simulink model "DYN_02x"  (R2021a)
(part 22 of 53)

(sin(e5)*(cos(e1)*cos(e2)*cos(e3) - cos(e1)*sin(e2)*sin(e3)) + cos(e5)*(sin(e1)*sin(e4) + cos(e4)*(cos(e1)*cos(e2)*sin(e3) + cos(e1)*cos(e3)*sin(e2))))*(z5*(cos(e2 + e3)*cos(e5) - sin(e2 + e3)*cos(e4)*sin(e5)) - y5*sin(e2 + e3)*sin(e4) + cos(e5)*sin(e4)*(a3*cos(e2 + e3) - d4*sin(e2 + e3) + a2*cos(e2))) - (cos(e5)*(cos(e1)*cos(e2)*cos(e3) - cos(e1)*sin(e2)*sin(e3)) - sin(e5)*(sin(e1)*sin(e4) + cos(e4)*(cos(e1)*cos(e2)*sin(e3) + cos(e1)*cos(e3)*sin(e2))))*(z5*(cos(e2 + e3)*sin(e5) + sin(e2 + e3)*cos(e4)*cos(e5)) - x5*sin(e2 + e3)*sin(e4) + sin(e4)*sin(e5)*(a3*cos(e2 + e3) - d4*sin(e2 + e3) + a2*cos(e2))) - (sin(e5)*(cos(e1)*cos(e2)*sin(e3) + cos(e1)*cos(e3)*sin(e2)) - cos(e4)*cos(e5)*(cos(e1)*cos(e2)*cos(e3) - cos(e1)*sin(e2)*sin(e3)))*(z5*(sin(e2 + e3)*cos(e5) + cos(e2 + e3)*cos(e4)*sin(e5)) + cos(e5)*sin(e4)*(a1 + d4*cos(e2 + e3) + a3*sin(e2 + e3) + a2*sin(e2)) + y5*cos(e2 + e3)*sin(e4)) - sin(e4)*(cos(e1)*cos(e2)*cos(e3) - cos(e1)*sin(e2)*sin(e3))*(cos(e4)*(a1 + d4*cos(e2 + e3) + a3*sin(e2 + e3) + a2*sin(e2)) + x5*(sin(e2 + e3)*cos(e5) + cos(e2 + e3)*cos(e4)*sin(e5)) - y5*(sin(e2 + e3)*sin(e5) - cos(e2 + e3)*cos(e4)*cos(e5)))) - m5*((cos(e5)*(sin(e2)*sin(e3) - cos(e2)*cos(e3)) + cos(e4)*sin(e5)*(cos(e2)*sin(e3) + cos(e3)*sin(e2)))*(a3*cos(e5) + x5*cos(e4) + d4*cos(e4)*sin(e5) + z5*cos(e5)*sin(e4)) + (sin(e5)*(sin(e2)*sin(e3) - cos(e2)*cos(e3)) - cos(e4)*cos(e5)*(cos(e2)*sin(e3) + cos(e3)*sin(e2)))*(a3*sin(e5) - y5*cos(e4) - d4*cos(e4)*cos(e5) + z5*sin(e4)*sin(e5)) + sin(e4)*(cos(e2)*sin(e3) + cos(e3)*sin(e2))*(d4*sin(e4) + y5*cos(e5)*sin(e4) + x5*sin(e4)*sin(e5)))*((cos(e5)*(cos(e2)*sin(e3) + cos(e3)*sin(e2)) - cos(e4)*sin(e5)*(sin(e2)*sin(e3) - cos(e2)*cos(e3)))*(z5*(sin(e2 + e3)*sin(e5) - cos(e2 + e3)*cos(e4)*cos(e5)) + sin(e4)*sin(e5)*(a1 + d4*cos(e2 + e3) + a3*sin(e2 + e3) + a2*sin(e2)) + x5*cos(e2 + e3)*sin(e4)) - (sin(e5)*(cos(e2)*sin(e3) + cos(e3)*sin(e2)) + cos(e4)*cos(e5)*(sin(e2)*sin(e3) - cos(e2)*cos(e3)))*(z5*(sin(e2 + e3)*cos(e5) + cos(e2 + e3)*cos(e4)*sin(e5)) + cos(e5)*sin(e4)*(a1 + d4*cos(e2 + e3) + a3*sin(e2 + e3) + a2*sin(e2)) + y5*cos(e2 + e3)*sin(e4)) + sin(e4)*(sin(e2)*sin(e3) - cos(e2)*cos(e3))*(cos(e4)*(a1 + d4*cos(e2 + e3) + a3*sin(e2 + e3) + a2*sin(e2)) + x5*(sin(e2 + e3)*cos(e5) + cos(e2 + e3)*cos(e4)*sin(e5)) - y5*(sin(e2 + e3)*sin(e5) - cos(e2 + e3)*cos(e4)*cos(e5)))) - (sin(e4)*sin(e5)*(I5xy*(cos(e2 + e3)*sin(e5) + sin(e2 + e3)*cos(e4)*cos(e5)) + I5yy*(cos(e2 + e3)*cos(e5) - sin(e2 + e3)*cos(e4)*sin(e5)) + I5zy*sin(e2 + e3)*sin(e4)))/2 + m5*((cos(e4)*sin(e1) - sin(e4)*(cos(e1)*cos(e2)*sin(e3) + cos(e1)*cos(e3)*sin(e2)))*(cos(e4)*(a1 + d4*cos(e2 + e3) + a3*sin(e2 + e3) + a2*sin(e2)) + x5*(sin(e2 + e3)*cos(e5) + cos(e2 + e3)*cos(e4)*sin(e5)) - y5*(sin(e2 + e3)*sin(e5) - cos(e2 + e3)*cos(e4)*cos(e5))) + (sin(e5)*(cos(e1)*cos(e2)*cos(e3) - cos(e1)*sin(e2)*sin(e3)) + cos(e5)*(sin(e1)*sin(e4) + cos(e4)*(cos(e1)*cos(e2)*sin(e3) + cos(e1)*cos(e3)*sin(e2))))*(z5*(sin(e2 + e3)*cos(e5) + cos(e2 + e3)*cos(e4)*sin(e5)) + cos(e5)*sin(e4)*(a1 + d4*cos(e2 + e3) + a3*sin(e2 + e3) + a2*sin(e2)) + y5*cos(e2 + e3)*sin(e4)) - (cos(e5)*(cos(e1)*cos(e2)*cos(e3) - cos(e1)*sin(e2)*sin(e3)) - sin(e5)*(sin(e1)*sin(e4) + cos(e4)*(cos(e1)*cos(e2)*sin(e3) + cos(e1)*cos(e3)*sin(e2))))*(z5*(sin(e2 + e3)*sin(e5) - cos(e2 + e3)*cos(e4)*cos(e5)) + sin(e4)*sin(e5)*(a1 + d4*cos(e2 + e3) + a3*sin(e2 + e3) + a2*sin(e2)) + x5*cos(e2 + e3)*sin(e4)))*((cos(e5)*(cos(e1)*cos(e2)*sin(e3) + cos(e1)*cos(e3)*sin(e2)) + cos(e4)*sin(e5)*(cos(e1)*cos(e2)*cos(e3) - cos(e1)*sin(e2)*sin(e3)))*(a3*cos(e5) + x5*cos(e4) + d4*cos(e4)*sin(e5) + z5*cos(e5)*sin(e4)) + (sin(e5)*(cos(e1)*cos(e2)*sin(e3) + cos(e1)*cos(e3)*sin(e2)) - cos(e4)*cos(e5)*(cos(e1)*cos(e2)*cos(e3) - cos(e1)*sin(e2)*sin(e3)))*(a3*sin(e5) - y5*cos(e4) - d4*cos(e4)*cos(e5) + z5*sin(e4)*sin(e5)) + sin(e4)*(cos(e1)*cos(e2)*cos(e3) - cos(e1)*sin(e2)*sin(e3))*(d4*sin(e4) + y5*cos(e5)*sin(e4) + x5*sin(e4)*sin(e5))) - (sin(e2 + e3)*sin(e4)*(I5zz*cos(e4) - I5xz*cos(e5)*sin(e4) + I5yz*sin(e4)*sin(e5)))/2 + m4*(cos(e4)*(sin(e2)*sin(e3) - cos(e2)*cos(e3))*(d4*cos(e4) + z4*cos(e4)) - (cos(e2)*sin(e3) + cos(e3)*sin(e2))*(a3 + x4*cos(e4) - y4*sin(e4)) + sin(e4)*(sin(e2)*sin(e3) - cos(e2)*cos(e3))*(d4*sin(e4) + z4*sin(e4)))*((sin(e2)*sin(e3) - cos(e2)*cos(e3))*(y4*cos(e2 + e3)*cos(e4) + x4*cos(e2 + e3)*sin(e4)) + (cos(e2)*sin(e3) + cos(e3)*sin(e2))*(y4*sin(e2 + e3)*cos(e4) + x4*sin(e2 + e3)*sin(e4)) - sin(e4)*(sin(e2)*sin(e3) - cos(e2)*cos(e3))*(x4*cos(e2 + e3) + cos(e4)*(a3*cos(e2 + e3) - d4*sin(e2 + e3) + a2*cos(e2)) - z4*sin(e2 + e3)*cos(e4)) - cos(e4)*(sin(e2)*sin(e3) - cos(e2)*cos(e3))*(y4*cos(e2 + e3) - sin(e4)*(a3*cos(e2 + e3) - d4*sin(e2 + e3) + a2*cos(e2)) + z4*sin(e2 + e3)*sin(e4)) - sin(e4)*(cos(e2)*sin(e3) + cos(e3)*sin(e2))*(cos(e4)*(a1 + d4*cos(e2 + e3) + a3*sin(e2 + e3) + a2*sin(e2)) + x4*sin(e2 + e3) + z4*cos(e2 + e3)*cos(e4)) + cos(e4)*(cos(e2)*sin(e3) + cos(e3)*sin(e2))*(sin(e4)*(a1 + d4*cos(e2 + e3) + a3*sin(e2 + e3) + a2*sin(e2)) - y4*sin(e2 + e3) + z4*cos(e2 + e3)*sin(e4))) - m5*((cos(e5)*(cos(e2)*sin(e1)*sin(e3) + cos(e3)*sin(e1)*sin(e2)) + cos(e4)*sin(e5)*(cos(e2)*cos(e3)*sin(e1) - sin(e1)*sin(e2)*sin(e3)))*(a3*cos(e5) + x5*cos(e4) + d4*cos(e4)*sin(e5) + z5*cos(e5)*sin(e4)) + (sin(e5)*(cos(e2)*sin(e1)*sin(e3) + cos(e3)*sin(e1)*sin(e2)) - cos(e4)*cos(e5)*(cos(e2)*cos(e3)*sin(e1) - sin(e1)*sin(e2)*sin(e3)))*(a3*sin(e5) - y5*cos(e4) - d4*cos(e4)*cos(e5) + z5*sin(e4)*sin(e5)) + sin(e4)*(cos(e2)*cos(e3)*sin(e1) - sin(e1)*sin(e2)*sin(e3))*(d4*sin(e4) + y5*cos(e5)*sin(e4) + x5*sin(e4)*sin(e5)))*((cos(e5)*(cos(e2)*cos(e3)*sin(e1) - sin(e1)*sin(e2)*sin(e3)) + sin(e5)*(cos(e1)*sin(e4) - cos(e4)*(cos(e2)*sin(e1)*sin(e3) + cos(e3)*sin(e1)*sin(e2))))*(z5*(sin(e2 + e3)*sin(e5) - cos(e2 + e3)*cos(e4)*cos(e5)) + sin(e4)*sin(e5)*(a1 + d4*cos(e2 + e3) + a3*sin(e2 + e3) + a2*sin(e2)) + x5*cos(e2 + e3)*sin(e4)) + (sin(e4)*(cos(e2)*sin(e1)*sin(e3) + cos(e3)*sin(e1)*sin(e2)) + cos(e1)*cos(e4))*(cos(e4)*(a1 + d4*cos(e2 + e3) + a3*sin(e2 + e3) + a2*sin(e2)) + x5*(sin(e2 + e3)*cos(e5) + cos(e2 + e3)*cos(e4)*sin(e5)) - y5*(sin(e2 + e3)*sin(e5) - cos(e2 + e3)*cos(e4)*cos(e5))) - (sin(e5)*(cos(e2)*cos(e3)*sin(e1) - sin(e1)*sin(e2)*sin(e3)) - cos(e5)*(cos(e1)*sin(e4) - cos(e4)*(cos(e2)*sin(e1)*sin(e3) + cos(e3)*sin(e1)*sin(e2))))*(z5*(sin(e2 + e3)*cos(e5) + cos(e2 + e3)*cos(e4)*sin(e5)) + cos(e5)*sin(e4)*(a1 + d4*cos(e2 + e3) + a3*sin(e2 + e3) + a2*sin(e2)) + y5*cos(e2 + e3)*sin(e4))) + m6*((sin(e6)*(sin(e5)*(cos(e2)*cos(e3)*sin(e1) - sin(e1)*sin(e2)*sin(e3)) - cos(e5)*(cos(e1)*sin(e4) - cos(e4)*(cos(e2)*sin(e1)*sin(e3) + cos(e3)*sin(e1)*sin(e2)))) + cos(e6)*(sin(e4)*(cos(e2)*sin(e1)*sin(e3) + cos(e3)*sin(e1)*sin(e2)) + cos(e1)*cos(e4)))*(z6*(cos(e4)*sin(e6) + cos(e5)*cos(e6)*sin(e4)) - sin(e6)*(a3*sin(e5) - d4*cos(e4)*cos(e5)) + d4*cos(e6)*sin(e4) + x6*sin(e4)*sin(e5)) - (cos(e5)*(cos(e2)*cos(e3)*sin(e1) - sin(e1)*sin(e2)*sin(e3)) + sin(e5)*(cos(e1)*sin(e4) - cos(e4)*(cos(e2)*sin(e1)*sin(e3) + cos(e3)*sin(e1)*sin(e2))))*(a3*cos(e5) - y6*(cos(e4)*sin(e6) + cos(e5)*cos(e6)*sin(e4)) + x6*(cos(e4)*cos(e6) - cos(e5)*sin(e4)*sin(e6)) + d4*cos(e4)*sin(e5)) + (cos(e6)*(sin(e5)*(cos(e2)*cos(e3)*sin(e1) - sin(e1)*sin(e2)*sin(e3)) - cos(e5)*(cos(e1)*sin(e4) - cos(e4)*(cos(e2)*sin(e1)*sin(e3) + cos(e3)*sin(e1)*sin(e2)))) - sin(e6)*(sin(e4)*(cos(e2)*sin(e1)*sin(e3) + cos(e3)*sin(e1)*sin(e2)) + cos(e1)*cos(e4)))*(z6*(cos(e4)*cos(e6) - cos(e5)*sin(e4)*sin(e6)) - cos(e6)*(a3*sin(e5) - d4*cos(e4)*cos(e5)) - d4*sin(e4)*sin(e6) + y6*sin(e4)*sin(e5)))*((sin(e6)*(sin(e5)*(cos(e2)*sin(e1)*sin(e3) + cos(e3)*sin(e1)*sin(e2)) - cos(e4)*cos(e5)*(cos(e2)*cos(e3)*sin(e1) - sin(e1)*sin(e2)*sin(e3))) - cos(e6)*sin(e4)*(cos(e2)*cos(e3)*sin(e1) - sin(e1)*sin(e2)*sin(e3)))*(x6*(sin(e2 + e3)*cos(e5) + cos(e2 + e3)*cos(e4)*sin(e5)) - z6*(cos(e6)*(sin(e2 + e3)*sin(e5) - cos(e2 + e3)*cos(e4)*cos(e5)) + cos(e2 + e3)*sin(e4)*sin(e6)) + cos(e4)*cos(e6)*(a1 + d4*cos(e2 + e3) + a3*sin(e2 + e3) + a2*sin(e2)) - cos(e5)*sin(e4)*sin(e6)*(a1 + d4*cos(e2 + e3) + a3*sin(e2 + e3) + a2*sin(e2))) + (cos(e6)*(sin(e5)*(cos(e2)*sin(e1)*sin(e3) + cos(e3)*sin(e1)*sin(e2)) - cos(e4)*cos(e5)*(cos(e2)*cos(e3)*sin(e1) - sin(e1)*sin(e2)*sin(e3))) + sin(e4)*sin(e6)*(cos(e2)*cos(e3)*sin(e1) - sin(e1)*sin(e2)*sin(e3)))*(y6*(sin(e2 + e3)*cos(e5) + cos(e2 + e3)*cos(e4)*sin(e5)) + z6*(sin(e6)*(sin(e2 + e3)*sin(e5) - cos(e2 + e3)*cos(e4)*cos(e5)) - cos(e2 + e3)*cos(e6)*sin(e4)) - cos(e4)*sin(e6)*(a1 + d4*cos(e2 + e3) + a3*sin(e2 + e3) + a2*sin(e2)) - cos(e5)*cos(e6)*sin(e4)*(a1 + d4*cos(e2 + e3) + a3*sin(e2 + e3) + a2*sin(e2))) + (cos(e5)*(cos(e2)*cos(e3)*sin(e1) - sin(e1)*sin(e2)*sin(e3)) + sin(e5)*(cos(e1)*sin(e4) - cos(e4)*(cos(e2)*sin(e1)*sin(e3) + cos(e3)*sin(e1)*sin(e2))))*(x6*(sin(e6)*(cos(e2 + e3)*sin(e5) + sin(e2 + e3)*cos(e4)*cos(e5)) + sin(e2 + e3)*cos(e6)*sin(e4)) + y6*(cos(e6)*(cos(e2 + e3)*sin(e5) + sin(e2 + e3)*cos(e4)*cos(e5)) - sin(e2 + e3)*sin(e4)*sin(e6)) - sin(e4)*sin(e5)*(a3*cos(e2 + e3) - d4*sin(e2 + e3) + a2*cos(e2))) - (sin(e6)*(sin(e5)*(cos(e2)*cos(e3)*sin(e1) - sin(e1)*sin(e2)*sin(e3)) - cos(e5)*(cos(e1)*sin(e4) - cos(e4)*(cos(e2)*sin(e1)*sin(e3) + cos(e3)*sin(e1)*sin(e2)))) + cos(e6)*(sin(e4)*(cos(e2)*sin(e1)*sin(e3) + cos(e3)*sin(e1)*sin(e2)) + cos(e1)*cos(e4)))*(x6*(cos(e2 + e3)*cos(e5) - sin(e2 + e3)*cos(e4)*sin(e5)) - z6*(cos(e6)*(cos(e2 + e3)*sin(e5) + sin(e2 + e3)*cos(e4)*cos(e5)) - sin(e2 + e3)*sin(e4)*sin(e6)) + cos(e4)*cos(e6)*(a3*cos(e2 + e3) - d4*sin(e2 + e3) + a2*cos(e2)) - cos(e5)*sin(e4)*sin(e6)*(a3*cos(e2 + e3) - d4*sin(e2 + e3) + a2*cos(e2))) - (cos(e6)*(sin(e5)*(cos(e2)*cos(e3)*sin(e1) - sin(e1)*sin(e2)*sin(e3)) - cos(e5)*(cos(e1)*sin(e4) - cos(e4)*(cos(e2)*sin(e1)*sin(e3) + cos(e3)*sin(e1)*sin(e2)))) - sin(e6)*(sin(e4)*(cos(e2)*sin(e1)*sin(e3) + cos(e3)*sin(e1)*sin(e2)) + cos(e1)*cos(e4)))*(y6*(cos(e2 + e3)*cos(e5) - sin(e2 + e3)*cos(e4)*sin(e5)) + z6*(sin(e6)*(cos(e2 + e3)*sin(e5) + sin(e2 + e3)*cos(e4)*cos(e5)) + sin(e2 + e3)*cos(e6)*sin(e4)) - cos(e4)*sin(e6)*(a3*cos(e2 + e3) - d4*sin(e2 + e3) + a2*cos(e2)) - cos(e5)*cos(e6)*sin(e4)*(a3*cos(e2 + e3) - d4*sin(e2 + e3) + a2*cos(e2))) - (cos(e5)*(cos(e2)*sin(e1)*sin(e3) + cos(e3)*sin(e1)*sin(e2)) + cos(e4)*sin(e5)*(cos(e2)*cos(e3)*sin(e1) - sin(e1)*sin(e2)*sin(e3)))*(x6*(sin(e6)*(sin(e2 + e3)*sin(e5) - cos(e2 + e3)*cos(e4)*cos(e5)) - cos(e2 + e3)*cos(e6)*sin(e4)) + y6*(cos(e6)*(sin(e2 + e3)*sin(e5) - cos(e2 + e3)*cos(e4)*cos(e5)) + cos(e2 + e3)*sin(e4)*sin(e6)) - sin(e4)*sin(e5)*(a1 + d4*cos(e2 + e3) + a3*sin(e2 + e3) + a2*sin(e2)))) - m4*((cos(e2)*cos(e3)*sin(e1) - sin(e1)*sin(e2)*sin(e3))*(a3 + x4*cos(e4) - y4*sin(e4)) + (d4*cos(e4) + z4*cos(e4))*(cos(e1)*sin(e4) - cos(e4)*(cos(e2)*sin(e1)*sin(e3) + cos(e3)*sin(e1)*sin(e2))) - (sin(e4)*(cos(e2)*sin(e1)*sin(e3) + cos(e3)*sin(e1)*sin(e2)) + cos(e1)*cos(e4))*(d4*sin(e4) + z4*sin(e4)))*((cos(e2)*sin(e1)*sin(e3) + cos(e3)*sin(e1)*sin(e2))*(y4*cos(e2 + e3)*cos(e4) + x4*cos(e2 + e3)*sin(e4)) + (cos(e2)*cos(e3)*sin(e1) - sin(e1)*sin(e2)*sin(e3))*(y4*sin(e2 + e3)*cos(e4) + x4*sin(e2 + e3)*sin(e4)) - (sin(e4)*(cos(e2)*sin(e1)*sin(e3) + cos(e3)*sin(e1)*sin(e2)) + cos(e1)*cos(e4))*(x4*cos(e2 + e3) + cos(e4)*(a3*cos(e2 + e3) - d4*sin(e2 + e3) + a2*cos(e2)) - z4*sin(e2 + e3)*cos(e4)) + (cos(e1)*sin(e4) - cos(e4)*(cos(e2)*sin(e1)*sin(e3) + cos(e3)*sin(e1)*sin(e2)))*(y4*cos(e2 + e3) - sin(e4)*(a3*cos(e2 + e3) - d4*sin(e2 + e3) + a2*cos(e2)) + z4*sin(e2 + e3)*sin(e4)) - sin(e4)*(cos(e2)*cos(e3)*sin(e1) - sin(e1)*sin(e2)*sin(e3))*(cos(e4)*(a1 + d4*cos(e2 + e3) + a3*sin(e2 + e3) + a2*sin(e2)) + x4*sin(e2 + e3) + z4*cos(e2 + e3)*cos(e4)) + cos(e4)*(cos(e2)*cos(e3)*sin(e1) - sin(e1)*sin(e2)*sin(e3))*(sin(e4)*(a1 + d4*cos(e2 + e3) + a3*sin(e2 + e3) + a2*sin(e2)) - y4*sin(e2 + e3) + z4*cos(e2 + e3)*sin(e4))) - m4*((sin(e4)*(cos(e2)*sin(e1)*sin(e3) + cos(e3)*sin(e1)*sin(e2)) + cos(e1)*cos(e4))*(cos(e4)*(a1 + d4*cos(e2 + e3) + a3*sin(e2 + e3) + a2*sin(e2)) + x4*sin(e2 + e3) + z4*cos(e2 + e3)*cos(e4)) + (cos(e2)*cos(e3)*sin(e1) - sin(e1)*sin(e2)*sin(e3))*(y4*cos(e2 + e3)*cos(e4) + x4*cos(e2 + e3)*sin(e4)) + (cos(e1)*sin(e4) - cos(e4)*(cos(e2)*sin(e1)*sin(e3) + cos(e3)*sin(e1)*sin(e2)))*(sin(e4)*(a1 + d4*cos(e2 + e3) + a3*sin(e2 + e3) + a2*sin(e2)) - y4*sin(e2 + e3) + z4*cos(e2 + e3)*sin(e4)))*((cos(e2)*sin(e1)*sin(e3) + cos(e3)*sin(e1)*sin(e2))*(a3 + x4*cos(e4) - y4*sin(e4)) + cos(e4)*(cos(e2)*cos(e3)*sin(e1) - sin(e1)*sin(e2)*sin(e3))*(d4*cos(e4) + z4*cos(e4)) + sin(e4)*(cos(e2)*cos(e3)*sin(e1) - sin(e1)*sin(e2)*sin(e3))*(d4*sin(e4) + z4*sin(e4))) - m4*((cos(e1)*cos(e2)*cos(e3) - cos(e1)*sin(e2)*sin(e3))*(a3 + x4*cos(e4) - y4*sin(e4)) - (sin(e1)*sin(e4) + cos(e4)*(cos(e1)*cos(e2)*sin(e3) + cos(e1)*cos(e3)*sin(e2)))*(d4*cos(e4) + z4*cos(e4)) + (cos(e4)*sin(e1) - sin(e4)*(cos(e1)*cos(e2)*sin(e3) + cos(e1)*cos(e3)*sin(e2)))*(d4*sin(e4) + z4*sin(e4)))*((y4*cos(e2 + e3)*cos(e4) + x4*cos(e2 + e3)*sin(e4))*(cos(e1)*cos(e2)*sin(e3) + cos(e1)*cos(e3)*sin(e2)) + (y4*sin(e2 + e3)*cos(e4) + x4*sin(e2 + e3)*sin(e4))*(cos(e1)*cos(e2)*cos(e3) - cos(e1)*sin(e2)*sin(e3)) + (cos(e4)*sin(e1) - sin(e4)*(cos(e1)*cos(e2)*sin(e3) + cos(e1)*cos(e3)*sin(e2)))*(x4*cos(e2 + e3) + cos(e4)*(a3*cos(e2 + e3) - d4*sin(e2 + e3) + a2*cos(e2)) - z4*sin(e2 + e3)*cos(e4)) - (sin(e1)*sin(e4) + cos(e4)*(cos(e1)*cos(e2)*sin(e3) + cos(e1)*cos(e3)*sin(e2)))*(y4*cos(e2 + e3) - sin(e4)*(a3*cos(e2 + e3) - d4*sin(e2 + e3) + a2*cos(e2)) + z4*sin(e2 + e3)*sin(e4)) - sin(e4)*(cos(e1)*cos(e2)*cos(e3) - cos(e1)*sin(e2)*sin(e3))*(cos(e4)*(a1 + d4*cos(e2 + e3) + a3*sin(e2 + e3) + a2*sin(e2)) + x4*sin(e2 + e3) + z4*cos(e2 + e3)*cos(e4)) + cos(e4)*(cos(e1)*cos(e2)*cos(e3) - cos(e1)*sin(e2)*sin(e3))*(sin(e4)*(a1 + d4*cos(e2 + e3) + a3*sin(e2 + e3) + a2*sin(e2)) - y4*sin(e2 + e3) + z4*cos(e2 + e3)*sin(e4))) + m3*(y3*cos(e2 + e3)*cos(e1) + x3*sin(e2 + e3)*cos(e1))*(sin(e1)*(a1 + y3*cos(e2 + e3) + x3*sin(e2 + e3) + a2*sin(e2)) + z3*cos(e2 + e3)^2*cos(e1) + z3*sin(e2 + e3)^2*cos(e1)) + m6*((sin(e6)*(sin(e5)*(cos(e2)*sin(e3) + cos(e3)*sin(e2)) + cos(e4)*cos(e5)*(sin(e2)*sin(e3) - cos(e2)*cos(e3))) + cos(e6)*sin(e4)*(sin(e2)*sin(e3) - cos(e2)*cos(e3)))*(z6*(cos(e4)*sin(e6) + cos(e5)*cos(e6)*sin(e4)) - sin(e6)*(a3*sin(e5) - d4*cos(e4)*cos(e5)) + d4*cos(e6)*sin(e4) + x6*sin(e4)*sin(e5)) + (cos(e6)*(sin(e5)*(cos(e2)*sin(e3) + cos(e3)*sin(e2)) + cos(e4)*cos(e5)*(sin(e2)*sin(e3) - cos(e2)*cos(e3))) - sin(e4)*sin(e6)*(sin(e2)*sin(e3) - cos(e2)*cos(e3)))*(z6*(cos(e4)*cos(e6) - cos(e5)*sin(e4)*sin(e6)) - cos(e6)*(a3*sin(e5) - d4*cos(e4)*cos(e5)) - d4*sin(e4)*sin(e6) + y6*sin(e4)*sin(e5)) - (cos(e5)*(cos(e2)*sin(e3) + cos(e3)*sin(e2)) - cos(e4)*sin(e5)*(sin(e2)*sin(e3) - cos(e2)*cos(e3)))*(a3*cos(e5) - y6*(cos(e4)*sin(e6) + cos(e5)*cos(e6)*sin(e4)) + x6*(cos(e4)*cos(e6) - cos(e5)*sin(e4)*sin(e6)) + d4*cos(e4)*sin(e5)))*((sin(e6)*(sin(e5)*(sin(e2)*sin(e3) - cos(e2)*cos(e3)) - cos(e4)*cos(e5)*(cos(e2)*sin(e3) + cos(e3)*sin(e2))) - cos(e6)*sin(e4)*(cos(e2)*sin(e3) + cos(e3)*sin(e2)))*(x6*(sin(e2 + e3)*cos(e5) + cos(e2 + e3)*cos(e4)*sin(e5)) - z6*(cos(e6)*(sin(e2 + e3)*sin(e5) - cos(e2 + e3)*cos(e4)*cos(e5)) + cos(e2 + e3)*sin(e4)*sin(e6)) + cos(e4)*cos(e6)*(a1 + d4*cos(e2 + e3) + a3*sin(e2 + e3) + a2*sin(e2)) - cos(e5)*sin(e4)*sin(e6)*(a1 + d4*cos(e2 + e3) + a3*sin(e2 + e3) + a2*sin(e2))) + (cos(e6)*(sin(e5)*(sin(e2)*sin(e3) - cos(e2)*cos(e3)) - cos(e4)*cos(e5)*(cos(e2)*sin(e3) + cos(e3)*sin(e2))) + sin(e4)*sin(e6)*(cos(e2)*sin(e3) + cos(e3)*sin(e2)))*(y6*(sin(e2 + e3)*cos(e5) + cos(e2 + e3)*cos(e4)*sin(e5)) + z6*(sin(e6)*(sin(e2 + e3)*sin(e5) - cos(e2 + e3)*cos(e4)*cos(e5)) - cos(e2 + e3)*cos(e6)*sin(e4)) - cos(e4)*sin(e6)*(a1 + d4*cos(e2 + e3) + a3*sin(e2 + e3) + a2*sin(e2)) - cos(e5)*cos(e6)*sin(e4)*(a1 + d4*cos(e2 + e3) + a3*sin(e2 + e3) + a2*sin(e2))) + (cos(e5)*(cos(e2)*sin(e3) + cos(e3)*sin(e2)) - cos(e4)*sin(e5)*(sin(e2)*sin(e3) - cos(e2)*cos(e3)))*(x6*(sin(e6)*(cos(e2 + e3)*sin(e5) + sin(e2 + e3)*cos(e4)*cos(e5)) + sin(e2 + e3)*cos(e6)*sin(e4)) + y6*(cos(e6)*(cos(e2 + e3)*sin(e5) + sin(e2 + e3)*cos(e4)*cos(e5)) - sin(e2 + e3)*sin(e4)*sin(e6)) - sin(e4)*sin(e5)*(a3*cos(e2 + e3) - d4*sin(e2 + e3) + a2*cos(e2))) - (sin(e6)*(sin(e5)*(cos(e2)*sin(e3) + cos(e3)*sin(e2)) + cos(e4)*cos(e5)*(sin(e2)*sin(e3) - cos(e2)*cos(e3))) + cos(e6)*sin(e4)*(sin(e2)*sin(e3) - cos(e2)*cos(e3)))*(x6*(cos(e2 + e3)*cos(e5) - sin(e2 + e3)*cos(e4)*sin(e5)) - z6*(cos(e6)*(cos(e2 + e3)*sin(e5) + sin(e2 + e3)*cos(e4)*cos(e5)) - sin(e2 + e3)*sin(e4)*sin(e6)) + cos(e4)*cos(e6)*(a3*cos(e2 + e3) - d4*sin(e2 + e3) + a2*cos(e2)) - cos(e5)*sin(e4)*sin(e6)*(a3*cos(e2 + e3) - d4*sin(e2 + e3) + a2*cos(e2))) - (cos(e6)*(sin(e5)*(cos(e2)*sin(e3) + cos(e3)*sin(e2)) + cos(e4)*cos(e5)*(sin(e2)*sin(e3) - cos(e2)*cos(e3))) - sin(e4)*sin(e6)*(sin(e2)*sin(e3) - cos(e2)*cos(e3)))*(y6*(cos(e2 + e3)*cos(e5) - sin(e2 + e3)*cos(e4)*sin(e5)) + z6*(sin(e6)*(cos(e2 + e3)*sin(e5) + sin(e2 + e3)*cos(e4)*cos(e5)) + sin(e2 + e3)*cos(e6)*sin(e4)) - cos(e4)*sin(e6)*(a3*cos(e2 + e3) - d4*sin(e2 + e3) + a2*cos(e2)) - cos(e5)*cos(e6)*sin(e4)*(a3*cos(e2 + e3) - d4*sin(e2 + e3) + a2*cos(e2))) - (cos(e5)*(sin(e2)*sin(e3) - cos(e2)*cos(e3)) + cos(e4)*sin(e5)*(cos(e2)*sin(e3) + cos(e3)*sin(e2)))*(x6*(sin(e6)*(sin(e2 + e3)*sin(e5) - cos(e2 + e3)*cos(e4)*cos(e5)) - cos(e2 + e3)*cos(e6)*sin(e4)) + y6*(cos(e6)*(sin(e2 + e3)*sin(e5) - cos(e2 + e3)*cos(e4)*cos(e5)) + cos(e2 + e3)*sin(e4)*sin(e6)) - sin(e4)*sin(e5)*(a1 + d4*cos(e2 + e3) + a3*sin(e2 + e3) + a2*sin(e2)))) + m6*((sin(e6)*(sin(e5)*(cos(e2)*cos(e3)*sin(e1) - sin(e1)*sin(e2)*sin(e3)) - cos(e5)*(cos(e1)*sin(e4) - cos(e4)*(cos(e2)*sin(e1)*sin(e3) + cos(e3)*sin(e1)*sin(e2)))) + cos(e6)*(sin(e4)*(cos(e2)*sin(e1)*sin(e3) + cos(e3)*sin(e1)*sin(e2)) + cos(e1)*cos(e4)))*(x6*(sin(e2 + e3)*cos(e5) + cos(e2 + e3)*cos(e4)*sin(e5)) - z6*(cos(e6)*(sin(e2 + e3)*sin(e5) - cos(e2 + e3)*cos(e4)*cos(e5)) + cos(e2 + e3)*sin(e4)*sin(e6)) + cos(e4)*cos(e6)*(a1 + d4*cos(e2 + e3) + a3*sin(e2 + e3) + a2*sin(e2)) - cos(e5)*sin(e4)*sin(e6)*(a1 + d4*cos(e2 + e3) + a3*sin(e2 + e3) + a2*sin(e2))) + (cos(e6)*(sin(e5)*(cos(e2)*cos(e3)*sin(e1) - sin(e1)*sin(e2)*sin(e3)) - cos(e5)*(cos(e1)*sin(e4) - cos(e4)*(cos(e2)*sin(e1)*sin(e3) + cos(e3)*sin(e1)*sin(e2)))) - sin(e6)*(sin(e4)*(cos(e2)*sin(e1)*sin(e3) + cos(e3)*sin(e1)*sin(e2)) + cos(e1)*cos(e4)))*(y6*(sin(e2 + e3)*cos(e5) + cos(e2 + e3)*cos(e4)*sin(e5)) + z6*(sin(e6)*(sin(e2 + e3)*sin(e5) - cos(e2 + e3)*cos(e4)*cos(e5)) - cos(e2 + e3)*cos(e6)*sin(e4)) - cos(e4)*sin(e6)*(a1 + d4*cos(e2 + e3) + a3*sin(e2 + e3) + a2*sin(e2)) - cos(e5)*cos(e6)*sin(e4)*(a1 + d4*cos(e2 + e3) + a3*sin(e2 + e3) + a2*sin(e2))) - (cos(e5)*(cos(e2)*cos(e3)*sin(e1) - sin(e1)*sin(e2)*sin(e3)) + sin(e5)*(cos(e1)*sin(e4) - cos(e4)*(cos(e2)*sin(e1)*sin(e3) + cos(e3)*sin(e1)*sin(e2))))*(x6*(sin(e6)*(sin(e2 + e3)*sin(e5) - cos(e2 + e3)*cos(e4)*cos(e5)) - cos(e2 + e3)*cos(e6)*sin(e4)) + y6*(cos(e6)*(sin(e2 + e3)*sin(e5) - cos(e2 + e3)*cos(e4)*cos(e5)) + cos(e2 + e3)*sin(e4)*sin(e6)) - sin(e4)*sin(e5)*(a1 + d4*cos(e2 + e3) + a3*sin(e2 + e3) + a2*sin(e2))))*((sin(e6)*(sin(e5)*(cos(e2)*sin(e1)*sin(e3) + cos(e3)*sin(e1)*sin(e2)) - cos(e4)*cos(e5)*(cos(e2)*cos(e3)*sin(e1) - sin(e1)*sin(e2)*sin(e3))) - cos(e6)*sin(e4)*(cos(e2)*cos(e3)*sin(e1) - sin(e1)*sin(e2)*sin(e3)))*(z6*(cos(e4)*sin(e6) + cos(e5)*cos(e6)*sin(e4)) - sin(e6)*(a3*sin(e5) - d4*cos(e4)*cos(e5)) + d4*cos(e6)*sin(e4) + x6*sin(e4)*sin(e5)) - (cos(e5)*(cos(e2)*sin(e1)*sin(e3) + cos(e3)*sin(e1)*sin(e2)) + cos(e4)*sin(e5)*(cos(e2)*cos(e3)*sin(e1) - sin(e1)*sin(e2)*sin(e3)))*(a3*cos(e5) - y6*(cos(e4)*sin(e6) + cos(e5)*cos(e6)*sin(e4)) + x6*(cos(e4)*cos(e6) - cos(e5)*sin(e4)*sin(e6)) + d4*cos(e4)*sin(e5)) + (cos(e6)*(sin(e5)*(cos(e2)*sin(e1)*sin(e3) + cos(e3)*sin(e1)*sin(e2)) - cos(e4)*cos(e5)*(cos(e2)*cos(e3)*sin(e1) - sin(e1)*sin(e2)*sin(e3))) + sin(e4)*sin(e6)*(cos(e2)*cos(e3)*sin(e1) - sin(e1)*sin(e2)*sin(e3)))*(z6*(cos(e4)*cos(e6) - cos(e5)*sin(e4)*sin(e6)) - cos(e6)*(a3*sin(e5) - d4*cos(e4)*cos(e5)) - d4*sin(e4)*sin(e6) + y6*sin(e4)*sin(e5))) + m5*((cos(e5)*(cos(e2)*cos(e3)*sin(e1) - sin(e1)*sin(e2)*sin(e3)) + sin(e5)*(cos(e1)*sin(e4) - cos(e4)*(cos(e2)*sin(e1)*sin(e3) + cos(e3)*sin(e1)*sin(e2))))*(a3*cos(e5) + x5*cos(e4) + d4*cos(e4)*sin(e5) + z5*cos(e5)*sin(e4)) + (sin(e5)*(cos(e2)*cos(e3)*sin(e1) - sin(e1)*sin(e2)*sin(e3)) - cos(e5)*(cos(e1)*sin(e4) - cos(e4)*(cos(e2)*sin(e1)*sin(e3) + cos(e3)*sin(e1)*sin(e2))))*(a3*sin(e5) - y5*cos(e4) - d4*cos(e4)*cos(e5) + z5*sin(e4)*sin(e5)) - (sin(e4)*(cos(e2)*sin(e1)*sin(e3) + cos(e3)*sin(e1)*sin(e2)) + cos(e1)*cos(e4))*(d4*sin(e4) + y5*cos(e5)*sin(e4) + x5*sin(e4)*sin(e5)))*((sin(e4)*(cos(e2)*sin(e1)*sin(e3) + cos(e3)*sin(e1)*sin(e2)) + cos(e1)*cos(e4))*(x5*(cos(e2 + e3)*cos(e5) - sin(e2 + e3)*cos(e4)*sin(e5)) - y5*(cos(e2 + e3)*sin(e5) + sin(e2 + e3)*cos(e4)*cos(e5)) + cos(e4)*(a3*cos(e2 + e3) - d4*sin(e2 + e3) + a2*cos(e2))) + (sin(e5)*(cos(e2)*sin(e1)*sin(e3) + cos(e3)*sin(e1)*sin(e2)) - cos(e4)*cos(e5)*(cos(e2)*cos(e3)*sin(e1) - sin(e1)*sin(e2)*sin(e3)))*(z5*(sin(e2 + e3)*cos(e5) + cos(e2 + e3)*cos(e4)*sin(e5)) + cos(e5)*sin(e4)*(a1 + d4*cos(e2 + e3) + a3*sin(e2 + e3) + a2*sin(e2)) + y5*cos(e2 + e3)*sin(e4)) - (cos(e5)*(cos(e2)*sin(e1)*sin(e3) + cos(e3)*sin(e1)*sin(e2)) + cos(e4)*sin(e5)*(cos(e2)*cos(e3)*sin(e1) - sin(e1)*sin(e2)*sin(e3)))*(z5*(sin(e2 + e3)*sin(e5) - cos(e2 + e3)*cos(e4)*cos(e5)) + sin(e4)*sin(e5)*(a1 + d4*cos(e2 + e3) + a3*sin(e2 + e3) + a2*sin(e2)) + x5*cos(e2 + e3)*sin(e4)) - (sin(e5)*(cos(e2)*cos(e3)*sin(e1) - sin(e1)*sin(e2)*sin(e3)) - cos(e5)*(cos(e1)*sin(e4) - cos(e4)*(cos(e2)*sin(e1)*sin(e3) + cos(e3)*sin(e1)*sin(e2))))*(z5*(cos(e2 + e3)*cos(e5) - sin(e2 + e3)*cos(e4)*sin(e5)) - y5*sin(e2 + e3)*sin(e4) + cos(e5)*sin(e4)*(a3*cos(e2 + e3) - d4*sin(e2 + e3) + a2*cos(e2))) + (cos(e5)*(cos(e2)*cos(e3)*sin(e1) - sin(e1)*sin(e2)*sin(e3)) + sin(e5)*(cos(e1)*sin(e4) - cos(e4)*(cos(e2)*sin(e1)*sin(e3) + cos(e3)*sin(e1)*sin(e2))))*(z5*(cos(e2 + e3)*sin(e5) + sin(e2 + e3)*cos(e4)*cos(e5)) - x5*sin(e2 + e3)*sin(e4) + sin(e4)*sin(e5)*(a3*cos(e2 + e3) - d4*sin(e2 + e3) + a2*cos(e2))) + sin(e4)*(cos(e2)*cos(e3)*sin(e1) - sin(e1)*sin(e2)*sin(e3))*(cos(e4)*(a1 + d4*cos(e2 + e3) + a3*sin(e2 + e3) + a2*sin(e2)) + x5*(sin(e2 + e3)*cos(e5) + cos(e2 + e3)*cos(e4)*sin(e5)) - y5*(sin(e2 + e3)*sin(e5) - cos(e2 + e3)*cos(e4)*cos(e5)))) + m3*(y3*cos(e2 + e3)*sin(e1) + x3*sin(e2 + e3)*sin(e1))*(z3*cos(e2 + e3)^2*sin(e1) - cos(e1)*(a1 + y3*cos(e2 + e3) + x3*sin(e2 + e3) + a2*sin(e2)) + z3*sin(e2 + e3)^2*sin(e1)) + m4*((cos(e1)*cos(e2)*sin(e3) + cos(e1)*cos(e3)*sin(e2))*(a3 + x4*cos(e4) - y4*sin(e4)) + cos(e4)*(d4*cos(e4) + z4*cos(e4))*(cos(e1)*cos(e2)*cos(e3) - cos(e1)*sin(e2)*sin(e3)) + sin(e4)*(d4*sin(e4) + z4*sin(e4))*(cos(e1)*cos(e2)*cos(e3) - cos(e1)*sin(e2)*sin(e3)))*((cos(e4)*sin(e1) - sin(e4)*(cos(e1)*cos(e2)*sin(e3) + cos(e1)*cos(e3)*sin(e2)))*(cos(e4)*(a1 + d4*cos(e2 + e3) + a3*sin(e2 + e3) + a2*sin(e2)) + x4*sin(e2 + e3) + z4*cos(e2 + e3)*cos(e4)) - (y4*cos(e2 + e3)*cos(e4) + x4*cos(e2 + e3)*sin(e4))*(cos(e1)*cos(e2)*cos(e3) - cos(e1)*sin(e2)*sin(e3)) + (sin(e1)*sin(e4) + cos(e4)*(cos(e1)*cos(e2)*sin(e3) + cos(e1)*cos(e3)*sin(e2)))*(sin(e4)*(a1 + d4*cos(e2 + e3) + a3*sin(e2 + e3) + a2*sin(e2)) - y4*sin(e2 + e3) + z4*cos(e2 + e3)*sin(e4))) - m4*((sin(e2)*sin(e3) - cos(e2)*cos(e3))*(a3 + x4*cos(e4) - y4*sin(e4)) + cos(e4)*(cos(e2)*sin(e3) + cos(e3)*sin(e2))*(d4*cos(e4) + z4*cos(e4)) + sin(e4)*(cos(e2)*sin(e3) + cos(e3)*sin(e2))*(d4*sin(e4) + z4*sin(e4)))*((cos(e2)*sin(e3) + cos(e3)*sin(e2))*(y4*cos(e2 + e3)*cos(e4) + x4*cos(e2 + e3)*sin(e4)) + sin(e4)*(sin(e2)*sin(e3) - cos(e2)*cos(e3))*(cos(e4)*(a1 + d4*cos(e2 + e3) + a3*sin(e2 + e3) + a2*sin(e2)) + x4*sin(e2 + e3) + z4*cos(e2 + e3)*cos(e4)) - cos(e4)*(sin(e2)*sin(e3) - cos(e2)*cos(e3))*(sin(e4)*(a1 + d4*cos(e2 + e3) + a3*sin(e2 + e3) + a2*sin(e2)) - y4*sin(e2 + e3) + z4*cos(e2 + e3)*sin(e4))) - (sin(e4)*sin(e5)*(I6zz*(cos(e2 + e3)*cos(e5) - sin(e2 + e3)*cos(e4)*sin(e5)) + I6xz*(cos(e6)*(cos(e2 + e3)*sin(e5) + sin(e2 + e3)*cos(e4)*cos(e5)) - sin(e2 + e3)*sin(e4)*sin(e6)) - I6yz*(sin(e6)*(cos(e2 + e3)*sin(e5) + sin(e2 + e3)*cos(e4)*cos(e5)) + sin(e2 + e3)*cos(e6)*sin(e4))))/2 + m6*((sin(e6)*(sin(e5)*(cos(e1)*cos(e2)*cos(e3) - cos(e1)*sin(e2)*sin(e3)) + cos(e5)*(sin(e1)*sin(e4) + cos(e4)*(cos(e1)*cos(e2)*sin(e3) + cos(e1)*cos(e3)*sin(e2)))) - cos(e6)*(cos(e4)*sin(e1) - sin(e4)*(cos(e1)*cos(e2)*sin(e3) + cos(e1)*cos(e3)*sin(e2))))*(x6*(sin(e2 + e3)*cos(e5) + cos(e2 + e3)*cos(e4)*sin(e5)) - z6*(cos(e6)*(sin(e2 + e3)*sin(e5) - cos(e2 + e3)*cos(e4)*cos(e5)) + cos(e2 + e3)*sin(e4)*sin(e6)) + cos(e4)*cos(e6)*(a1 + d4*cos(e2 + e3) + a3*sin(e2 + e3) + a2*sin(e2)) - cos(e5)*sin(e4)*sin(e6)*(a1 + d4*cos(e2 + e3) + a3*sin(e2 + e3) + a2*sin(e2))) + (cos(e6)*(sin(e5)*(cos(e1)*cos(e2)*cos(e3) - cos(e1)*sin(e2)*sin(e3)) + cos(e5)*(sin(e1)*sin(e4) + cos(e4)*(cos(e1)*cos(e2)*sin(e3) + cos(e1)*cos(e3)*sin(e2)))) + sin(e6)*(cos(e4)*sin(e1) - sin(e4)*(cos(e1)*cos(e2)*sin(e3) + cos(e1)*cos(e3)*sin(e2))))*(y6*(sin(e2 + e3)*cos(e5) + cos(e2 + e3)*cos(e4)*sin(e5)) + z6*(sin(e6)*(sin(e2 + e3)*sin(e5) - cos(e2 + e3)*cos(e4)*cos(e5)) - cos(e2 + e3)*cos(e6)*sin(e4)) - cos(e4)*sin(e6)*(a1 + d4*cos(e2 + e3) + a3*sin(e2 + e3) + a2*sin(e2)) - cos(e5)*cos(e6)*sin(e4)*(a1 + d4*cos(e2 + e3) + a3*sin(e2 + e3) + a2*sin(e2))) - (cos(e5)*(cos(e1)*cos(e2)*cos(e3) - cos(e1)*sin(e2)*sin(e3)) - sin(e5)*(sin(e1)*sin(e4) + cos(e4)*(cos(e1)*cos(e2)*sin(e3) + cos(e1)*cos(e3)*sin(e2))))*(x6*(sin(e6)*(sin(e2 + e3)*sin(e5) - cos(e2 + e3)*cos(e4)*cos(e5)) - cos(e2 + e3)*cos(e6)*sin(e4)) + y6*(cos(e6)*(sin(e2 + e3)*sin(e5) - cos(e2 + e3)*cos(e4)*cos(e5)) + cos(e2 + e3)*sin(e4)*sin(e6)) - sin(e4)*sin(e5)*(a1 + d4*cos(e2 + e3) + a3*sin(e2 + e3) + a2*sin(e2))))*((sin(e6)*(sin(e5)*(cos(e1)*cos(e2)*sin(e3) + cos(e1)*cos(e3)*sin(e2)) - cos(e4)*cos(e5)*(cos(e1)*cos(e2)*cos(e3) - cos(e1)*sin(e2)*sin(e3))) - cos(e6)*sin(e4)*(cos(e1)*cos(e2)*cos(e3) - cos(e1)*sin(e2)*sin(e3)))*(z6*(cos(e4)*sin(e6) + cos(e5)*cos(e6)*sin(e4)) - sin(e6)*(a3*sin(e5) - d4*cos(e4)*cos(e5)) + d4*cos(e6)*sin(e4) + x6*sin(e4)*sin(e5)) - (cos(e5)*(cos(e1)*cos(e2)*sin(e3) + cos(e1)*cos(e3)*sin(e2)) + cos(e4)*sin(e5)*(cos(e1)*cos(e2)*cos(e3) - cos(e1)*sin(e2)*sin(e3)))*(a3*cos(e5) - y6*(cos(e4)*sin(e6) + cos(e5)*cos(e6)*sin(e4)) + x6*(cos(e4)*cos(e6) - cos(e5)*sin(e4)*sin(e6)) + d4*cos(e4)*sin(e5)) + (cos(e6)*(sin(e5)*(cos(e1)*cos(e2)*sin(e3) + cos(e1)*cos(e3)*sin(e2)) - cos(e4)*cos(e5)*(cos(e1)*cos(e2)*cos(e3) - cos(e1)*sin(e2)*sin(e3))) + sin(e4)*sin(e6)*(cos(e1)*cos(e2)*cos(e3) - cos(e1)*sin(e2)*sin(e3)))*(z6*(cos(e4)*cos(e6) - cos(e5)*sin(e4)*sin(e6)) - cos(e6)*(a3*sin(e5) - d4*cos(e4)*cos(e5)) - d4*sin(e4)*sin(e6) + y6*sin(e4)*sin(e5))) + m6*((sin(e6)*(sin(e5)*(sin(e2)*sin(e3) - cos(e2)*cos(e3)) - cos(e4)*cos(e5)*(cos(e2)*sin(e3) + cos(e3)*sin(e2))) - cos(e6)*sin(e4)*(cos(e2)*sin(e3) + cos(e3)*sin(e2)))*(z6*(cos(e4)*sin(e6) + cos(e5)*cos(e6)*sin(e4)) - sin(e6)*(a3*sin(e5) - d4*cos(e4)*cos(e5)) + d4*cos(e6)*sin(e4) + x6*sin(e4)*sin(e5)) + (cos(e6)*(sin(e5)*(sin(e2)*sin(e3) - cos(e2)*cos(e3)) - cos(e4)*cos(e5)*(cos(e2)*sin(e3) + cos(e3)*sin(e2))) + sin(e4)*sin(e6)*(cos(e2)*sin(e3) + cos(e3)*sin(e2)))*(z6*(cos(e4)*cos(e6) - cos(e5)*sin(e4)*sin(e6)) - cos(e6)*(a3*sin(e5) - d4*cos(e4)*cos(e5)) - d4*sin(e4)*sin(e6) + y6*sin(e4)*sin(e5)) - (cos(e5)*(sin(e2)*sin(e3) - cos(e2)*cos(e3)) + cos(e4)*sin(e5)*(cos(e2)*sin(e3) + cos(e3)*sin(e2)))*(a3*cos(e5) - y6*(cos(e4)*sin(e6) + cos(e5)*cos(e6)*sin(e4)) + x6*(cos(e4)*cos(e6) - cos(e5)*sin(e4)*sin(e6)) + d4*cos(e4)*sin(e5)))*((sin(e6)*(sin(e5)*(cos(e2)*sin(e3) + cos(e3)*sin(e2)) + cos(e4)*cos(e5)*(sin(e2)*sin(e3) - cos(e2)*cos(e3))) + cos(e6)*sin(e4)*(sin(e2)*sin(e3) - cos(e2)*cos(e3)))*(x6*(sin(e2 + e3)*cos(e5) + cos(e2 + e3)*cos(e4)*sin(e5)) - z6*(cos(e6)*(sin(e2 + e3)*sin(e5) - cos(e2 + e3)*cos(e4)*cos(e5)) + cos(e2 + e3)*sin(e4)*sin(e6)) + cos(e4)*cos(e6)*(a1 + d4*cos(e2 + e3) + a3*sin(e2 + e3) + a2*sin(e2)) - cos(e5)*sin(e4)*sin(e6)*(a1 + d4*cos(e2 + e3) + a3*sin(e2 + e3) + a2*sin(e2))) + (cos(e6)*(sin(e5)*(cos(e2)*sin(e3) + cos(e3)*sin(e2)) + cos(e4)*cos(e5)*(sin(e2)*sin(e3) - cos(e2)*cos(e3))) - sin(e4)*sin(e6)*(sin(e2)*sin(e3) - cos(e2)*cos(e3)))*(y6*(sin(e2 + e3)*cos(e5) + cos(e2 + e3)*cos(e4)*sin(e5)) + z6*(sin(e6)*(sin(e2 + e3)*sin(e5) - cos(e2 + e3)*cos(e4)*cos(e5)) - cos(e2 + e3)*cos(e6)*sin(e4)) - cos(e4)*sin(e6)*(a1 + d4*cos(e2 + e3) + a3*sin(e2 + e3) + a2*sin(e2)) - cos(e5)*cos(e6)*sin(e4)*(a1 + d4*cos(e2 + e3) + a3*sin(e2 + e3) + a2*sin(e2))) - (cos(e5)*(cos(e2)*sin(e3) + cos(e3)*sin(e2)) - cos(e4)*sin(e5)*(sin(e2)*sin(e3) - cos(e2)*cos(e3)))*(x6*(sin(e6)*(sin(e2 + e3)*sin(e5) - cos(e2 + e3)*cos(e4)*cos(e5)) - cos(e2 + e3)*cos(e6)*sin(e4)) + y6*(cos(e6)*(sin(e2 + e3)*sin(e5) - cos(e2 + e3)*cos(e4)*cos(e5)) + cos(e2 + e3)*sin(e4)*sin(e6)) - sin(e4)*sin(e5)*(a1 + d4*cos(e2 + e3) + a3*sin(e2 + e3) + a2*sin(e2)))) + m6*((sin(e6)*(sin(e5)*(cos(e1)*cos(e2)*cos(e3) - cos(e1)*sin(e2)*sin(e3)) + cos(e5)*(sin(e1)*sin(e4) + cos(e4)*(cos(e1)*cos(e2)*sin(e3) + cos(e1)*cos(e3)*sin(e2)))) - cos(e6)*(cos(e4)*sin(e1) - sin(e4)*(cos(e1)*cos(e2)*sin(e3) + cos(e1)*cos(e3)*sin(e2))))*(z6*(cos(e4)*sin(e6) + cos(e5)*cos(e6)*sin(e4)) - sin(e6)*(a3*sin(e5) - d4*cos(e4)*cos(e5)) + d4*cos(e6)*sin(e4) + x6*sin(e4)*sin(e5)) + (cos(e6)*(sin(e5)*(cos(e1)*cos(e2)*cos(e3) - cos(e1)*sin(e2)*sin(e3)) + cos(e5)*(sin(e1)*sin(e4) + cos(e4)*(cos(e1)*cos(e2)*sin(e3) + cos(e1)*cos(e3)*sin(e2)))) + sin(e6)*(cos(e4)*sin(e1) - sin(e4)*(cos(e1)*cos(e2)*sin(e3) + cos(e1)*cos(e3)*sin(e2))))*(z6*(cos(e4)*cos(e6) - cos(e5)*sin(e4)*sin(e6)) - cos(e6)*(a3*sin(e5) - d4*cos(e4)*cos(e5)) - d4*sin(e4)*sin(e6) + y6*sin(e4)*sin(e5)) - (cos(e5)*(cos(e1)*cos(e2)*cos(e3) - cos(e1)*sin(e2)*sin(e3)) - sin(e5)*(sin(e1)*sin(e4) + cos(e4)*(cos(e1)*cos(e2)*sin(e3) + cos(e1)*cos(e3)*sin(e2))))*(a3*cos(e5) - y6*(cos(e4)*sin(e6) + cos(e5)*cos(e6)*sin(e4)) + x6*(cos(e4)*cos(e6) - cos(e5)*sin(e4)*sin(e6)) + d4*cos(e4)*sin(e5)))*((cos(e5)*(cos(e1)*cos(e2)*cos(e3) - cos(e1)*sin(e2)*sin(e3)) - sin(e5)*(sin(e1)*sin(e4) + cos(e4)*(cos(e1)*cos(e2)*sin(e3) + cos(e1)*cos(e3)*sin(e2))))*(x6*(sin(e6)*(cos(e2 + e3)*sin(e5) + sin(e2 + e3)*cos(e4)*cos(e5)) + sin(e2 + e3)*cos(e6)*sin(e4)) + y6*(cos(e6)*(cos(e2 + e3)*sin(e5) + sin(e2 + e3)*cos(e4)*cos(e5)) - sin(e2 + e3)*sin(e4)*sin(e6)) - sin(e4)*sin(e5)*(a3*cos(e2 + e3) - d4*sin(e2 + e3) + a2*cos(e2))) - (sin(e6)*(sin(e5)*(cos(e1)*cos(e2)*cos(e3) - cos(e1)*sin(e2)*sin(e3)) + cos(e5)*(sin(e1)*sin(e4) + cos(e4)*(cos(e1)*cos(e2)*sin(e3) + cos(e1)*cos(e3)*sin(e2)))) - cos(e6)*(cos(e4)*sin(e1) - sin(e4)*(cos(e1)*cos(e2)*sin(e3) + cos(e1)*cos(e3)*sin(e2))))*(x6*(cos(e2 + e3)*cos(e5) - sin(e2 + e3)*cos(e4)*sin(e5)) - z6*(cos(e6)*(cos(e2 + e3)*sin(e5) + sin(e2 + e3)*cos(e4)*cos(e5)) - sin(e2 + e3)*sin(e4)*sin(e6)) + cos(e4)*cos(e6)*(a3*cos(e2 + e3) - d4*sin(e2 + e3) + a2*cos(e2)) - cos(e5)*sin(e4)*sin(e6)*(a3*cos(e2 + e3) - d4*sin(e2 + e3) + a2*cos(e2))) - (cos(e6)*(sin(e5)*(cos(e1)*cos(e2)*cos(e3) - cos(e1)*sin(e2)*sin(e3)) + cos(e5)*(sin(e1)*sin(e4) + cos(e4)*(cos(e1)*cos(e2)*sin(e3) + cos(e1)*cos(e3)*sin(e2)))) + sin(e6)*(cos(e4)*sin(e1) - sin(e4)*(cos(e1)*cos(e2)*sin(e3) + cos(e1)*cos(e3)*sin(e2))))*(y6*(cos(e2 + e3)*cos(e5) - sin(e2 + e3)*cos(e4)*sin(e5)) + z6*(sin(e6)*(cos(e2 + e3)*sin(e5) + sin(e2 + e3)*cos(e4)*cos(e5)) + sin(e2 + e3)*cos(e6)*sin(e4)) - cos(e4)*sin(e6)*(a3*cos(e2 + e3) - d4*sin(e2 + e3) + a2*cos(e2)) - cos(e5)*cos(e6)*sin(e4)*(a3*cos(e2 + e3) - d4*sin(e2 + e3) + a2*cos(e2))) - (cos(e5)*(cos(e1)*cos(e2)*sin(e3) + cos(e1)*cos(e3)*sin(e2)) + cos(e4)*sin(e5)*(cos(e1)*cos(e2)*cos(e3) - cos(e1)*sin(e2)*sin(e3)))*(x6*(sin(e6)*(sin(e2 + e3)*sin(e5) - cos(e2 + e3)*cos(e4)*cos(e5)) - cos(e2 + e3)*cos(e6)*sin(e4)) + y6*(cos(e6)*(sin(e2 + e3)*sin(e5) - cos(e2 + e3)*cos(e4)*cos(e5)) + cos(e2 + e3)*sin(e4)*sin(e6)) - sin(e4)*sin(e5)*(a1 + d4*cos(e2 + e3) + a3*sin(e2 + e3) + a2*sin(e2))) + (sin(e6)*(sin(e5)*(cos(e1)*cos(e2)*sin(e3) + cos(e1)*cos(e3)*sin(e2)) - cos(e4)*cos(e5)*(cos(e1)*cos(e2)*cos(e3) - cos(e1)*sin(e2)*sin(e3))) - cos(e6)*sin(e4)*(cos(e1)*cos(e2)*cos(e3) - cos(e1)*sin(e2)*sin(e3)))*(x6*(sin(e2 + e3)*cos(e5) + cos(e2 + e3)*cos(e4)*sin(e5)) - z6*(cos(e6)*(sin(e2 + e3)*sin(e5) - cos(e2 + e3)*cos(e4)*cos(e5)) + cos(e2 + e3)*sin(e4)*sin(e6)) + cos(e4)*cos(e6)*(a1 + d4*cos(e2 + e3) + a3*sin(e2 + e3) + a2*sin(e2)) - cos(e5)*sin(e4)*sin(e6)*(a1 + d4*cos(e2 + e3) + a3*sin(e2 + e3) + a2*sin(e2))) + (cos(e6)*(sin(e5)*(cos(e1)*cos(e2)*sin(e3) + cos(e1)*cos(e3)*sin(e2)) - cos(e4)*cos(e5)*(cos(e1)*cos(e2)*cos(e3) - cos(e1)*sin(e2)*sin(e3))) + sin(e4)*sin(e6)*(cos(e1)*cos(e2)*cos(e3) - cos(e1)*sin(e2)*sin(e3)))*(y6*(sin(e2 + e3)*cos(e5) + cos(e2 + e3)*cos(e4)*sin(e5)) + z6*(sin(e6)*(sin(e2 + e3)*sin(e5) - cos(e2 + e3)*cos(e4)*cos(e5)) - cos(e2 + e3)*cos(e6)*sin(e4)) - cos(e4)*sin(e6)*(a1 + d4*cos(e2 + e3) + a3*sin(e2 + e3) + a2*sin(e2)) - cos(e5)*cos(e6)*sin(e4)*(a1 + d4*cos(e2 + e3) + a3*sin(e2 + e3) + a2*sin(e2)))) - m3*sin(e1)*(x3*cos(e2 + e3)*cos(e1) - y3*sin(e2 + e3)*cos(e1))*(x3*cos(e2 + e3) - y3*sin(e2 + e3) + a2*cos(e2)) + m3*cos(e1)*(x3*cos(e2 + e3)*sin(e1) - y3*sin(e2 + e3)*sin(e1))*(x3*cos(e2 + e3) - y3*sin(e2 + e3) + a2*cos(e2))) + (de5*(0.5*I5xz*(cos(e2 + e3)*sin(e5) + sin(e2 + e3)*cos(e4)*cos(e5)) + 0.5*I5zx*(cos(e2 + e3)*sin(e5) + sin(e2 + e3)*cos(e4)*cos(e5)) + 0.5*(I6yy*cos(e6) + I6xy*sin(e6))*(sin(e6)*(cos(e2 + e3)*sin(e5) + sin(e2 + e3)*cos(e4)*cos(e5)) + sin(e2 + e3)*cos(e6)*sin(e4)) + 0.5*I5yz*(cos(e2 + e3)*cos(e5) - 1.0*sin(e2 + e3)*cos(e4)*sin(e5)) + 0.5*I5zy*(cos(e2 + e3)*cos(e5) - 1.0*sin(e2 + e3)*cos(e4)*sin(e5)) - 0.5*(I6yz*cos(e6) + I6xz*sin(e6))*(cos(e2 + e3)*cos(e5) - 1.0*sin(e2 + e3)*cos(e4)*sin(e5)) - 0.5*cos(e6)*(I6zy*(cos(e2 + e3)*cos(e5) - 1.0*sin(e2 + e3)*cos(e4)*sin(e5)) - 1.0*I6yy*(sin(e6)*(cos(e2 + e3)*sin(e5) + sin(e2 + e3)*cos(e4)*cos(e5)) + sin(e2 + e3)*cos(e6)*sin(e4)) + I6xy*(cos(e6)*(cos(e2 + e3)*sin(e5) + sin(e2 + e3)*cos(e4)*cos(e5)) - 1.0*sin(e2 + e3)*sin(e4)*sin(e6))) - 0.5*sin(e6)*(I6zx*(cos(e2 + e3)*cos(e5) - 1.0*sin(e2 + e3)*cos(e4)*sin(e5)) - 1.0*I6yx*(sin(e6)*(cos(e2 + e3)*sin(e5) + sin(e2 + e3)*cos(e4)*cos(e5)) + sin(e2 + e3)*cos(e6)*sin(e4)) + I6xx*(cos(e6)*(cos(e2 + e3)*sin(e5) + sin(e2 + e3)*cos(e4)*cos(e5)) - 1.0*sin(e2 + e3)*sin(e4)*sin(e6))) - 0.5*(cos(e6)*(cos(e2 + e3)*sin(e5) + sin(e2 + e3)*cos(e4)*cos(e5)) - 1.0*sin(e2 + e3)*sin(e4)*sin(e6))*(I6yx*cos(e6) + I6xx*sin(e6)) + m6*(1.0*(sin(e5)*(cos(e1)*sin(e4) - 1.0*cos(e4)*(cos(e2)*sin(e1)*sin(e3) + cos(e3)*sin(e1)*sin(e2))) + cos(e5)*(cos(e2)*cos(e3)*sin(e1) - 1.0*sin(e1)*sin(e2)*sin(e3)))*(x6*cos(e6) - 1.0*y6*sin(e6)) + z6*sin(e6)*(sin(e6)*(1.0*cos(e5)*(cos(e1)*sin(e4) - 1.0*cos(e4)*(cos(e2)*sin(e1)*sin(e3) + cos(e3)*sin(e1)*sin(e2))) - sin(e5)*(cos(e2)*cos(e3)*sin(e1) - 1.0*sin(e1)*sin(e2)*sin(e3))) - cos(e6)*(sin(e4)*(cos(e2)*sin(e1)*sin(e3) + cos(e3)*sin(e1)*sin(e2)) + cos(e1)*cos(e4))) + z6*cos(e6)*(cos(e6)*(1.0*cos(e5)*(cos(e1)*sin(e4) - 1.0*cos(e4)*(cos(e2)*sin(e1)*sin(e3) + cos(e3)*sin(e1)*sin(e2))) - sin(e5)*(cos(e2)*cos(e3)*sin(e1) - 1.0*sin(e1)*sin(e2)*sin(e3))) + 1.0*sin(e6)*(sin(e4)*(cos(e2)*sin(e1)*sin(e3) + cos(e3)*sin(e1)*sin(e2)) + cos(e1)*cos(e4))))*((sin(e6)*(sin(e5)*(cos(e2)*sin(e1)*sin(e3) + cos(e3)*sin(e1)*sin(e2)) - 1.0*cos(e4)*cos(e5)*(cos(e2)*cos(e3)*sin(e1) - 1.0*sin(e1)*sin(e2)*sin(e3))) - 1.0*cos(e6)*sin(e4)*(cos(e2)*cos(e3)*sin(e1) - 1.0*sin(e1)*sin(e2)*sin(e3)))*(x6*(sin(e2 + e3)*cos(e5) + cos(e2 + e3)*cos(e4)*sin(e5)) - 1.0*z6*(cos(e6)*(sin(e2 + e3)*sin(e5) - 1.0*cos(e2 + e3)*cos(e4)*cos(e5)) + cos(e2 + e3)*sin(e4)*sin(e6)) + cos(e4)*cos(e6)*(a1 + d4*cos(e2 + e3) + a3*sin(e2 + e3) + a2*sin(e2)) - 1.0*cos(e5)*sin(e4)*sin(e6)*(a1 + d4*cos(e2 + e3) + a3*sin(e2 + e3) + a2*sin(e2))) - 1.0*(cos(e5)*(cos(e2)*sin(e1)*sin(e3) + cos(e3)*sin(e1)*sin(e2)) + cos(e4)*sin(e5)*(cos(e2)*cos(e3)*sin(e1) - 1.0*sin(e1)*sin(e2)*sin(e3)))*(x6*(sin(e6)*(sin(e2 + e3)*sin(e5) - 1.0*cos(e2 + e3)*cos(e4)*cos(e5)) - 1.0*cos(e2 + e3)*cos(e6)*sin(e4)) + y6*(cos(e6)*(sin(e2 + e3)*sin(e5) - 1.0*cos(e2 + e3)*cos(e4)*cos(e5)) + cos(e2 + e3)*sin(e4)*sin(e6)) - 1.0*sin(e4)*sin(e5)*(a1 + d4*cos(e2 + e3) + a3*sin(e2 + e3) + a2*sin(e2))) + (cos(e6)*(sin(e5)*(cos(e2)*sin(e1)*sin(e3) + cos(e3)*sin(e1)*sin(e2)) - 1.0*cos(e4)*cos(e5)*(cos(e2)*cos(e3)*sin(e1) - 1.0*sin(e1)*sin(e2)*sin(e3))) + sin(e4)*sin(e6)*(cos(e2)*cos(e3)*sin(e1) - 1.0*sin(e1)*sin(e2)*sin(e3)))*(z6*(sin(e6)*(sin(e2 + e3)*sin(e5) - 1.0*cos(e2 + e3)*cos(e4)*cos(e5)) - 1.0*cos(e2 + e3)*cos(e6)*sin(e4)) + y6*(sin(e2 + e3)*cos(e5) + cos(e2 + e3)*cos(e4)*sin(e5)) - 1.0*cos(e4)*sin(e6)*(a1 + d4*cos(e2 + e3) + a3*sin(e2 + e3) + a2*sin(e2)) - 1.0*cos(e5)*cos(e6)*sin(e4)*(a1 + d4*cos(e2 + e3) + a3*sin(e2 + e3) + a2*sin(e2))) + 1.0*(sin(e6)*(1.0*cos(e5)*(cos(e1)*sin(e4) - 1.0*cos(e4)*(cos(e2)*sin(e1)*sin(e3) + cos(e3)*sin(e1)*sin(e2))) - sin(e5)*(cos(e2)*cos(e3)*sin(e1) - 1.0*sin(e1)*sin(e2)*sin(e3))) - cos(e6)*(sin(e4)*(cos(e2)*sin(e1)*sin(e3) + cos(e3)*sin(e1)*sin(e2)) + cos(e1)*cos(e4)))*(x6*(cos(e2 + e3)*cos(e5) - 1.0*sin(e2 + e3)*cos(e4)*sin(e5)) - 1.0*z6*(cos(e6)*(cos(e2 + e3)*sin(e5) + sin(e2 + e3)*cos(e4)*cos(e5)) - 1.0*sin(e2 + e3)*sin(e4)*sin(e6)) + cos(e4)*cos(e6)*(a3*cos(e2 + e3) - 1.0*d4*sin(e2 + e3)) - 1.0*cos(e5)*sin(e4)*sin(e6)*(a3*cos(e2 + e3) - 1.0*d4*sin(e2 + e3))) + 1.0*(cos(e6)*(1.0*cos(e5)*(cos(e1)*sin(e4) - 1.0*cos(e4)*(cos(e2)*sin(e1)*sin(e3) + cos(e3)*sin(e1)*sin(e2))) - sin(e5)*(cos(e2)*cos(e3)*sin(e1) - 1.0*sin(e1)*sin(e2)*sin(e3))) + 1.0*sin(e6)*(sin(e4)*(cos(e2)*sin(e1)*sin(e3) + cos(e3)*sin(e1)*sin(e2)) + cos(e1)*cos(e4)))*(z6*(sin(e6)*(cos(e2 + e3)*sin(e5) + sin(e2 + e3)*cos(e4)*cos(e5)) + sin(e2 + e3)*cos(e6)*sin(e4)) + y6*(cos(e2 + e3)*cos(e5) - 1.0*sin(e2 + e3)*cos(e4)*sin(e5)) - 1.0*cos(e4)*sin(e6)*(a3*cos(e2 + e3) - 1.0*d4*sin(e2 + e3)) - 1.0*cos(e5)*cos(e6)*sin(e4)*(a3*cos(e2 + e3) - 1.0*d4*sin(e2 + e3))) + (sin(e5)*(cos(e1)*sin(e4) - 1.0*cos(e4)*(cos(e2)*sin(e1)*sin(e3) + cos(e3)*sin(e1)*sin(e2))) + cos(e5)*(cos(e2)*cos(e3)*sin(e1) - 1.0*sin(e1)*sin(e2)*sin(e3)))*(x6*(sin(e6)*(cos(e2 + e3)*sin(e5) + sin(e2 + e3)*cos(e4)*cos(e5)) + sin(e2 + e3)*cos(e6)*sin(e4)) + y6*(cos(e6)*(cos(e2 + e3)*sin(e5) + sin(e2 + e3)*cos(e4)*cos(e5)) - 1.0*sin(e2 + e3)*sin(e4)*sin(e6)) - 1.0*sin(e4)*sin(e5)*(a3*cos(e2 + e3) - 1.0*d4*sin(e2 + e3)))) - m6*(z6*cos(e6)*(cos(e6)*(sin(e5)*(sin(e2)*sin(e3) - 1.0*cos(e2)*cos(e3)) - 1.0*cos(e4)*cos(e5)*(cos(e2)*sin(e3) + cos(e3)*sin(e2))) + sin(e4)*sin(e6)*(cos(e2)*sin(e3) + cos(e3)*sin(e2))) - 1.0*(cos(e5)*(sin(e2)*sin(e3) - 1.0*cos(e2)*cos(e3)) + cos(e4)*sin(e5)*(cos(e2)*sin(e3) + cos(e3)*sin(e2)))*(x6*cos(e6) - 1.0*y6*sin(e6)) + z6*sin(e6)*(sin(e6)*(sin(e5)*(sin(e2)*sin(e3) - 1.0*cos(e2)*cos(e3)) - 1.0*cos(e4)*cos(e5)*(cos(e2)*sin(e3) + cos(e3)*sin(e2))) - 1.0*cos(e6)*sin(e4)*(cos(e2)*sin(e3) + cos(e3)*sin(e2))))*((sin(e6)*(sin(e5)*(cos(e2)*sin(e3) + cos(e3)*sin(e2)) + cos(e4)*cos(e5)*(sin(e2)*sin(e3) - 1.0*cos(e2)*cos(e3))) + cos(e6)*sin(e4)*(sin(e2)*sin(e3) - 1.0*cos(e2)*cos(e3)))*(x6*(sin(e2 + e3)*cos(e5) + cos(e2 + e3)*cos(e4)*sin(e5)) - 1.0*z6*(cos(e6)*(sin(e2 + e3)*sin(e5) - 1.0*cos(e2 + e3)*cos(e4)*cos(e5)) + cos(e2 + e3)*sin(e4)*sin(e6)) + cos(e4)*cos(e6)*(a1 + d4*cos(e2 + e3) + a3*sin(e2 + e3) + a2*sin(e2)) - 1.0*cos(e5)*sin(e4)*sin(e6)*(a1 + d4*cos(e2 + e3) + a3*sin(e2 + e3) + a2*sin(e2))) + (cos(e6)*(sin(e5)*(cos(e2)*sin(e3) + cos(e3)*sin(e2)) + cos(e4)*cos(e5)*(sin(e2)*sin(e3) - 1.0*cos(e2)*cos(e3))) - 1.0*sin(e4)*sin(e6)*(sin(e2)*sin(e3) - 1.0*cos(e2)*cos(e3)))*(z6*(sin(e6)*(sin(e2 + e3)*sin(e5) - 1.0*cos(e2 + e3)*cos(e4)*cos(e5)) - 1.0*cos(e2 + e3)*cos(e6)*sin(e4)) + y6*(sin(e2 + e3)*cos(e5) + cos(e2 + e3)*cos(e4)*sin(e5)) - 1.0*cos(e4)*sin(e6)*(a1 + d4*cos(e2 + e3) + a3*sin(e2 + e3) + a2*sin(e2)) - 1.0*cos(e5)*cos(e6)*sin(e4)*(a1 + d4*cos(e2 + e3) + a3*sin(e2 + e3) + a2*sin(e2))) - 1.0*(cos(e5)*(cos(e2)*sin(e3) + cos(e3)*sin(e2)) - 1.0*cos(e4)*sin(e5)*(sin(e2)*sin(e3) - 1.0*cos(e2)*cos(e3)))*(x6*(sin(e6)*(sin(e2 + e3)*sin(e5) - 1.0*cos(e2 + e3)*cos(e4)*cos(e5)) - 1.0*cos(e2 + e3)*cos(e6)*sin(e4)) + y6*(cos(e6)*(sin(e2 + e3)*sin(e5) - 1.0*cos(e2 + e3)*cos(e4)*cos(e5)) + cos(e2 + e3)*sin(e4)*sin(e6)) - 1.0*sin(e4)*sin(e5)*(a1 + d4*cos(e2 + e3) + a3*sin(e2 + e3) + a2*sin(e2)))) + 1.0*I5zz*sin(e2 + e3)*sin(e4) - m5*(x5*(cos(e5)*(cos(e1)*cos(e2)*sin(e3) + cos(e1)*cos(e3)*sin(e2)) + cos(e4)*sin(e5)*(cos(e1)*cos(e2)*cos(e3) - 1.0*cos(e1)*sin(e2)*sin(e3))) - 1.0*y5*(sin(e5)*(cos(e1)*cos(e2)*sin(e3) + cos(e1)*cos(e3)*sin(e2)) - 1.0*cos(e4)*cos(e5)*(cos(e1)*cos(e2)*cos(e3) - 1.0*cos(e1)*sin(e2)*sin(e3))))*((sin(e5)*(cos(e1)*cos(e2)*cos(e3) - 1.0*cos(e1)*sin(e2)*sin(e3)) + cos(e5)*(sin(e1)*sin(e4) + cos(e4)*(cos(e1)*cos(e2)*sin(e3) + cos(e1)*cos(e3)*sin(e2))))*(z5*(sin(e2 + e3)*cos(e5) + cos(e2 + e3)*cos(e4)*sin(e5)) + cos(e5)*sin(e4)*(a1 + d4*cos(e2 + e3) + a3*sin(e2 + e3) + a2*sin(e2)) + y5*cos(e2 + e3)*sin(e4)) + (cos(e4)*sin(e1) - 1.0*sin(e4)*(cos(e1)*cos(e2)*sin(e3) + cos(e1)*cos(e3)*sin(e2)))*(cos(e4)*(a1 + d4*cos(e2 + e3) + a3*sin(e2 + e3) + a2*sin(e2)) + x5*(sin(e2 + e3)*cos(e5) + cos(e2 + e3)*cos(e4)*sin(e5)) - 1.0*y5*(sin(e2 + e3)*sin(e5) - 1.0*cos(e2 + e3)*cos(e4)*cos(e5))) - 1.0*(cos(e5)*(cos(e1)*cos(e2)*cos(e3) - 1.0*cos(e1)*sin(e2)*sin(e3)) - 1.0*sin(e5)*(sin(e1)*sin(e4) + cos(e4)*(cos(e1)*cos(e2)*sin(e3) + cos(e1)*cos(e3)*sin(e2))))*(z5*(sin(e2 + e3)*sin(e5) - 1.0*cos(e2 + e3)*cos(e4)*cos(e5)) + sin(e4)*sin(e5)*(a1 + d4*cos(e2 + e3) + a3*sin(e2 + e3) + a2*sin(e2)) + x5*cos(e2 + e3)*sin(e4))) - m5*(1.0*y5*(1.0*cos(e5)*(cos(e1)*sin(e4) - 1.0*cos(e4)*(cos(e2)*sin(e1)*sin(e3) + cos(e3)*sin(e1)*sin(e2))) - sin(e5)*(cos(e2)*cos(e3)*sin(e1) - 1.0*sin(e1)*sin(e2)*sin(e3))) + x5*(sin(e5)*(cos(e1)*sin(e4) - 1.0*cos(e4)*(cos(e2)*sin(e1)*sin(e3) + cos(e3)*sin(e1)*sin(e2))) + cos(e5)*(cos(e2)*cos(e3)*sin(e1) - 1.0*sin(e1)*sin(e2)*sin(e3))))*((sin(e5)*(cos(e1)*sin(e4) - 1.0*cos(e4)*(cos(e2)*sin(e1)*sin(e3) + cos(e3)*sin(e1)*sin(e2))) + cos(e5)*(cos(e2)*cos(e3)*sin(e1) - 1.0*sin(e1)*sin(e2)*sin(e3)))*(z5*(cos(e2 + e3)*sin(e5) + sin(e2 + e3)*cos(e4)*cos(e5)) - 1.0*x5*sin(e2 + e3)*sin(e4) + sin(e4)*sin(e5)*(a3*cos(e2 + e3) - 1.0*d4*sin(e2 + e3))) + (sin(e4)*(cos(e2)*sin(e1)*sin(e3) + cos(e3)*sin(e1)*sin(e2)) + cos(e1)*cos(e4))*(cos(e4)*(a3*cos(e2 + e3) - 1.0*d4*sin(e2 + e3)) - 1.0*y5*(cos(e2 + e3)*sin(e5) + sin(e2 + e3)*cos(e4)*cos(e5)) + x5*(cos(e2 + e3)*cos(e5) - 1.0*sin(e2 + e3)*cos(e4)*sin(e5))) + 1.0*(1.0*cos(e5)*(cos(e1)*sin(e4) - 1.0*cos(e4)*(cos(e2)*sin(e1)*sin(e3) + cos(e3)*sin(e1)*sin(e2))) - sin(e5)*(cos(e2)*cos(e3)*sin(e1) - 1.0*sin(e1)*sin(e2)*sin(e3)))*(z5*(cos(e2 + e3)*cos(e5) - 1.0*sin(e2 + e3)*cos(e4)*sin(e5)) + cos(e5)*sin(e4)*(a3*cos(e2 + e3) - 1.0*d4*sin(e2 + e3)) - 1.0*y5*sin(e2 + e3)*sin(e4)) + (sin(e5)*(cos(e2)*sin(e1)*sin(e3) + cos(e3)*sin(e1)*sin(e2)) - 1.0*cos(e4)*cos(e5)*(cos(e2)*cos(e3)*sin(e1) - 1.0*sin(e1)*sin(e2)*sin(e3)))*(z5*(sin(e2 + e3)*cos(e5) + cos(e2 + e3)*cos(e4)*sin(e5)) + cos(e5)*sin(e4)*(a1 + d4*cos(e2 + e3) + a3*sin(e2 + e3) + a2*sin(e2)) + y5*cos(e2 + e3)*sin(e4)) - 1.0*(cos(e5)*(cos(e2)*sin(e1)*sin(e3) + cos(e3)*sin(e1)*sin(e2)) + cos(e4)*sin(e5)*(cos(e2)*cos(e3)*sin(e1) - 1.0*sin(e1)*sin(e2)*sin(e3)))*(z5*(sin(e2 + e3)*sin(e5) - 1.0*cos(e2 + e3)*cos(e4)*cos(e5)) + sin(e4)*sin(e5)*(a1 + d4*cos(e2 + e3) + a3*sin(e2 + e3) + a2*sin(e2)) + x5*cos(e2 + e3)*sin(e4)) + sin(e4)*(cos(e2)*cos(e3)*sin(e1) - 1.0*sin(e1)*sin(e2)*sin(e3))*(cos(e4)*(a1 + d4*cos(e2 + e3) + a3*sin(e2 + e3) + a2*sin(e2)) + x5*(sin(e2 + e3)*cos(e5) + cos(e2 + e3)*cos(e4)*sin(e5)) - 1.0*y5*(sin(e2 + e3)*sin(e5) - 1.0*cos(e2 + e3)*cos(e4)*cos(e5)))) + 1.0*m5*(1.0*y5*(sin(e5)*(cos(e1)*cos(e2)*cos(e3) - 1.0*cos(e1)*sin(e2)*sin(e3)) + cos(e5)*(sin(e1)*sin(e4) + cos(e4)*(cos(e1)*cos(e2)*sin(e3) + cos(e1)*cos(e3)*sin(e2)))) - x5*(cos(e5)*(cos(e1)*cos(e2)*cos(e3) - 1.0*cos(e1)*sin(e2)*sin(e3)) - 1.0*sin(e5)*(sin(e1)*sin(e4) + cos(e4)*(cos(e1)*cos(e2)*sin(e3) + cos(e1)*cos(e3)*sin(e2)))))*(1.0*(sin(e5)*(cos(e1)*cos(e2)*sin(e3) + cos(e1)*cos(e3)*sin(e2)) - 1.0*cos(e4)*cos(e5)*(cos(e1)*cos(e2)*cos(e3) - 1.0*cos(e1)*sin(e2)*sin(e3)))*(z5*(sin(e2 + e3)*cos(e5) + cos(e2 + e3)*cos(e4)*sin(e5)) + cos(e5)*sin(e4)*(a1 + d4*cos(e2 + e3) + a3*sin(e2 + e3) + a2*sin(e2)) + y5*cos(e2 + e3)*sin(e4)) - (cos(e5)*(cos(e1)*cos(e2)*sin(e3) + cos(e1)*cos(e3)*sin(e2)) + cos(e4)*sin(e5)*(cos(e1)*cos(e2)*cos(e3) - 1.0*cos(e1)*sin(e2)*sin(e3)))*(z5*(sin(e2 + e3)*sin(e5) - 1.0*cos(e2 + e3)*cos(e4)*cos(e5)) + sin(e4)*sin(e5)*(a1 + d4*cos(e2 + e3) + a3*sin(e2 + e3) + a2*sin(e2)) + x5*cos(e2 + e3)*sin(e4)) - (cos(e4)*sin(e1) - 1.0*sin(e4)*(cos(e1)*cos(e2)*sin(e3) + cos(e1)*cos(e3)*sin(e2)))*(cos(e4)*(a3*cos(e2 + e3) - 1.0*d4*sin(e2 + e3)) - 1.0*y5*(cos(e2 + e3)*sin(e5) + sin(e2 + e3)*cos(e4)*cos(e5)) + x5*(cos(e2 + e3)*cos(e5) - 1.0*sin(e2 + e3)*cos(e4)*sin(e5))) - (sin(e5)*(cos(e1)*cos(e2)*cos(e3) - 1.0*cos(e1)*sin(e2)*sin(e3)) + cos(e5)*(sin(e1)*sin(e4) + cos(e4)*(cos(e1)*cos(e2)*sin(e3) + cos(e1)*cos(e3)*sin(e2))))*(z5*(cos(e2 + e3)*cos(e5) - 1.0*sin(e2 + e3)*cos(e4)*sin(e5)) + cos(e5)*sin(e4)*(a3*cos(e2 + e3) - 1.0*d4*sin(e2 + e3)) - 1.0*y5*sin(e2 + e3)*sin(e4)) + 1.0*(cos(e5)*(cos(e1)*cos(e2)*cos(e3) - 1.0*cos(e1)*sin(e2)*sin(e3)) - 1.0*sin(e5)*(sin(e1)*sin(e4) + cos(e4)*(cos(e1)*cos(e2)*sin(e3) + cos(e1)*cos(e3)*sin(e2))))*(z5*(cos(e2 + e3)*sin(e5) + sin(e2 + e3)*cos(e4)*cos(e5)) - 1.0*x5*sin(e2 + e3)*sin(e4) + sin(e4)*sin(e5)*(a3*cos(e2 + e3) - 1.0*d4*sin(e2 + e3))) + 1.0*sin(e4)*(cos(e1)*cos(e2)*cos(e3) - 1.0*cos(e1)*sin(e2)*sin(e3))*(cos(e4)*(a1 + d4*cos(e2 + e3) + a3*sin(e2 + e3) + a2*sin(e2)) + x5*(sin(e2 + e3)*cos(e5) + cos(e2 + e3)*cos(e4)*sin(e5)) - 1.0*y5*(sin(e2 + e3)*sin(e5) - 1.0*cos(e2 + e3)*cos(e4)*cos(e5)))) - 1.0*m5*(1.0*y5*(sin(e5)*(cos(e2)*sin(e1)*sin(e3) + cos(e3)*sin(e1)*sin(e2)) - 1.0*cos(e4)*cos(e5)*(cos(e2)*cos(e3)*sin(e1) - 1.0*sin(e1)*sin(e2)*sin(e3))) - x5*(cos(e5)*(cos(e2)*sin(e1)*sin(e3) + cos(e3)*sin(e1)*sin(e2)) + cos(e4)*sin(e5)*(cos(e2)*cos(e3)*sin(e1) - 1.0*sin(e1)*sin(e2)*sin(e3))))*((sin(e4)*(cos(e2)*sin(e1)*sin(e3) + cos(e3)*sin(e1)*sin(e2)) + cos(e1)*cos(e4))*(cos(e4)*(a1 + d4*cos(e2 + e3) + a3*sin(e2 + e3) + a2*sin(e2)) + x5*(sin(e2 + e3)*cos(e5) + cos(e2 + e3)*cos(e4)*sin(e5)) - 1.0*y5*(sin(e2 + e3)*sin(e5) - 1.0*cos(e2 + e3)*cos(e4)*cos(e5))) + 1.0*(1.0*cos(e5)*(cos(e1)*sin(e4) - 1.0*cos(e4)*(cos(e2)*sin(e1)*sin(e3) + cos(e3)*sin(e1)*sin(e2))) - sin(e5)*(cos(e2)*cos(e3)*sin(e1) - 1.0*sin(e1)*sin(e2)*sin(e3)))*(z5*(sin(e2 + e3)*cos(e5) + cos(e2 + e3)*cos(e4)*sin(e5)) + cos(e5)*sin(e4)*(a1 + d4*cos(e2 + e3) + a3*sin(e2 + e3) + a2*sin(e2)) + y5*cos(e2 + e3)*sin(e4)) + (sin(e5)*(cos(e1)*sin(e4) - 1.0*cos(e4)*(cos(e2)*sin(e1)*sin(e3) + cos(e3)*sin(e1)*sin(e2))) + cos(e5)*(cos(e2)*cos(e3)*sin(e1) - 1.0*sin(e1)*sin(e2)*sin(e3)))*(z5*(sin(e2 + e3)*sin(e5) - 1.0*cos(e2 + e3)*cos(e4)*cos(e5)) + sin(e4)*sin(e5)*(a1 + d4*cos(e2 + e3) + a3*sin(e2 + e3) + a2*sin(e2)) + x5*cos(e2 + e3)*sin(e4))) - m6*((sin(e6)*(sin(e5)*(cos(e1)*cos(e2)*cos(e3) - 1.0*cos(e1)*sin(e2)*sin(e3)) + cos(e5)*(sin(e1)*sin(e4) + cos(e4)*(cos(e1)*cos(e2)*sin(e3) + cos(e1)*cos(e3)*sin(e2)))) - 1.0*cos(e6)*(cos(e4)*sin(e1) - 1.0*sin(e4)*(cos(e1)*cos(e2)*sin(e3) + cos(e1)*cos(e3)*sin(e2))))*(x6*(sin(e2 + e3)*cos(e5) + cos(e2 + e3)*cos(e4)*sin(e5)) - 1.0*z6*(cos(e6)*(sin(e2 + e3)*sin(e5) - 1.0*cos(e2 + e3)*cos(e4)*cos(e5)) + cos(e2 + e3)*sin(e4)*sin(e6)) + cos(e4)*cos(e6)*(a1 + d4*cos(e2 + e3) + a3*sin(e2 + e3) + a2*sin(e2)) - 1.0*cos(e5)*sin(e4)*sin(e6)*(a1 + d4*cos(e2 + e3) + a3*sin(e2 + e3) + a2*sin(e2))) + (sin(e6)*(cos(e4)*sin(e1) - 1.0*sin(e4)*(cos(e1)*cos(e2)*sin(e3) + cos(e1)*cos(e3)*sin(e2))) + cos(e6)*(sin(e5)*(cos(e1)*cos(e2)*cos(e3) - 1.0*cos(e1)*sin(e2)*sin(e3)) + cos(e5)*(sin(e1)*sin(e4) + cos(e4)*(cos(e1)*cos(e2)*sin(e3) + cos(e1)*cos(e3)*sin(e2)))))*(z6*(sin(e6)*(sin(e2 + e3)*sin(e5) - 1.0*cos(e2 + e3)*cos(e4)*cos(e5)) - 1.0*cos(e2 + e3)*cos(e6)*sin(e4)) + y6*(sin(e2 + e3)*cos(e5) + cos(e2 + e3)*cos(e4)*sin(e5)) - 1.0*cos(e4)*sin(e6)*(a1 + d4*cos(e2 + e3) + a3*sin(e2 + e3) + a2*sin(e2)) - 1.0*cos(e5)*cos(e6)*sin(e4)*(a1 + d4*cos(e2 + e3) + a3*sin(e2 + e3) + a2*sin(e2))) - 1.0*(cos(e5)*(cos(e1)*cos(e2)*cos(e3) - 1.0*cos(e1)*sin(e2)*sin(e3)) - 1.0*sin(e5)*(sin(e1)*sin(e4) + cos(e4)*(cos(e1)*cos(e2)*sin(e3) + cos(e1)*cos(e3)*sin(e2))))*(x6*(sin(e6)*(sin(e2 + e3)*sin(e5) - 1.0*cos(e2 + e3)*cos(e4)*cos(e5)) - 1.0*cos(e2 + e3)*cos(e6)*sin(e4)) + y6*(cos(e6)*(sin(e2 + e3)*sin(e5) - 1.0*cos(e2 + e3)*cos(e4)*cos(e5)) + cos(e2 + e3)*sin(e4)*sin(e6)) - 1.0*sin(e4)*sin(e5)*(a1 + d4*cos(e2 + e3) + a3*sin(e2 + e3) + a2*sin(e2))))*(z6*cos(e6)*(cos(e6)*(sin(e5)*(cos(e1)*cos(e2)*sin(e3) + cos(e1)*cos(e3)*sin(e2)) - 1.0*cos(e4)*cos(e5)*(cos(e1)*cos(e2)*cos(e3) - 1.0*cos(e1)*sin(e2)*sin(e3))) + sin(e4)*sin(e6)*(cos(e1)*cos(e2)*cos(e3) - 1.0*cos(e1)*sin(e2)*sin(e3))) - 1.0*(cos(e5)*(cos(e1)*cos(e2)*sin(e3) + cos(e1)*cos(e3)*sin(e2)) + cos(e4)*sin(e5)*(cos(e1)*cos(e2)*cos(e3) - 1.0*cos(e1)*sin(e2)*sin(e3)))*(x6*cos(e6) - 1.0*y6*sin(e6)) + z6*sin(e6)*(sin(e6)*(sin(e5)*(cos(e1)*cos(e2)*sin(e3) + cos(e1)*cos(e3)*sin(e2)) - 1.0*cos(e4)*cos(e5)*(cos(e1)*cos(e2)*cos(e3) - 1.0*cos(e1)*sin(e2)*sin(e3))) - 1.0*cos(e6)*sin(e4)*(cos(e1)*cos(e2)*cos(e3) - 1.0*cos(e1)*sin(e2)*sin(e3)))) + 1.0*m6*(z6*cos(e6)*(sin(e6)*(cos(e4)*sin(e1) - 1.0*sin(e4)*(cos(e1)*cos(e2)*sin(e3) + cos(e1)*cos(e3)*sin(e2))) + cos(e6)*(sin(e5)*(cos(e1)*cos(e2)*cos(e3) - 1.0*cos(e1)*sin(e2)*sin(e3)) + cos(e5)*(sin(e1)*sin(e4) + cos(e4)*(cos(e1)*cos(e2)*sin(e3) + cos(e1)*cos(e3)*sin(e2))))) - 1.0*(cos(e5)*(cos(e1)*cos(e2)*cos(e3) - 1.0*cos(e1)*sin(e2)*sin(e3)) - 1.0*sin(e5)*(sin(e1)*sin(e4) + cos(e4)*(cos(e1)*cos(e2)*sin(e3) + cos(e1)*cos(e3)*sin(e2))))*(x6*cos(e6) - 1.0*y6*sin(e6)) + z6*sin(e6)*(sin(e6)*(sin(e5)*(cos(e1)*cos(e2)*cos(e3) - 1.0*cos(e1)*sin(e2)*sin(e3)) + cos(e5)*(sin(e1)*sin(e4) + cos(e4)*(cos(e1)*cos(e2)*sin(e3) + cos(e1)*cos(e3)*sin(e2)))) - 1.0*cos(e6)*(cos(e4)*sin(e1) - 1.0*sin(e4)*(cos(e1)*cos(e2)*sin(e3) + cos(e1)*cos(e3)*sin(e2)))))*((sin(e6)*(cos(e4)*sin(e1) - 1.0*sin(e4)*(cos(e1)*cos(e2)*sin(e3) + cos(e1)*cos(e3)*sin(e2))) + cos(e6)*(sin(e5)*(cos(e1)*cos(e2)*cos(e3) - 1.0*cos(e1)*sin(e2)*sin(e3)) + cos(e5)*(sin(e1)*sin(e4) + cos(e4)*(cos(e1)*cos(e2)*sin(e3) + cos(e1)*cos(e3)*sin(e2)))))*(z6*(sin(e6)*(cos(e2 + e3)*sin(e5) + sin(e2 + e3)*cos(e4)*cos(e5)) + sin(e2 + e3)*cos(e6)*sin(e4)) + y6*(cos(e2 + e3)*cos(e5) - 1.0*sin(e2 + e3)*cos(e4)*sin(e5)) - 1.0*cos(e4)*sin(e6)*(a3*cos(e2 + e3) - 1.0*d4*sin(e2 + e3)) - 1.0*cos(e5)*cos(e6)*sin(e4)*(a3*cos(e2 + e3) - 1.0*d4*sin(e2 + e3))) - 1.0*(sin(e6)*(sin(e5)*(cos(e1)*cos(e2)*sin(e3) + cos(e1)*cos(e3)*sin(e2)) - 1.0*cos(e4)*cos(e5)*(cos(e1)*cos(e2)*cos(e3) - 1.0*cos(e1)*sin(e2)*sin(e3))) - 1.0*cos(e6)*sin(e4)*(cos(e1)*cos(e2)*cos(e3) - 1.0*cos(e1)*sin(e2)*sin(e3)))*(x6*(sin(e2 + e3)*cos(e5) + cos(e2 + e3)*cos(e4)*sin(e5)) - 1.0*z6*(cos(e6)*(sin(e2 + e3)*sin(e5) - 1.0*cos(e2 + e3)*cos(e4)*cos(e5)) + cos(e2 + e3)*sin(e4)*sin(e6)) + cos(e4)*cos(e6)*(a1 + d4*cos(e2 + e3) + a3*sin(e2 + e3) + a2*sin(e2)) - 1.0*cos(e5)*sin(e4)*sin(e6)*(a1 + d4*cos(e2 + e3) + a3*sin(e2 + e3) + a2*sin(e2))) - 1.0*(cos(e6)*(sin(e5)*(cos(e1)*cos(e2)*sin(e3) + cos(e1)*cos(e3)*sin(e2)) - 1.0*cos(e4)*cos(e5)*(cos(e1)*cos(e2)*cos(e3) - 1.0*cos(e1)*sin(e2)*sin(e3))) + sin(e4)*sin(e6)*(cos(e1)*cos(e2)*cos(e3) - 1.0*cos(e1)*sin(e2)*sin(e3)))*(z6*(sin(e6)*(sin(e2 + e3)*sin(e5) - 1.0*cos(e2 + e3)*cos(e4)*cos(e5)) - 1.0*cos(e2 + e3)*cos(e6)*sin(e4)) + y6*(sin(e2 + e3)*cos(e5) + cos(e2 + e3)*cos(e4)*sin(e5)) - 1.0*cos(e4)*sin(e6)*(a1 + d4*cos(e2 + e3) + a3*sin(e2 + e3) + a2*sin(e2)) - 1.0*cos(e5)*cos(e6)*sin(e4)*(a1 + d4*cos(e2 + e3) + a3*sin(e2 + e3) + a2*sin(e2))) + (sin(e6)*(sin(e5)*(cos(e1)*cos(e2)*cos(e3) - 1.0*cos(e1)*sin(e2)*sin(e3)) + cos(e5)*(sin(e1)*sin(e4) + cos(e4)*(cos(e1)*cos(e2)*sin(e3) + cos(e1)*cos(e3)*sin(e2)))) - 1.0*cos(e6)*(cos(e4)*sin(e1) - 1.0*sin(e4)*(cos(e1)*cos(e2)*sin(e3) + cos(e1)*cos(e3)*sin(e2))))*(x6*(cos(e2 + e3)*cos(e5) - 1.0*sin(e2 + e3)*cos(e4)*sin(e5)) - 1.0*z6*(cos(e6)*(cos(e2 + e3)*sin(e5) + sin(e2 + e3)*cos(e4)*cos(e5)) - 1.0*sin(e2 + e3)*sin(e4)*sin(e6)) + cos(e4)*cos(e6)*(a3*cos(e2 + e3) - 1.0*d4*sin(e2 + e3)) - 1.0*cos(e5)*sin(e4)*sin(e6)*(a3*cos(e2 + e3) - 1.0*d4*sin(e2 + e3))) - 1.0*(cos(e5)*(cos(e1)*cos(e2)*cos(e3) - 1.0*cos(e1)*sin(e2)*sin(e3)) - 1.0*sin(e5)*(sin(e1)*sin(e4) + cos(e4)*(cos(e1)*cos(e2)*sin(e3) + cos(e1)*cos(e3)*sin(e2))))*(x6*(sin(e6)*(cos(e2 + e3)*sin(e5) + sin(e2 + e3)*cos(e4)*cos(e5)) + sin(e2 + e3)*cos(e6)*sin(e4)) + y6*(cos(e6)*(cos(e2 + e3)*sin(e5) + sin(e2 + e3)*cos(e4)*cos(e5)) - 1.0*sin(e2 + e3)*sin(e4)*sin(e6)) - 1.0*sin(e4)*sin(e5)*(a3*cos(e2 + e3) - 1.0*d4*sin(e2 + e3))) + (cos(e5)*(cos(e1)*cos(e2)*sin(e3) + cos(e1)*cos(e3)*sin(e2)) + cos(e4)*sin(e5)*(cos(e1)*cos(e2)*cos(e3) - 1.0*cos(e1)*sin(e2)*sin(e3)))*(x6*(sin(e6)*(sin(e2 + e3)*sin(e5) - 1.0*cos(e2 + e3)*cos(e4)*cos(e5)) - 1.0*cos(e2 + e3)*cos(e6)*sin(e4)) + y6*(cos(e6)*(sin(e2 + e3)*sin(e5) - 1.0*cos(e2 + e3)*cos(e4)*cos(e5)) + cos(e2 + e3)*sin(e4)*sin(e6)) - 1.0*sin(e4)*sin(e5)*(a1 + d4*cos(e2 + e3) + a3*sin(e2 + e3) + a2*sin(e2)))) + m6*((sin(e6)*(1.0*cos(e5)*(cos(e1)*sin(e4) - 1.0*cos(e4)*(cos(e2)*sin(e1)*sin(e3) + cos(e3)*sin(e1)*sin(e2))) - sin(e5)*(cos(e2)*cos(e3)*sin(e1) - 1.0*sin(e1)*sin(e2)*sin(e3))) - cos(e6)*(sin(e4)*(cos(e2)*sin(e1)*sin(e3) + cos(e3)*sin(e1)*sin(e2)) + cos(e1)*cos(e4)))*(x6*(sin(e2 + e3)*cos(e5) + cos(e2 + e3)*cos(e4)*sin(e5)) - 1.0*z6*(cos(e6)*(sin(e2 + e3)*sin(e5) - 1.0*cos(e2 + e3)*cos(e4)*cos(e5)) + cos(e2 + e3)*sin(e4)*sin(e6)) + cos(e4)*cos(e6)*(a1 + d4*cos(e2 + e3) + a3*sin(e2 + e3) + a2*sin(e2)) - 1.0*cos(e5)*sin(e4)*sin(e6)*(a1 + d4*cos(e2 + e3) + a3*sin(e2 + e3) + a2*sin(e2))) + 1.0*(sin(e5)*(cos(e1)*sin(e4) - 1.0*cos(e4)*(cos(e2)*sin(e1)*sin(e3) + cos(e3)*sin(e1)*sin(e2))) + cos(e5)*(cos(e2)*cos(e3)*sin(e1) - 1.0*sin(e1)*sin(e2)*sin(e3)))*(x6*(sin(e6)*(sin(e2 + e3)*sin(e5) - 1.0*cos(e2 + e3)*cos(e4)*cos(e5)) - 1.0*cos(e2 + e3)*cos(e6)*sin(e4)) + y6*(cos(e6)*(sin(e2 + e3)*sin(e5) - 1.0*cos(e2 + e3)*cos(e4)*cos(e5)) + cos(e2 + e3)*sin(e4)*sin(e6)) - 1.0*sin(e4)*sin(e5)*(a1 + d4*cos(e2 + e3) + a3*sin(e2 + e3) + a2*sin(e2))) + (cos(e6)*(1.0*cos(e5)*(cos(e1)*sin(e4) - 1.0*cos(e4)*(cos(e2)*sin(e1)*sin(e3) + cos(e3)*sin(e1)*sin(e2))) - sin(e5)*(cos(e2)*cos(e3)*sin(e1) - 1.0*sin(e1)*sin(e2)*sin(e3))) + 1.0*sin(e6)*(sin(e4)*(cos(e2)*sin(e1)*sin(e3) + cos(e3)*sin(e1)*sin(e2)) + cos(e1)*cos(e4)))*(z6*(sin(e6)*(sin(e2 + e3)*sin(e5) - 1.0*cos(e2 + e3)*cos(e4)*cos(e5)) - 1.0*cos(e2 + e3)*cos(e6)*sin(e4)) + y6*(sin(e2 + e3)*cos(e5) + cos(e2 + e3)*cos(e4)*sin(e5)) - 1.0*cos(e4)*sin(e6)*(a1 + d4*cos(e2 + e3) + a3*sin(e2 + e3) + a2*sin(e2)) - 1.0*cos(e5)*cos(e6)*sin(e4)*(a1 + d4*cos(e2 + e3) + a3*sin(e2 + e3) + a2*sin(e2))))*(z6*sin(e6)*(sin(e6)*(sin(e5)*(cos(e2)*sin(e1)*sin(e3) + cos(e3)*sin(e1)*sin(e2)) - 1.0*cos(e4)*cos(e5)*(cos(e2)*cos(e3)*sin(e1) - 1.0*sin(e1)*sin(e2)*sin(e3))) - 1.0*cos(e6)*sin(e4)*(cos(e2)*cos(e3)*sin(e1) - 1.0*sin(e1)*sin(e2)*sin(e3))) - 1.0*(cos(e5)*(cos(e2)*sin(e1)*sin(e3) + cos(e3)*sin(e1)*sin(e2)) + cos(e4)*sin(e5)*(cos(e2)*cos(e3)*sin(e1) - 1.0*sin(e1)*sin(e2)*sin(e3)))*(x6*cos(e6) - 1.0*y6*sin(e6)) + z6*cos(e6)*(cos(e6)*(sin(e5)*(cos(e2)*sin(e1)*sin(e3) + cos(e3)*sin(e1)*sin(e2)) - 1.0*cos(e4)*cos(e5)*(cos(e2)*cos(e3)*sin(e1) - 1.0*sin(e1)*sin(e2)*sin(e3))) + sin(e4)*sin(e6)*(cos(e2)*cos(e3)*sin(e1) - 1.0*sin(e1)*sin(e2)*sin(e3)))) + m6*(z6*sin(e6)*(sin(e6)*(sin(e5)*(cos(e2)*sin(e3) + cos(e3)*sin(e2)) + cos(e4)*cos(e5)*(sin(e2)*sin(e3) - 1.0*cos(e2)*cos(e3))) + cos(e6)*sin(e4)*(sin(e2)*sin(e3) - 1.0*cos(e2)*cos(e3))) - 1.0*(cos(e5)*(cos(e2)*sin(e3) + cos(e3)*sin(e2)) - 1.0*cos(e4)*sin(e5)*(sin(e2)*sin(e3) - 1.0*cos(e2)*cos(e3)))*(x6*cos(e6) - 1.0*y6*sin(e6)) + z6*cos(e6)*(cos(e6)*(sin(e5)*(cos(e2)*sin(e3) + cos(e3)*sin(e2)) + cos(e4)*cos(e5)*(sin(e2)*sin(e3) - 1.0*cos(e2)*cos(e3))) - 1.0*sin(e4)*sin(e6)*(sin(e2)*sin(e3) - 1.0*cos(e2)*cos(e3))))*(1.0*(sin(e6)*(sin(e5)*(cos(e2)*sin(e3) + cos(e3)*sin(e2)) + cos(e4)*cos(e5)*(sin(e2)*sin(e3) - 1.0*cos(e2)*cos(e3))) + cos(e6)*sin(e4)*(sin(e2)*sin(e3) - 1.0*cos(e2)*cos(e3)))*(x6*(cos(e2 + e3)*cos(e5) - 1.0*sin(e2 + e3)*cos(e4)*sin(e5)) - 1.0*z6*(cos(e6)*(cos(e2 + e3)*sin(e5) + sin(e2 + e3)*cos(e4)*cos(e5)) - 1.0*sin(e2 + e3)*sin(e4)*sin(e6)) + cos(e4)*cos(e6)*(a3*cos(e2 + e3) - 1.0*d4*sin(e2 + e3)) - 1.0*cos(e5)*sin(e4)*sin(e6)*(a3*cos(e2 + e3) - 1.0*d4*sin(e2 + e3))) + 1.0*(cos(e6)*(sin(e5)*(cos(e2)*sin(e3) + cos(e3)*sin(e2)) + cos(e4)*cos(e5)*(sin(e2)*sin(e3) - 1.0*cos(e2)*cos(e3))) - 1.0*sin(e4)*sin(e6)*(sin(e2)*sin(e3) - 1.0*cos(e2)*cos(e3)))*(z6*(sin(e6)*(cos(e2 + e3)*sin(e5) + sin(e2 + e3)*cos(e4)*cos(e5)) + sin(e2 + e3)*cos(e6)*sin(e4)) + y6*(cos(e2 + e3)*cos(e5) - 1.0*sin(e2 + e3)*cos(e4)*sin(e5)) - 1.0*cos(e4)*sin(e6)*(a3*cos(e2 + e3) - 1.0*d4*sin(e2 + e3)) - 1.0*cos(e5)*cos(e6)*sin(e4)*(a3*cos(e2 + e3) - 1.0*d4*sin(e2 + e3))) - (sin(e6)*(sin(e5)*(sin(e2)*sin(e3) - 1.0*cos(e2)*cos(e3)) - 1.0*cos(e4)*cos(e5)*(cos(e2)*sin(e3) + cos(e3)*sin(e2))) - 1.0*cos(e6)*sin(e4)*(cos(e2)*sin(e3) + cos(e3)*sin(e2)))*(x6*(sin(e2 + e3)*cos(e5) + cos(e2 + e3)*cos(e4)*sin(e5)) - 1.0*z6*(cos(e6)*(sin(e2 + e3)*sin(e5) - 1.0*cos(e2 + e3)*cos(e4)*cos(e5)) + cos(e2 + e3)*sin(e4)*sin(e6)) + cos(e4)*cos(e6)*(a1 + d4*cos(e2 + e3) + a3*sin(e2 + e3) + a2*sin(e2)) - 1.0*cos(e5)*sin(e4)*sin(e6)*(a1 + d4*cos(e2 + e3) + a3*sin(e2 + e3) + a2*sin(e2))) - (cos(e6)*(sin(e5)*(sin(e2)*sin(e3) - 1.0*cos(e2)*cos(e3)) - 1.0*cos(e4)*cos(e5)*(cos(e2)*sin(e3) + cos(e3)*sin(e2))) + sin(e4)*sin(e6)*(cos(e2)*sin(e3) + cos(e3)*sin(e2)))*(z6*(sin(e6)*(sin(e2 + e3)*sin(e5) - 1.0*cos(e2 + e3)*cos(e4)*cos(e5)) - 1.0*cos(e2 + e3)*cos(e6)*sin(e4)) + y6*(sin(e2 + e3)*cos(e5) + cos(e2 + e3)*cos(e4)*sin(e5)) - 1.0*cos(e4)*sin(e6)*(a1 + d4*cos(e2 + e3) + a3*sin(e2 + e3) + a2*sin(e2)) - 1.0*cos(e5)*cos(e6)*sin(e4)*(a1 + d4*cos(e2 + e3) + a3*sin(e2 + e3) + a2*sin(e2))) + 1.0*(cos(e5)*(sin(e2)*sin(e3) - 1.0*cos(e2)*cos(e3)) + cos(e4)*sin(e5)*(cos(e2)*sin(e3) + cos(e3)*sin(e2)))*(x6*(sin(e6)*(sin(e2 + e3)*sin(e5) - 1.0*cos(e2 + e3)*cos(e4)*cos(e5)) - 1.0*cos(e2 + e3)*cos(e6)*sin(e4)) + y6*(cos(e6)*(sin(e2 + e3)*sin(e5) - 1.0*cos(e2 + e3)*cos(e4)*cos(e5)) + cos(e2 + e3)*sin(e4)*sin(e6)) - 1.0*sin(e4)*sin(e5)*(a1 + d4*cos(e2 + e3) + a3*sin(e2 + e3) + a2*sin(e2))) - (cos(e5)*(cos(e2)*sin(e3) + cos(e3)*sin(e2)) - 1.0*cos(e4)*sin(e5)*(sin(e2)*sin(e3) - 1.0*cos(e2)*cos(e3)))*(x6*(sin(e6)*(cos(e2 + e3)*sin(e5) + sin(e2 + e3)*cos(e4)*cos(e5)) + sin(e2 + e3)*cos(e6)*sin(e4)) + y6*(cos(e6)*(cos(e2 + e3)*sin(e5) + sin(e2 + e3)*cos(e4)*cos(e5)) - 1.0*sin(e2 + e3)*sin(e4)*sin(e6)) - 1.0*sin(e4)*sin(e5)*(a3*cos(e2 + e3) - 1.0*d4*sin(e2 + e3)))) + 1.0*m5*(x5*(cos(e5)*(sin(e2)*sin(e3) - 1.0*cos(e2)*cos(e3)) + cos(e4)*sin(e5)*(cos(e2)*sin(e3) + cos(e3)*sin(e2))) - 1.0*y5*(sin(e5)*(sin(e2)*sin(e3) - 1.0*cos(e2)*cos(e3)) - 1.0*cos(e4)*cos(e5)*(cos(e2)*sin(e3) + cos(e3)*sin(e2))))*((cos(e5)*(cos(e2)*sin(e3) + cos(e3)*sin(e2)) - 1.0*cos(e4)*sin(e5)*(sin(e2)*sin(e3) - 1.0*cos(e2)*cos(e3)))*(z5*(sin(e2 + e3)*sin(e5) - 1.0*cos(e2 + e3)*cos(e4)*cos(e5)) + sin(e4)*sin(e5)*(a1 + d4*cos(e2 + e3) + a3*sin(e2 + e3) + a2*sin(e2)) + x5*cos(e2 + e3)*sin(e4)) - 1.0*(sin(e5)*(cos(e2)*sin(e3) + cos(e3)*sin(e2)) + cos(e4)*cos(e5)*(sin(e2)*sin(e3) - 1.0*cos(e2)*cos(e3)))*(z5*(sin(e2 + e3)*cos(e5) + cos(e2 + e3)*cos(e4)*sin(e5)) + cos(e5)*sin(e4)*(a1 + d4*cos(e2 + e3) + a3*sin(e2 + e3) + a2*sin(e2)) + y5*cos(e2 + e3)*sin(e4)) + sin(e4)*(sin(e2)*sin(e3) - 1.0*cos(e2)*cos(e3))*(cos(e4)*(a1 + d4*cos(e2 + e3) + a3*sin(e2 + e3) + a2*sin(e2)) + x5*(sin(e2 + e3)*cos(e5) + cos(e2 + e3)*cos(e4)*sin(e5)) - 1.0*y5*(sin(e2 + e3)*sin(e5) - 1.0*cos(e2 + e3)*cos(e4)*cos(e5)))) + m5*(1.0*y5*(sin(e5)*(cos(e2)*sin(e3) + cos(e3)*sin(e2)) + cos(e4)*cos(e5)*(sin(e2)*sin(e3) - 1.0*cos(e2)*cos(e3))) - x5*(cos(e5)*(cos(e2)*sin(e3) + cos(e3)*sin(e2)) - 1.0*cos(e4)*sin(e5)*(sin(e2)*sin(e3) - 1.0*cos(e2)*cos(e3))))*((sin(e5)*(sin(e2)*sin(e3) - 1.0*cos(e2)*cos(e3)) - 1.0*cos(e4)*cos(e5)*(cos(e2)*sin(e3) + cos(e3)*sin(e2)))*(z5*(sin(e2 + e3)*cos(e5) + cos(e2 + e3)*cos(e4)*sin(e5)) + cos(e5)*sin(e4)*(a1 + d4*cos(e2 + e3) + a3*sin(e2 + e3) + a2*sin(e2)) + y5*cos(e2 + e3)*sin(e4)) - 1.0*(cos(e5)*(sin(e2)*sin(e3) - 1.0*cos(e2)*cos(e3)) + cos(e4)*sin(e5)*(cos(e2)*sin(e3) + cos(e3)*sin(e2)))*(z5*(sin(e2 + e3)*sin(e5) - 1.0*cos(e2 + e3)*cos(e4)*cos(e5)) + sin(e4)*sin(e5)*(a1 + d4*cos(e2 + e3) + a3*sin(e2 + e3) + a2*sin(e2)) + x5*cos(e2 + e3)*sin(e4)) - 1.0*(sin(e5)*(cos(e2)*sin(e3) + cos(e3)*sin(e2)) + cos(e4)*cos(e5)*(sin(e2)*sin(e3) - 1.0*cos(e2)*cos(e3)))*(z5*(cos(e2 + e3)*cos(e5) - 1.0*sin(e2 + e3)*cos(e4)*sin(e5)) + cos(e5)*sin(e4)*(a3*cos(e2 + e3) - 1.0*d4*sin(e2 + e3)) - 1.0*y5*sin(e2 + e3)*sin(e4)) + (cos(e5)*(cos(e2)*sin(e3) + cos(e3)*sin(e2)) - 1.0*cos(e4)*sin(e5)*(sin(e2)*sin(e3) - 1.0*cos(e2)*cos(e3)))*(z5*(cos(e2 + e3)*sin(e5) + sin(e2 + e3)*cos(e4)*cos(e5)) - 1.0*x5*sin(e2 + e3)*sin(e4) + sin(e4)*sin(e5)*(a3*cos(e2 + e3) - 1.0*d4*sin(e2 + e3))) + sin(e4)*(sin(e2)*sin(e3) - 1.0*cos(e2)*cos(e3))*(cos(e4)*(a3*cos(e2 + e3) - 1.0*d4*sin(e2 + e3)) - 1.0*y5*(cos(e2 + e3)*sin(e5) + sin(e2 + e3)*cos(e4)*cos(e5)) + x5*(cos(e2 + e3)*cos(e5) - 1.0*sin(e2 + e3)*cos(e4)*sin(e5))) + sin(e4)*(cos(e2)*sin(e3) + cos(e3)*sin(e2))*(cos(e4)*(a1 + d4*cos(e2 + e3) + a3*sin(e2 + e3) + a2*sin(e2)) + x5*(sin(e2 + e3)*cos(e5) + cos(e2 + e3)*cos(e4)*sin(e5)) - 1.0*y5*(sin(e2 + e3)*sin(e5) - 1.0*cos(e2 + e3)*cos(e4)*cos(e5))))))/2 + (de2*(0.5*(cos(e2 + e3)*cos(e5) - 1.0*sin(e2 + e3)*cos(e4)*sin(e5))*(I5zy*cos(e4) - 1.0*I5xy*cos(e5)*sin(e4) + I5yy*sin(e4)*sin(e5)) - 0.5*(cos(e4)*sin(e6) + cos(e5)*cos(e6)*sin(e4))*(I6zx*(cos(e2 + e3)*cos(e5) - 1.0*sin(e2 + e3)*cos(e4)*sin(e5)) - 1.0*I6yx*(sin(e6)*(cos(e2 + e3)*sin(e5) + sin(e2 + e3)*cos(e4)*cos(e5)) + sin(e2 + e3)*cos(e6)*sin(e4)) + I6xx*(cos(e6)*(cos(e2 + e3)*sin(e5) + sin(e2 + e3)*cos(e4)*cos(e5)) - 1.0*sin(e2 + e3)*sin(e4)*sin(e6))) + 0.5*(sin(e6)*(cos(e2 + e3)*sin(e5) + sin(e2 + e3)*cos(e4)*cos(e5)) + sin(e2 + e3)*cos(e6)*sin(e4))*(I6yy*(cos(e4)*cos(e6) - 1.0*cos(e5)*sin(e4)*sin(e6)) + I6xy*(cos(e4)*sin(e6) + cos(e5)*cos(e6)*sin(e4)) - 1.0*I6zy*sin(e4)*sin(e5)) - 0.5*cos(e4)*(I4zy*cos(e2 + e3) + I4xy*sin(e2 + e3)*cos(e4) - 1.0*I4yy*sin(e2 + e3)*sin(e4)) - 0.5*(cos(e2 + e3)*cos(e5) - 1.0*sin(e2 + e3)*cos(e4)*sin(e5))*(I6yz*(cos(e4)*cos(e6) - 1.0*cos(e5)*sin(e4)*sin(e6)) + I6xz*(cos(e4)*sin(e6) + cos(e5)*cos(e6)*sin(e4)) - 1.0*I6zz*sin(e4)*sin(e5)) + 0.5*I3yz*cos(e2 + e3) + 0.5*I3zy*cos(e2 + e3) - 0.5*sin(e4)*(I4zx*cos(e2 + e3) + I4xx*sin(e2 + e3)*cos(e4) - 1.0*I4yx*sin(e2 + e3)*sin(e4)) - 0.5*cos(e2 + e3)*(I4yz*cos(e4) + I4xz*sin(e4)) + 0.5*I3xz*sin(e2 + e3) + 0.5*I3zx*sin(e2 + e3) - 0.5*(cos(e4)*cos(e6) - 1.0*cos(e5)*sin(e4)*sin(e6))*(I6zy*(cos(e2 + e3)*cos(e5) - 1.0*sin(e2 + e3)*cos(e4)*sin(e5)) - 1.0*I6yy*(sin(e6)*(cos(e2 + e3)*sin(e5) + sin(e2 + e3)*cos(e4)*cos(e5)) + sin(e2 + e3)*cos(e6)*sin(e4)) + I6xy*(cos(e6)*(cos(e2 + e3)*sin(e5) + sin(e2 + e3)*cos(e4)*cos(e5)) - 1.0*sin(e2 + e3)*sin(e4)*sin(e6))) - 0.5*(cos(e6)*(cos(e2 + e3)*sin(e5) + sin(e2 + e3)*cos(e4)*cos(e5)) - 1.0*sin(e2 + e3)*sin(e4)*sin(e6))*(I6yx*(cos(e4)*cos(e6) - 1.0*cos(e5)*sin(e4)*sin(e6)) + I6xx*(cos(e4)*sin(e6) + cos(e5)*cos(e6)*sin(e4)) - 1.0*I6zx*sin(e4)*sin(e5)) + 0.5*cos(e4)*(I5xz*(cos(e2 + e3)*sin(e5) + sin(e2 + e3)*cos(e4)*cos(e5)) + I5yz*(cos(e2 + e3)*cos(e5) - 1.0*sin(e2 + e3)*cos(e4)*sin(e5)) + I5zz*sin(e2 + e3)*sin(e4)) + 0.5*(cos(e2 + e3)*sin(e5) + sin(e2 + e3)*cos(e4)*cos(e5))*(I5zx*cos(e4) - 1.0*I5xx*cos(e5)*sin(e4) + I5yx*sin(e4)*sin(e5)) + 1.0*m4*((cos(e2)*cos(e3)*sin(e1) - 1.0*sin(e1)*sin(e2)*sin(e3))*(a3 + a2*cos(e3) + x4*cos(e4) - 1.0*y4*sin(e4)) - 1.0*(sin(e4)*(cos(e2)*sin(e1)*sin(e3) + cos(e3)*sin(e1)*sin(e2)) + cos(e1)*cos(e4))*(z4*sin(e4) + sin(e4)*(d4 - 1.0*a2*sin(e3))) + (z4*cos(e4) + cos(e4)*(d4 - 1.0*a2*sin(e3)))*(cos(e1)*sin(e4) - 1.0*cos(e4)*(cos(e2)*sin(e1)*sin(e3) + cos(e3)*sin(e1)*sin(e2))))*((cos(e1)*sin(e4) - 1.0*cos(e4)*(cos(e2)*sin(e1)*sin(e3) + cos(e3)*sin(e1)*sin(e2)))*(y4*cos(e2 + e3) - 1.0*sin(e4)*(a3*cos(e2 + e3) - 1.0*d4*sin(e2 + e3)) + z4*sin(e2 + e3)*sin(e4)) + (cos(e2)*sin(e1)*sin(e3) + cos(e3)*sin(e1)*sin(e2))*(y4*cos(e2 + e3)*cos(e4) + x4*cos(e2 + e3)*sin(e4)) + (cos(e2)*cos(e3)*sin(e1) - 1.0*sin(e1)*sin(e2)*sin(e3))*(y4*sin(e2 + e3)*cos(e4) + x4*sin(e2 + e3)*sin(e4)) - 1.0*(sin(e4)*(cos(e2)*sin(e1)*sin(e3) + cos(e3)*sin(e1)*sin(e2)) + cos(e1)*cos(e4))*(x4*cos(e2 + e3) + cos(e4)*(a3*cos(e2 + e3) - 1.0*d4*sin(e2 + e3)) - 1.0*z4*sin(e2 + e3)*cos(e4)) + cos(e4)*(cos(e2)*cos(e3)*sin(e1) - 1.0*sin(e1)*sin(e2)*sin(e3))*(sin(e4)*(a1 + d4*cos(e2 + e3) + a3*sin(e2 + e3) + a2*sin(e2)) - 1.0*y4*sin(e2 + e3) + z4*cos(e2 + e3)*sin(e4)) - 1.0*sin(e4)*(cos(e2)*cos(e3)*sin(e1) - 1.0*sin(e1)*sin(e2)*sin(e3))*(cos(e4)*(a1 + d4*cos(e2 + e3) + a3*sin(e2 + e3) + a2*sin(e2)) + x4*sin(e2 + e3) + z4*cos(e2 + e3)*cos(e4))) - 0.5*sin(e2 + e3)*cos(e4)*(I4yx*cos(e4) + I4xx*sin(e4)) + m5*(1.0*(sin(e4)*(cos(e2)*sin(e1)*sin(e3) + cos(e3)*sin(e1)*sin(e2)) + cos(e1)*cos(e4))*(sin(e4)*(d4 - 1.0*a2*sin(e3)) + y5*cos(e5)*sin(e4) + x5*sin(e4)*sin(e5)) + (1.0*cos(e5)*(cos(e1)*sin(e4) - 1.0*cos(e4)*(cos(e2)*sin(e1)*sin(e3) + cos(e3)*sin(e1)*sin(e2))) - sin(e5)*(cos(e2)*cos(e3)*sin(e1) - 1.0*sin(e1)*sin(e2)*sin(e3)))*(sin(e5)*(a3 + a2*cos(e3)) - 1.0*y5*cos(e4) + z5*sin(e4)*sin(e5) - 1.0*cos(e4)*cos(e5)*(d4 - 1.0*a2*sin(e3))) - (sin(e5)*(cos(e1)*sin(e4) - 1.0*cos(e4)*(cos(e2)*sin(e1)*sin(e3) + cos(e3)*sin(e1)*sin(e2))) + cos(e5)*(cos(e2)*cos(e3)*sin(e1) - 1.0*sin(e1)*sin(e2)*sin(e3)))*(cos(e5)*(a3 + a2*cos(e3)) + x5*cos(e4) + z5*cos(e5)*sin(e4) + cos(e4)*sin(e5)*(d4 - 1.0*a2*sin(e3))))*((sin(e5)*(cos(e1)*sin(e4) - 1.0*cos(e4)*(cos(e2)*sin(e1)*sin(e3) + cos(e3)*sin(e1)*sin(e2))) + cos(e5)*(cos(e2)*cos(e3)*sin(e1) - 1.0*sin(e1)*sin(e2)*sin(e3)))*(z5*(cos(e2 + e3)*sin(e5) + sin(e2 + e3)*cos(e4)*cos(e5)) - 1.0*x5*sin(e2 + e3)*sin(e4) + sin(e4)*sin(e5)*(a3*cos(e2 + e3) - 1.0*d4*sin(e2 + e3))) + (sin(e4)*(cos(e2)*sin(e1)*sin(e3) + cos(e3)*sin(e1)*sin(e2)) + cos(e1)*cos(e4))*(cos(e4)*(a3*cos(e2 + e3) - 1.0*d4*sin(e2 + e3)) - 1.0*y5*(cos(e2 + e3)*sin(e5) + sin(e2 + e3)*cos(e4)*cos(e5)) + x5*(cos(e2 + e3)*cos(e5) - 1.0*sin(e2 + e3)*cos(e4)*sin(e5))) + 1.0*(1.0*cos(e5)*(cos(e1)*sin(e4) - 1.0*cos(e4)*(cos(e2)*sin(e1)*sin(e3) + cos(e3)*sin(e1)*sin(e2))) - sin(e5)*(cos(e2)*cos(e3)*sin(e1) - 1.0*sin(e1)*sin(e2)*sin(e3)))*(z5*(cos(e2 + e3)*cos(e5) - 1.0*sin(e2 + e3)*cos(e4)*sin(e5)) + cos(e5)*sin(e4)*(a3*cos(e2 + e3) - 1.0*d4*sin(e2 + e3)) - 1.0*y5*sin(e2 + e3)*sin(e4)) + (sin(e5)*(cos(e2)*sin(e1)*sin(e3) + cos(e3)*sin(e1)*sin(e2)) - 1.0*cos(e4)*cos(e5)*(cos(e2)*cos(e3)*sin(e1) - 1.0*sin(e1)*sin(e2)*sin(e3)))*(z5*(sin(e2 + e3)*cos(e5) + cos(e2 + e3)*cos(e4)*sin(e5)) + cos(e5)*sin(e4)*(a1 + d4*cos(e2 + e3) + a3*sin(e2 + e3) + a2*sin(e2)) + y5*cos(e2 + e3)*sin(e4)) - 1.0*(cos(e5)*(cos(e2)*sin(e1)*sin(e3) + cos(e3)*sin(e1)*sin(e2)) + cos(e4)*sin(e5)*(cos(e2)*cos(e3)*sin(e1) - 1.0*sin(e1)*sin(e2)*sin(e3)))*(z5*(sin(e2 + e3)*sin(e5) - 1.0*cos(e2 + e3)*cos(e4)*cos(e5)) + sin(e4)*sin(e5)*(a1 + d4*cos(e2 + e3) + a3*sin(e2 + e3) + a2*sin(e2)) + x5*cos(e2 + e3)*sin(e4)) + sin(e4)*(cos(e2)*cos(e3)*sin(e1) - 1.0*sin(e1)*sin(e2)*sin(e3))*(cos(e4)*(a1 + d4*cos(e2 + e3) + a3*sin(e2 + e3) + a2*sin(e2)) + x5*(sin(e2 + e3)*cos(e5) + cos(e2 + e3)*cos(e4)*sin(e5)) - 1.0*y5*(sin(e2 + e3)*sin(e5) - 1.0*cos(e2 + e3)*cos(e4)*cos(e5)))) - 1.0*m5*((cos(e4)*sin(e1) - 1.0*sin(e4)*(cos(e1)*cos(e2)*sin(e3) + cos(e1)*cos(e3)*sin(e2)))*(sin(e4)*(d4 - 1.0*a2*sin(e3)) + y5*cos(e5)*sin(e4) + x5*sin(e4)*sin(e5)) + (cos(e5)*(cos(e1)*cos(e2)*cos(e3) - 1.0*cos(e1)*sin(e2)*sin(e3)) - 1.0*sin(e5)*(sin(e1)*sin(e4) + cos(e4)*(cos(e1)*cos(e2)*sin(e3) + cos(e1)*cos(e3)*sin(e2))))*(cos(e5)*(a3 + a2*cos(e3)) + x5*cos(e4) + z5*cos(e5)*sin(e4) + cos(e4)*sin(e5)*(d4 - 1.0*a2*sin(e3))) + (sin(e5)*(cos(e1)*cos(e2)*cos(e3) - 1.0*cos(e1)*sin(e2)*sin(e3)) + cos(e5)*(sin(e1)*sin(e4) + cos(e4)*(cos(e1)*cos(e2)*sin(e3) + cos(e1)*cos(e3)*sin(e2))))*(sin(e5)*(a3 + a2*cos(e3)) - 1.0*y5*cos(e4) + z5*sin(e4)*sin(e5) - 1.0*cos(e4)*cos(e5)*(d4 - 1.0*a2*sin(e3))))*(1.0*(sin(e5)*(cos(e1)*cos(e2)*sin(e3) + cos(e1)*cos(e3)*sin(e2)) - 1.0*cos(e4)*cos(e5)*(cos(e1)*cos(e2)*cos(e3) - 1.0*cos(e1)*sin(e2)*sin(e3)))*(z5*(sin(e2 + e3)*cos(e5) + cos(e2 + e3)*cos(e4)*sin(e5)) + cos(e5)*sin(e4)*(a1 + d4*cos(e2 + e3) + a3*sin(e2 + e3) + a2*sin(e2)) + y5*cos(e2 + e3)*sin(e4)) - (cos(e5)*(cos(e1)*cos(e2)*sin(e3) + cos(e1)*cos(e3)*sin(e2)) + cos(e4)*sin(e5)*(cos(e1)*cos(e2)*cos(e3) - 1.0*cos(e1)*sin(e2)*sin(e3)))*(z5*(sin(e2 + e3)*sin(e5) - 1.0*cos(e2 + e3)*cos(e4)*cos(e5)) + sin(e4)*sin(e5)*(a1 + d4*cos(e2 + e3) + a3*sin(e2 + e3) + a2*sin(e2)) + x5*cos(e2 + e3)*sin(e4)) - (cos(e4)*sin(e1) - 1.0*sin(e4)*(cos(e1)*cos(e2)*sin(e3) + cos(e1)*cos(e3)*sin(e2)))*(cos(e4)*(a3*cos(e2 + e3) - 1.0*d4*sin(e2 + e3)) - 1.0*y5*(cos(e2 + e3)*sin(e5) + sin(e2 + e3)*cos(e4)*cos(e5)) + x5*(cos(e2 + e3)*cos(e5) - 1.0*sin(e2 + e3)*cos(e4)*sin(e5))) - (sin(e5)*(cos(e1)*cos(e2)*cos(e3) - 1.0*cos(e1)*sin(e2)*sin(e3)) + cos(e5)*(sin(e1)*sin(e4) + cos(e4)*(cos(e1)*cos(e2)*sin(e3) + cos(e1)*cos(e3)*sin(e2))))*(z5*(cos(e2 + e3)*cos(e5) - 1.0*sin(e2 + e3)*cos(e4)*sin(e5)) + cos(e5)*sin(e4)*(a3*cos(e2 + e3) - 1.0*d4*sin(e2 + e3)) - 1.0*y5*sin(e2 + e3)*sin(e4)) + 1.0*(cos(e5)*(cos(e1)*cos(e2)*cos(e3) - 1.0*cos(e1)*sin(e2)*sin(e3)) - 1.0*sin(e5)*(sin(e1)*sin(e4) + cos(e4)*(cos(e1)*cos(e2)*sin(e3) + cos(e1)*cos(e3)*sin(e2))))*(z5*(cos(e2 + e3)*sin(e5) + sin(e2 + e3)*cos(e4)*cos(e5)) - 1.0*x5*sin(e2 + e3)*sin(e4) + sin(e4)*sin(e5)*(a3*cos(e2 + e3) - 1.0*d4*sin(e2 + e3))) + 1.0*sin(e4)*(cos(e1)*cos(e2)*cos(e3) - 1.0*cos(e1)*sin(e2)*sin(e3))*(cos(e4)*(a1 + d4*cos(e2 + e3) + a3*sin(e2 + e3) + a2*sin(e2)) + x5*(sin(e2 + e3)*cos(e5) + cos(e2 + e3)*cos(e4)*sin(e5)) - 1.0*y5*(sin(e2 + e3)*sin(e5) - 1.0*cos(e2 + e3)*cos(e4)*cos(e5)))) + 1.0*m6*((sin(e6)*(sin(e5)*(cos(e1)*cos(e2)*cos(e3) - 1.0*cos(e1)*sin(e2)*sin(e3)) + cos(e5)*(sin(e1)*sin(e4) + cos(e4)*(cos(e1)*cos(e2)*sin(e3) + cos(e1)*cos(e3)*sin(e2)))) - 1.0*cos(e6)*(cos(e4)*sin(e1) - 1.0*sin(e4)*(cos(e1)*cos(e2)*sin(e3) + cos(e1)*cos(e3)*sin(e2))))*(x6*(sin(e2 + e3)*cos(e5) + cos(e2 + e3)*cos(e4)*sin(e5)) - 1.0*z6*(cos(e6)*(sin(e2 + e3)*sin(e5) - 1.0*cos(e2 + e3)*cos(e4)*cos(e5)) + cos(e2 + e3)*sin(e4)*sin(e6)) + cos(e4)*cos(e6)*(a1 + d4*cos(e2 + e3) + a3*sin(e2 + e3) + a2*sin(e2)) - 1.0*cos(e5)*sin(e4)*sin(e6)*(a1 + d4*cos(e2 + e3) + a3*sin(e2 + e3) + a2*sin(e2))) + (sin(e6)*(cos(e4)*sin(e1) - 1.0*sin(e4)*(cos(e1)*cos(e2)*sin(e3) + cos(e1)*cos(e3)*sin(e2))) + cos(e6)*(sin(e5)*(cos(e1)*cos(e2)*cos(e3) - 1.0*cos(e1)*sin(e2)*sin(e3)) + cos(e5)*(sin(e1)*sin(e4) + cos(e4)*(cos(e1)*cos(e2)*sin(e3) + cos(e1)*cos(e3)*sin(e2)))))*(z6*(sin(e6)*(sin(e2 + e3)*sin(e5) - 1.0*cos(e2 + e3)*cos(e4)*cos(e5)) - 1.0*cos(e2 + e3)*cos(e6)*sin(e4)) + y6*(sin(e2 + e3)*cos(e5) + cos(e2 + e3)*cos(e4)*sin(e5)) - 1.0*cos(e4)*sin(e6)*(a1 + d4*cos(e2 + e3) + a3*sin(e2 + e3) + a2*sin(e2)) - 1.0*cos(e5)*cos(e6)*sin(e4)*(a1 + d4*cos(e2 + e3) + a3*sin(e2 + e3) + a2*sin(e2))) - 1.0*(cos(e5)*(cos(e1)*cos(e2)*cos(e3) - 1.0*cos(e1)*sin(e2)*sin(e3)) - 1.0*sin(e5)*(sin(e1)*sin(e4) + cos(e4)*(cos(e1)*cos(e2)*sin(e3) + cos(e1)*cos(e3)*sin(e2))))*(x6*(sin(e6)*(sin(e2 + e3)*sin(e5) - 1.0*cos(e2 + e3)*cos(e4)*cos(e5)) - 1.0*cos(e2 + e3)*cos(e6)*sin(e4)) + y6*(cos(e6)*(sin(e2 + e3)*sin(e5) - 1.0*cos(e2 + e3)*cos(e4)*cos(e5)) + cos(e2 + e3)*sin(e4)*sin(e6)) - 1.0*sin(e4)*sin(e5)*(a1 + d4*cos(e2 + e3) + a3*sin(e2 + e3) + a2*sin(e2))))*((cos(e5)*(cos(e1)*cos(e2)*cos(e3) - 1.0*cos(e1)*sin(e2)*sin(e3)) - 1.0*sin(e5)*(sin(e1)*sin(e4) + cos(e4)*(cos(e1)*cos(e2)*sin(e3) + cos(e1)*cos(e3)*sin(e2))))*(a2*cos(e5)*sin(e3) + a2*cos(e3)*cos(e4)*sin(e5)) - 1.0*(cos(e6)*(sin(e5)*(cos(e1)*cos(e2)*sin(e3) + cos(e1)*cos(e3)*sin(e2)) - 1.0*cos(e4)*cos(e5)*(cos(e1)*cos(e2)*cos(e3) - 1.0*cos(e1)*sin(e2)*sin(e3))) + sin(e4)*sin(e6)*(cos(e1)*cos(e2)*cos(e3) - 1.0*cos(e1)*sin(e2)*sin(e3)))*(z6*(cos(e4)*cos(e6) - 1.0*cos(e5)*sin(e4)*sin(e6)) - 1.0*cos(e6)*(sin(e5)*(a3 + a2*cos(e3)) - 1.0*cos(e4)*cos(e5)*(d4 - 1.0*a2*sin(e3))) + y6*sin(e4)*sin(e5) - 1.0*sin(e4)*sin(e6)*(d4 - 1.0*a2*sin(e3))) + (cos(e6)*(a2*sin(e3)*sin(e5) - 1.0*a2*cos(e3)*cos(e4)*cos(e5)) + a2*cos(e3)*sin(e4)*sin(e6))*(sin(e6)*(cos(e4)*sin(e1) - 1.0*sin(e4)*(cos(e1)*cos(e2)*sin(e3) + cos(e1)*cos(e3)*sin(e2))) + cos(e6)*(sin(e5)*(cos(e1)*cos(e2)*cos(e3) - 1.0*cos(e1)*sin(e2)*sin(e3)) + cos(e5)*(sin(e1)*sin(e4) + cos(e4)*(cos(e1)*cos(e2)*sin(e3) + cos(e1)*cos(e3)*sin(e2))))) + (sin(e6)*(a2*sin(e3)*sin(e5) - 1.0*a2*cos(e3)*cos(e4)*cos(e5)) - 1.0*a2*cos(e3)*cos(e6)*sin(e4))*(sin(e6)*(sin(e5)*(cos(e1)*cos(e2)*cos(e3) - 1.0*cos(e1)*sin(e2)*sin(e3)) + cos(e5)*(sin(e1)*sin(e4) + cos(e4)*(cos(e1)*cos(e2)*sin(e3) + cos(e1)*cos(e3)*sin(e2)))) - 1.0*cos(e6)*(cos(e4)*sin(e1) - 1.0*sin(e4)*(cos(e1)*cos(e2)*sin(e3) + cos(e1)*cos(e3)*sin(e2)))) + (cos(e5)*(cos(e1)*cos(e2)*sin(e3) + cos(e1)*cos(e3)*sin(e2)) + cos(e4)*sin(e5)*(cos(e1)*cos(e2)*cos(e3) - 1.0*cos(e1)*sin(e2)*sin(e3)))*(x6*(cos(e4)*cos(e6) - 1.0*cos(e5)*sin(e4)*sin(e6)) - 1.0*y6*(cos(e4)*sin(e6) + cos(e5)*cos(e6)*sin(e4)) + cos(e5)*(a3 + a2*cos(e3)) + cos(e4)*sin(e5)*(d4 - 1.0*a2*sin(e3))) - 1.0*(sin(e6)*(sin(e5)*(cos(e1)*cos(e2)*sin(e3) + cos(e1)*cos(e3)*sin(e2)) - 1.0*cos(e4)*cos(e5)*(cos(e1)*cos(e2)*cos(e3) - 1.0*cos(e1)*sin(e2)*sin(e3))) - 1.0*cos(e6)*sin(e4)*(cos(e1)*cos(e2)*cos(e3) - 1.0*cos(e1)*sin(e2)*sin(e3)))*(z6*(cos(e4)*sin(e6) + cos(e5)*cos(e6)*sin(e4)) - 1.0*sin(e6)*(sin(e5)*(a3 + a2*cos(e3)) - 1.0*cos(e4)*cos(e5)*(d4 - 1.0*a2*sin(e3))) + x6*sin(e4)*sin(e5) + cos(e6)*sin(e4)*(d4 - 1.0*a2*sin(e3)))) + 0.5*sin(e2 + e3)*sin(e4)*(I4yy*cos(e4) + I4xy*sin(e4)) + 1.0*m4*((cos(e4)*sin(e1) - 1.0*sin(e4)*(cos(e1)*cos(e2)*sin(e3) + cos(e1)*cos(e3)*sin(e2)))*(z4*sin(e4) + sin(e4)*(d4 - 1.0*a2*sin(e3))) + (cos(e1)*cos(e2)*cos(e3) - 1.0*cos(e1)*sin(e2)*sin(e3))*(a3 + a2*cos(e3) + x4*cos(e4) - 1.0*y4*sin(e4)) - 1.0*(sin(e1)*sin(e4) + cos(e4)*(cos(e1)*cos(e2)*sin(e3) + cos(e1)*cos(e3)*sin(e2)))*(z4*cos(e4) + cos(e4)*(d4 - 1.0*a2*sin(e3))))*((y4*cos(e2 + e3)*cos(e4) + x4*cos(e2 + e3)*sin(e4))*(cos(e1)*cos(e2)*sin(e3) + cos(e1)*cos(e3)*sin(e2)) + (cos(e1)*cos(e2)*cos(e3) - 1.0*cos(e1)*sin(e2)*sin(e3))*(y4*sin(e2 + e3)*cos(e4) + x4*sin(e2 + e3)*sin(e4)) - 1.0*(sin(e1)*sin(e4) + cos(e4)*(cos(e1)*cos(e2)*sin(e3) + cos(e1)*cos(e3)*sin(e2)))*(y4*cos(e2 + e3) - 1.0*sin(e4)*(a3*cos(e2 + e3) - 1.0*d4*sin(e2 + e3)) + z4*sin(e2 + e3)*sin(e4)) + (cos(e4)*sin(e1) - 1.0*sin(e4)*(cos(e1)*cos(e2)*sin(e3) + cos(e1)*cos(e3)*sin(e2)))*(x4*cos(e2 + e3) + cos(e4)*(a3*cos(e2 + e3) - 1.0*d4*sin(e2 + e3)) - 1.0*z4*sin(e2 + e3)*cos(e4)) - 1.0*sin(e4)*(cos(e1)*cos(e2)*cos(e3) - 1.0*cos(e1)*sin(e2)*sin(e3))*(cos(e4)*(a1 + d4*cos(e2 + e3) + a3*sin(e2 + e3) + a2*sin(e2)) + x4*sin(e2 + e3) + z4*cos(e2 + e3)*cos(e4)) + cos(e4)*(cos(e1)*cos(e2)*cos(e3) - 1.0*cos(e1)*sin(e2)*sin(e3))*(sin(e4)*(a1 + d4*cos(e2 + e3) + a3*sin(e2 + e3) + a2*sin(e2)) - 1.0*y4*sin(e2 + e3) + z4*cos(e2 + e3)*sin(e4))) + 1.0*m6*((sin(e6)*(sin(e5)*(cos(e2)*sin(e3) + cos(e3)*sin(e2)) + cos(e4)*cos(e5)*(sin(e2)*sin(e3) - 1.0*cos(e2)*cos(e3))) + cos(e6)*sin(e4)*(sin(e2)*sin(e3) - 1.0*cos(e2)*cos(e3)))*(x6*(sin(e2 + e3)*cos(e5) + cos(e2 + e3)*cos(e4)*sin(e5)) - 1.0*z6*(cos(e6)*(sin(e2 + e3)*sin(e5) - 1.0*cos(e2 + e3)*cos(e4)*cos(e5)) + cos(e2 + e3)*sin(e4)*sin(e6)) + cos(e4)*cos(e6)*(a1 + d4*cos(e2 + e3) + a3*sin(e2 + e3) + a2*sin(e2)) - 1.0*cos(e5)*sin(e4)*sin(e6)*(a1 + d4*cos(e2 + e3) + a3*sin(e2 + e3) + a2*sin(e2))) + (cos(e6)*(sin(e5)*(cos(e2)*sin(e3) + cos(e3)*sin(e2)) + cos(e4)*cos(e5)*(sin(e2)*sin(e3) - 1.0*cos(e2)*cos(e3))) - 1.0*sin(e4)*sin(e6)*(sin(e2)*sin(e3) - 1.0*cos(e2)*cos(e3)))*(z6*(sin(e6)*(sin(e2 + e3)*sin(e5) - 1.0*cos(e2 + e3)*cos(e4)*cos(e5)) - 1.0*cos(e2 + e3)*cos(e6)*sin(e4)) + y6*(sin(e2 + e3)*cos(e5) + cos(e2 + e3)*cos(e4)*sin(e5)) - 1.0*cos(e4)*sin(e6)*(a1 + d4*cos(e2 + e3) + a3*sin(e2 + e3) + a2*sin(e2)) - 1.0*cos(e5)*cos(e6)*sin(e4)*(a1 + d4*cos(e2 + e3) + a3*sin(e2 + e3) + a2*sin(e2))) - 1.0*(cos(e5)*(cos(e2)*sin(e3) + cos(e3)*sin(e2)) - 1.0*cos(e4)*sin(e5)*(sin(e2)*sin(e3) - 1.0*cos(e2)*cos(e3)))*(x6*(sin(e6)*(sin(e2 + e3)*sin(e5) - 1.0*cos(e2 + e3)*cos(e4)*cos(e5)) - 1.0*cos(e2 + e3)*cos(e6)*sin(e4)) + y6*(cos(e6)*(sin(e2 + e3)*sin(e5) - 1.0*cos(e2 + e3)*cos(e4)*cos(e5)) + cos(e2 + e3)*sin(e4)*sin(e6)) - 1.0*sin(e4)*sin(e5)*(a1 + d4*cos(e2 + e3) + a3*sin(e2 + e3) + a2*sin(e2))))*((cos(e5)*(cos(e2)*sin(e3) + cos(e3)*sin(e2)) - 1.0*cos(e4)*sin(e5)*(sin(e2)*sin(e3) - 1.0*cos(e2)*cos(e3)))*(a2*cos(e5)*sin(e3) + a2*cos(e3)*cos(e4)*sin(e5)) - 1.0*(sin(e6)*(sin(e5)*(sin(e2)*sin(e3) - 1.0*cos(e2)*cos(e3)) - 1.0*cos(e4)*cos(e5)*(cos(e2)*sin(e3) + cos(e3)*sin(e2))) - 1.0*cos(e6)*sin(e4)*(cos(e2)*sin(e3) + cos(e3)*sin(e2)))*(z6*(cos(e4)*sin(e6) + cos(e5)*cos(e6)*sin(e4)) - 1.0*sin(e6)*(sin(e5)*(a3 + a2*cos(e3)) - 1.0*cos(e4)*cos(e5)*(d4 - 1.0*a2*sin(e3))) + x6*sin(e4)*sin(e5) + cos(e6)*sin(e4)*(d4 - 1.0*a2*sin(e3))) + (sin(e6)*(a2*sin(e3)*sin(e5) - 1.0*a2*cos(e3)*cos(e4)*cos(e5)) - 1.0*a2*cos(e3)*cos(e6)*sin(e4))*(sin(e6)*(sin(e5)*(cos(e2)*sin(e3) + cos(e3)*sin(e2)) + cos(e4)*cos(e5)*(sin(e2)*sin(e3) - 1.0*cos(e2)*cos(e3))) + cos(e6)*sin(e4)*(sin(e2)*sin(e3) - 1.0*cos(e2)*cos(e3))) + (cos(e6)*(a2*sin(e3)*sin(e5) - 1.0*a2*cos(e3)*cos(e4)*cos(e5)) + a2*cos(e3)*sin(e4)*sin(e6))*(cos(e6)*(sin(e5)*(cos(e2)*sin(e3) + cos(e3)*sin(e2)) + cos(e4)*cos(e5)*(sin(e2)*sin(e3) - 1.0*cos(e2)*cos(e3))) - 1.0*sin(e4)*sin(e6)*(sin(e2)*sin(e3) - 1.0*cos(e2)*cos(e3))) - 1.0*(cos(e6)*(sin(e5)*(sin(e2)*sin(e3) - 1.0*cos(e2)*cos(e3)) - 1.0*cos(e4)*cos(e5)*(cos(e2)*sin(e3) + cos(e3)*sin(e2))) + sin(e4)*sin(e6)*(cos(e2)*sin(e3) + cos(e3)*sin(e2)))*(z6*(cos(e4)*cos(e6) - 1.0*cos(e5)*sin(e4)*sin(e6)) - 1.0*cos(e6)*(sin(e5)*(a3 + a2*cos(e3)) - 1.0*cos(e4)*cos(e5)*(d4 - 1.0*a2*sin(e3))) + y6*sin(e4)*sin(e5) - 1.0*sin(e4)*sin(e6)*(d4 - 1.0*a2*sin(e3))) + (cos(e5)*(sin(e2)*sin(e3) - 1.0*cos(e2)*cos(e3)) + cos(e4)*sin(e5)*(cos(e2)*sin(e3) + cos(e3)*sin(e2)))*(x6*(cos(e4)*cos(e6) - 1.0*cos(e5)*sin(e4)*sin(e6)) - 1.0*y6*(cos(e4)*sin(e6) + cos(e5)*cos(e6)*sin(e4)) + cos(e5)*(a3 + a2*cos(e3)) + cos(e4)*sin(e5)*(d4 - 1.0*a2*sin(e3)))) + 1.0*m4*((sin(e4)*(cos(e2)*sin(e1)*sin(e3) + cos(e3)*sin(e1)*sin(e2)) + cos(e1)*cos(e4))*(cos(e4)*(a1 + d4*cos(e2 + e3) + a3*sin(e2 + e3) + a2*sin(e2)) + x4*sin(e2 + e3) + z4*cos(e2 + e3)*cos(e4)) + (cos(e2)*cos(e3)*sin(e1) - 1.0*sin(e1)*sin(e2)*sin(e3))*(y4*cos(e2 + e3)*cos(e4) + x4*cos(e2 + e3)*sin(e4)) + (cos(e1)*sin(e4) - 1.0*cos(e4)*(cos(e2)*sin(e1)*sin(e3) + cos(e3)*sin(e1)*sin(e2)))*(sin(e4)*(a1 + d4*cos(e2 + e3) + a3*sin(e2 + e3) + a2*sin(e2)) - 1.0*y4*sin(e2 + e3) + z4*cos(e2 + e3)*sin(e4)))*((cos(e2)*sin(e1)*sin(e3) + cos(e3)*sin(e1)*sin(e2))*(a3 + a2*cos(e3) + x4*cos(e4) - 1.0*y4*sin(e4)) + cos(e4)*(cos(e2)*cos(e3)*sin(e1) - 1.0*sin(e1)*sin(e2)*sin(e3))*(z4*cos(e4) + cos(e4)*(d4 - 1.0*a2*sin(e3))) + sin(e4)*(cos(e2)*cos(e3)*sin(e1) - 1.0*sin(e1)*sin(e2)*sin(e3))*(z4*sin(e4) + sin(e4)*(d4 - 1.0*a2*sin(e3))) + a2*sin(e3)*(cos(e2)*cos(e3)*sin(e1) - 1.0*sin(e1)*sin(e2)*sin(e3)) + a2*cos(e3)*cos(e4)*(cos(e1)*sin(e4) - 1.0*cos(e4)*(cos(e2)*sin(e1)*sin(e3) + cos(e3)*sin(e1)*sin(e2))) - 1.0*a2*cos(e3)*sin(e4)*(sin(e4)*(cos(e2)*sin(e1)*sin(e3) + cos(e3)*sin(e1)*sin(e2)) + cos(e1)*cos(e4))) + m6*(1.0*(sin(e5)*(cos(e1)*sin(e4) - 1.0*cos(e4)*(cos(e2)*sin(e1)*sin(e3) + cos(e3)*sin(e1)*sin(e2))) + cos(e5)*(cos(e2)*cos(e3)*sin(e1) - 1.0*sin(e1)*sin(e2)*sin(e3)))*(x6*(cos(e4)*cos(e6) - 1.0*cos(e5)*sin(e4)*sin(e6)) - 1.0*y6*(cos(e4)*sin(e6) + cos(e5)*cos(e6)*sin(e4)) + cos(e5)*(a3 + a2*cos(e3)) + cos(e4)*sin(e5)*(d4 - 1.0*a2*sin(e3))) + (cos(e6)*(1.0*cos(e5)*(cos(e1)*sin(e4) - 1.0*cos(e4)*(cos(e2)*sin(e1)*sin(e3) + cos(e3)*sin(e1)*sin(e2))) - sin(e5)*(cos(e2)*cos(e3)*sin(e1) - 1.0*sin(e1)*sin(e2)*sin(e3))) + 1.0*sin(e6)*(sin(e4)*(cos(e2)*sin(e1)*sin(e3) + cos(e3)*sin(e1)*sin(e2)) + cos(e1)*cos(e4)))*(z6*(cos(e4)*cos(e6) - 1.0*cos(e5)*sin(e4)*sin(e6)) - 1.0*cos(e6)*(sin(e5)*(a3 + a2*cos(e3)) - 1.0*cos(e4)*cos(e5)*(d4 - 1.0*a2*sin(e3))) + y6*sin(e4)*sin(e5) - 1.0*sin(e4)*sin(e6)*(d4 - 1.0*a2*sin(e3))) + (sin(e6)*(1.0*cos(e5)*(cos(e1)*sin(e4) - 1.0*cos(e4)*(cos(e2)*sin(e1)*sin(e3) + cos(e3)*sin(e1)*sin(e2))) - sin(e5)*(cos(e2)*cos(e3)*sin(e1) - 1.0*sin(e1)*sin(e2)*sin(e3))) - cos(e6)*(sin(e4)*(cos(e2)*sin(e1)*sin(e3) + cos(e3)*sin(e1)*sin(e2)) + cos(e1)*cos(e4)))*(z6*(cos(e4)*sin(e6) + cos(e5)*cos(e6)*sin(e4)) - 1.0*sin(e6)*(sin(e5)*(a3 + a2*cos(e3)) - 1.0*cos(e4)*cos(e5)*(d4 - 1.0*a2*sin(e3))) + x6*sin(e4)*sin(e5) + cos(e6)*sin(e4)*(d4 - 1.0*a2*sin(e3))))*((sin(e6)*(sin(e5)*(cos(e2)*sin(e1)*sin(e3) + cos(e3)*sin(e1)*sin(e2)) - 1.0*cos(e4)*cos(e5)*(cos(e2)*cos(e3)*sin(e1) - 1.0*sin(e1)*sin(e2)*sin(e3))) - 1.0*cos(e6)*sin(e4)*(cos(e2)*cos(e3)*sin(e1) - 1.0*sin(e1)*sin(e2)*sin(e3)))*(x6*(sin(e2 + e3)*cos(e5) + cos(e2 + e3)*cos(e4)*sin(e5)) - 1.0*z6*(cos(e6)*(sin(e2 + e3)*sin(e5) - 1.0*cos(e2 + e3)*cos(e4)*cos(e5)) + cos(e2 + e3)*sin(e4)*sin(e6)) + cos(e4)*cos(e6)*(a1 + d4*cos(e2 + e3) + a3*sin(e2 + e3) + a2*sin(e2)) - 1.0*cos(e5)*sin(e4)*sin(e6)*(a1 + d4*cos(e2 + e3) + a3*sin(e2 + e3) + a2*sin(e2))) - 1.0*(cos(e5)*(cos(e2)*sin(e1)*sin(e3) + cos(e3)*sin(e1)*sin(e2)) + cos(e4)*sin(e5)*(cos(e2)*cos(e3)*sin(e1) - 1.0*sin(e1)*sin(e2)*sin(e3)))*(x6*(sin(e6)*(sin(e2 + e3)*sin(e5) - 1.0*cos(e2 + e3)*cos(e4)*cos(e5)) - 1.0*cos(e2 + e3)*cos(e6)*sin(e4)) + y6*(cos(e6)*(sin(e2 + e3)*sin(e5) - 1.0*cos(e2 + e3)*cos(e4)*cos(e5)) + cos(e2 + e3)*sin(e4)*sin(e6)) - 1.0*sin(e4)*sin(e5)*(a1 + d4*cos(e2 + e3) + a3*sin(e2 + e3) + a2*sin(e2))) + (cos(e6)*(sin(e5)*(cos(e2)*sin(e1)*sin(e3) + cos(e3)*sin(e1)*sin(e2)) - 1.0*cos(e4)*cos(e5)*(cos(e2)*cos(e3)*sin(e1) - 1.0*sin(e1)*sin(e2)*sin(e3))) + sin(e4)*sin(e6)*(cos(e2)*cos(e3)*sin(e1) - 1.0*sin(e1)*sin(e2)*sin(e3)))*(z6*(sin(e6)*(sin(e2 + e3)*sin(e5) - 1.0*cos(e2 + e3)*cos(e4)*cos(e5)) - 1.0*cos(e2 + e3)*cos(e6)*sin(e4)) + y6*(sin(e2 + e3)*cos(e5) + cos(e2 + e3)*cos(e4)*sin(e5)) - 1.0*cos(e4)*sin(e6)*(a1 + d4*cos(e2 + e3) + a3*sin(e2 + e3) + a2*sin(e2)) - 1.0*cos(e5)*cos(e6)*sin(e4)*(a1 + d4*cos(e2 + e3) + a3*sin(e2 + e3) + a2*sin(e2))) + 1.0*(sin(e6)*(1.0*cos(e5)*(cos(e1)*sin(e4) - 1.0*cos(e4)*(cos(e2)*sin(e1)*sin(e3) + cos(e3)*sin(e1)*sin(e2))) - sin(e5)*(cos(e2)*cos(e3)*sin(e1) - 1.0*sin(e1)*sin(e2)*sin(e3))) - cos(e6)*(sin(e4)*(cos(e2)*sin(e1)*sin(e3) + cos(e3)*sin(e1)*sin(e2)) + cos(e1)*cos(e4)))*(x6*(cos(e2 + e3)*cos(e5) - 1.0*sin(e2 + e3)*cos(e4)*sin(e5)) - 1.0*z6*(cos(e6)*(cos(e2 + e3)*sin(e5) + sin(e2 + e3)*cos(e4)*cos(e5)) - 1.0*sin(e2 + e3)*sin(e4)*sin(e6)) + cos(e4)*cos(e6)*(a3*cos(e2 + e3) - 1.0*d4*sin(e2 + e3)) - 1.0*cos(e5)*sin(e4)*sin(e6)*(a3*cos(e2 + e3) - 1.0*d4*sin(e2 + e3))) + 1.0*(cos(e6)*(1.0*cos(e5)*(cos(e1)*sin(e4) - 1.0*cos(e4)*(cos(e2)*sin(e1)*sin(e3) + cos(e3)*sin(e1)*sin(e2))) - sin(e5)*(cos(e2)*cos(e3)*sin(e1) - 1.0*sin(e1)*sin(e2)*sin(e3))) + 1.0*sin(e6)*(sin(e4)*(cos(e2)*sin(e1)*sin(e3) + cos(e3)*sin(e1)*sin(e2)) + cos(e1)*cos(e4)))*(z6*(sin(e6)*(cos(e2 + e3)*sin(e5) + sin(e2 + e3)*cos(e4)*cos(e5)) + sin(e2 + e3)*cos(e6)*sin(e4)) + y6*(cos(e2 + e3)*cos(e5) - 1.0*sin(e2 + e3)*cos(e4)*sin(e5)) - 1.0*cos(e4)*sin(e6)*(a3*cos(e2 + e3) - 1.0*d4*sin(e2 + e3)) - 1.0*cos(e5)*cos(e6)*sin(e4)*(a3*cos(e2 + e3) - 1.0*d4*sin(e2 + e3))) + (sin(e5)*(cos(e1)*sin(e4) - 1.0*cos(e4)*(cos(e2)*sin(e1)*sin(e3) + cos(e3)*sin(e1)*sin(e2))) + cos(e5)*(cos(e2)*cos(e3)*sin(e1) - 1.0*sin(e1)*sin(e2)*sin(e3)))*(x6*(sin(e6)*(cos(e2 + e3)*sin(e5) + sin(e2 + e3)*cos(e4)*cos(e5)) + sin(e2 + e3)*cos(e6)*sin(e4)) + y6*(cos(e6)*(cos(e2 + e3)*sin(e5) + sin(e2 + e3)*cos(e4)*cos(e5)) - 1.0*sin(e2 + e3)*sin(e4)*sin(e6)) - 1.0*sin(e4)*sin(e5)*(a3*cos(e2 + e3) - 1.0*d4*sin(e2 + e3)))) - m3*(z3*cos(e2 + e3)^2*sin(e1) - 1.0*cos(e1)*(a1 + y3*cos(e2 + e3) + x3*sin(e2 + e3) + a2*sin(e2)) + z3*sin(e2 + e3)^2*sin(e1))*(sin(e2 + e3)*sin(e1)*(x3 + a2*cos(e3)) + cos(e2 + e3)*sin(e1)*(y3 - 1.0*a2*sin(e3)) + a2*cos(e2 + e3)*sin(e1)*sin(e3) - 1.0*a2*sin(e2 + e3)*cos(e3)*sin(e1)) - m5*((sin(e5)*(cos(e1)*cos(e2)*cos(e3) - 1.0*cos(e1)*sin(e2)*sin(e3)) + cos(e5)*(sin(e1)*sin(e4) + cos(e4)*(cos(e1)*cos(e2)*sin(e3) + cos(e1)*cos(e3)*sin(e2))))*(z5*(sin(e2 + e3)*cos(e5) + cos(e2 + e3)*cos(e4)*sin(e5)) + cos(e5)*sin(e4)*(a1 + d4*cos(e2 + e3) + a3*sin(e2 + e3) + a2*sin(e2)) + y5*cos(e2 + e3)*sin(e4)) + (cos(e4)*sin(e1) - 1.0*sin(e4)*(cos(e1)*cos(e2)*sin(e3) + cos(e1)*cos(e3)*sin(e2)))*(cos(e4)*(a1 + d4*cos(e2 + e3) + a3*sin(e2 + e3) + a2*sin(e2)) + x5*(sin(e2 + e3)*cos(e5) + cos(e2 + e3)*cos(e4)*sin(e5)) - 1.0*y5*(sin(e2 + e3)*sin(e5) - 1.0*cos(e2 + e3)*cos(e4)*cos(e5))) - 1.0*(cos(e5)*(cos(e1)*cos(e2)*cos(e3) - 1.0*cos(e1)*sin(e2)*sin(e3)) - 1.0*sin(e5)*(sin(e1)*sin(e4) + cos(e4)*(cos(e1)*cos(e2)*sin(e3) + cos(e1)*cos(e3)*sin(e2))))*(z5*(sin(e2 + e3)*sin(e5) - 1.0*cos(e2 + e3)*cos(e4)*cos(e5)) + sin(e4)*sin(e5)*(a1 + d4*cos(e2 + e3) + a3*sin(e2 + e3) + a2*sin(e2)) + x5*cos(e2 + e3)*sin(e4)))*((a2*sin(e3)*sin(e5) - 1.0*a2*cos(e3)*cos(e4)*cos(e5))*(sin(e5)*(cos(e1)*cos(e2)*cos(e3) - 1.0*cos(e1)*sin(e2)*sin(e3)) + cos(e5)*(sin(e1)*sin(e4) + cos(e4)*(cos(e1)*cos(e2)*sin(e3) + cos(e1)*cos(e3)*sin(e2)))) + (cos(e5)*(cos(e1)*cos(e2)*cos(e3) - 1.0*cos(e1)*sin(e2)*sin(e3)) - 1.0*sin(e5)*(sin(e1)*sin(e4) + cos(e4)*(cos(e1)*cos(e2)*sin(e3) + cos(e1)*cos(e3)*sin(e2))))*(a2*cos(e5)*sin(e3) + a2*cos(e3)*cos(e4)*sin(e5)) + (sin(e5)*(cos(e1)*cos(e2)*sin(e3) + cos(e1)*cos(e3)*sin(e2)) - 1.0*cos(e4)*cos(e5)*(cos(e1)*cos(e2)*cos(e3) - 1.0*cos(e1)*sin(e2)*sin(e3)))*(sin(e5)*(a3 + a2*cos(e3)) - 1.0*y5*cos(e4) + z5*sin(e4)*sin(e5) - 1.0*cos(e4)*cos(e5)*(d4 - 1.0*a2*sin(e3))) + (cos(e5)*(cos(e1)*cos(e2)*sin(e3) + cos(e1)*cos(e3)*sin(e2)) + cos(e4)*sin(e5)*(cos(e1)*cos(e2)*cos(e3) - 1.0*cos(e1)*sin(e2)*sin(e3)))*(cos(e5)*(a3 + a2*cos(e3)) + x5*cos(e4) + z5*cos(e5)*sin(e4) + cos(e4)*sin(e5)*(d4 - 1.0*a2*sin(e3))) + sin(e4)*(cos(e1)*cos(e2)*cos(e3) - 1.0*cos(e1)*sin(e2)*sin(e3))*(sin(e4)*(d4 - 1.0*a2*sin(e3)) + y5*cos(e5)*sin(e4) + x5*sin(e4)*sin(e5)) + a2*cos(e3)*sin(e4)*(cos(e4)*sin(e1) - 1.0*sin(e4)*(cos(e1)*cos(e2)*sin(e3) + cos(e1)*cos(e3)*sin(e2)))) - 0.5*cos(e5)*sin(e4)*(I5xx*(cos(e2 + e3)*sin(e5) + sin(e2 + e3)*cos(e4)*cos(e5)) + I5yx*(cos(e2 + e3)*cos(e5) - 1.0*sin(e2 + e3)*cos(e4)*sin(e5)) + I5zx*sin(e2 + e3)*sin(e4)) + 1.0*m6*((sin(e6)*(1.0*cos(e5)*(cos(e1)*sin(e4) - 1.0*cos(e4)*(cos(e2)*sin(e1)*sin(e3) + cos(e3)*sin(e1)*sin(e2))) - sin(e5)*(cos(e2)*cos(e3)*sin(e1) - 1.0*sin(e1)*sin(e2)*sin(e3))) - cos(e6)*(sin(e4)*(cos(e2)*sin(e1)*sin(e3) + cos(e3)*sin(e1)*sin(e2)) + cos(e1)*cos(e4)))*(x6*(sin(e2 + e3)*cos(e5) + cos(e2 + e3)*cos(e4)*sin(e5)) - 1.0*z6*(cos(e6)*(sin(e2 + e3)*sin(e5) - 1.0*cos(e2 + e3)*cos(e4)*cos(e5)) + cos(e2 + e3)*sin(e4)*sin(e6)) + cos(e4)*cos(e6)*(a1 + d4*cos(e2 + e3) + a3*sin(e2 + e3) + a2*sin(e2)) - 1.0*cos(e5)*sin(e4)*sin(e6)*(a1 + d4*cos(e2 + e3) + a3*sin(e2 + e3) + a2*sin(e2))) + 1.0*(sin(e5)*(cos(e1)*sin(e4) - 1.0*cos(e4)*(cos(e2)*sin(e1)*sin(e3) + cos(e3)*sin(e1)*sin(e2))) + cos(e5)*(cos(e2)*cos(e3)*sin(e1) - 1.0*sin(e1)*sin(e2)*sin(e3)))*(x6*(sin(e6)*(sin(e2 + e3)*sin(e5) - 1.0*cos(e2 + e3)*cos(e4)*cos(e5)) - 1.0*cos(e2 + e3)*cos(e6)*sin(e4)) + y6*(cos(e6)*(sin(e2 + e3)*sin(e5) - 1.0*cos(e2 + e3)*cos(e4)*cos(e5)) + cos(e2 + e3)*sin(e4)*sin(e6)) - 1.0*sin(e4)*sin(e5)*(a1 + d4*cos(e2 + e3) + a3*sin(e2 + e3) + a2*sin(e2))) + (cos(e6)*(1.0*cos(e5)*(cos(e1)*sin(e4) - 1.0*cos(e4)*(cos(e2)*sin(e1)*sin(e3) + cos(e3)*sin(e1)*sin(e2))) - sin(e5)*(cos(e2)*cos(e3)*sin(e1) - 1.0*sin(e1)*sin(e2)*sin(e3))) + 1.0*sin(e6)*(sin(e4)*(cos(e2)*sin(e1)*sin(e3) + cos(e3)*sin(e1)*sin(e2)) + cos(e1)*cos(e4)))*(z6*(sin(e6)*(sin(e2 + e3)*sin(e5) - 1.0*cos(e2 + e3)*cos(e4)*cos(e5)) - 1.0*cos(e2 + e3)*cos(e6)*sin(e4)) + y6*(sin(e2 + e3)*cos(e5) + cos(e2 + e3)*cos(e4)*sin(e5)) - 1.0*cos(e4)*sin(e6)*(a1 + d4*cos(e2 + e3) + a3*sin(e2 + e3) + a2*sin(e2)) - 1.0*cos(e5)*cos(e6)*sin(e4)*(a1 + d4*cos(e2 + e3) + a3*sin(e2 + e3) + a2*sin(e2))))*((cos(e6)*(1.0*cos(e5)*(cos(e1)*sin(e4) - 1.0*cos(e4)*(cos(e2)*sin(e1)*sin(e3) + cos(e3)*sin(e1)*sin(e2))) - sin(e5)*(cos(e2)*cos(e3)*sin(e1) - 1.0*sin(e1)*sin(e2)*sin(e3))) + 1.0*sin(e6)*(sin(e4)*(cos(e2)*sin(e1)*sin(e3) + cos(e3)*sin(e1)*sin(e2)) + cos(e1)*cos(e4)))*(cos(e6)*(a2*sin(e3)*sin(e5) - 1.0*a2*cos(e3)*cos(e4)*cos(e5)) + a2*cos(e3)*sin(e4)*sin(e6)) + (sin(e6)*(a2*sin(e3)*sin(e5) - 1.0*a2*cos(e3)*cos(e4)*cos(e5)) - 1.0*a2*cos(e3)*cos(e6)*sin(e4))*(sin(e6)*(1.0*cos(e5)*(cos(e1)*sin(e4) - 1.0*cos(e4)*(cos(e2)*sin(e1)*sin(e3) + cos(e3)*sin(e1)*sin(e2))) - sin(e5)*(cos(e2)*cos(e3)*sin(e1) - 1.0*sin(e1)*sin(e2)*sin(e3))) - cos(e6)*(sin(e4)*(cos(e2)*sin(e1)*sin(e3) + cos(e3)*sin(e1)*sin(e2)) + cos(e1)*cos(e4))) - (sin(e5)*(cos(e1)*sin(e4) - 1.0*cos(e4)*(cos(e2)*sin(e1)*sin(e3) + cos(e3)*sin(e1)*sin(e2))) + cos(e5)*(cos(e2)*cos(e3)*sin(e1) - 1.0*sin(e1)*sin(e2)*sin(e3)))*(a2*cos(e5)*sin(e3) + a2*cos(e3)*cos(e4)*sin(e5)) - (cos(e5)*(cos(e2)*sin(e1)*sin(e3) + cos(e3)*sin(e1)*sin(e2)) + cos(e4)*sin(e5)*(cos(e2)*cos(e3)*sin(e1) - 1.0*sin(e1)*sin(e2)*sin(e3)))*(x6*(cos(e4)*cos(e6) - 1.0*cos(e5)*sin(e4)*sin(e6)) - 1.0*y6*(cos(e4)*sin(e6) + cos(e5)*cos(e6)*sin(e4)) + cos(e5)*(a3 + a2*cos(e3)) + cos(e4)*sin(e5)*(d4 - 1.0*a2*sin(e3))) + 1.0*(sin(e6)*(sin(e5)*(cos(e2)*sin(e1)*sin(e3) + cos(e3)*sin(e1)*sin(e2)) - 1.0*cos(e4)*cos(e5)*(cos(e2)*cos(e3)*sin(e1) - 1.0*sin(e1)*sin(e2)*sin(e3))) - 1.0*cos(e6)*sin(e4)*(cos(e2)*cos(e3)*sin(e1) - 1.0*sin(e1)*sin(e2)*sin(e3)))*(z6*(cos(e4)*sin(e6) + cos(e5)*cos(e6)*sin(e4)) - 1.0*sin(e6)*(sin(e5)*(a3 + a2*cos(e3)) - 1.0*cos(e4)*cos(e5)*(d4 - 1.0*a2*sin(e3))) + x6*sin(e4)*sin(e5) + cos(e6)*sin(e4)*(d4 - 1.0*a2*sin(e3))) + 1.0*(cos(e6)*(sin(e5)*(cos(e2)*sin(e1)*sin(e3) + cos(e3)*sin(e1)*sin(e2)) - 1.0*cos(e4)*cos(e5)*(cos(e2)*cos(e3)*sin(e1) - 1.0*sin(e1)*sin(e2)*sin(e3))) + sin(e4)*sin(e6)*(cos(e2)*cos(e3)*sin(e1) - 1.0*sin(e1)*sin(e2)*sin(e3)))*(z6*(cos(e4)*cos(e6) - 1.0*cos(e5)*sin(e4)*sin(e6)) - 1.0*cos(e6)*(sin(e5)*(a3 + a2*cos(e3)) - 1.0*cos(e4)*cos(e5)*(d4 - 1.0*a2*sin(e3))) + y6*sin(e4)*sin(e5) - 1.0*sin(e4)*sin(e6)*(d4 - 1.0*a2*sin(e3)))) + 0.5*sin(e4)*sin(e5)*(I5xy*(cos(e2 + e3)*sin(e5) + sin(e2 + e3)*cos(e4)*cos(e5)) + I5yy*(cos(e2 + e3)*cos(e5) - 1.0*sin(e2 + e3)*cos(e4)*sin(e5)) + I5zy*sin(e2 + e3)*sin(e4)) + 1.0*m4*((cos(e2)*sin(e3) + cos(e3)*sin(e2))*(y4*cos(e2 + e3)*cos(e4) + x4*cos(e2 + e3)*sin(e4)) + sin(e4)*(sin(e2)*sin(e3) - 1.0*cos(e2)*cos(e3))*(cos(e4)*(a1 + d4*cos(e2 + e3) + a3*sin(e2 + e3) + a2*sin(e2)) + x4*sin(e2 + e3) + z4*cos(e2 + e3)*cos(e4)) - 1.0*cos(e4)*(sin(e2)*sin(e3) - 1.0*cos(e2)*cos(e3))*(sin(e4)*(a1 + d4*cos(e2 + e3) + a3*sin(e2 + e3) + a2*sin(e2)) - 1.0*y4*sin(e2 + e3) + z4*cos(e2 + e3)*sin(e4)))*((sin(e2)*sin(e3) - 1.0*cos(e2)*cos(e3))*(a3 + a2*cos(e3) + x4*cos(e4) - 1.0*y4*sin(e4)) + cos(e4)*(cos(e2)*sin(e3) + cos(e3)*sin(e2))*(z4*cos(e4) + cos(e4)*(d4 - 1.0*a2*sin(e3))) + sin(e4)*(cos(e2)*sin(e3) + cos(e3)*sin(e2))*(z4*sin(e4) + sin(e4)*(d4 - 1.0*a2*sin(e3))) + a2*sin(e3)*(cos(e2)*sin(e3) + cos(e3)*sin(e2)) - 1.0*a2*cos(e3)*cos(e4)^2*(sin(e2)*sin(e3) - 1.0*cos(e2)*cos(e3)) - 1.0*a2*cos(e3)*sin(e4)^2*(sin(e2)*sin(e3) - 1.0*cos(e2)*cos(e3))) + 0.5*sin(e2 + e3)*sin(e4)*(I5zz*cos(e4) - 1.0*I5xz*cos(e5)*sin(e4) + I5yz*sin(e4)*sin(e5)) - m4*((cos(e4)*sin(e1) - 1.0*sin(e4)*(cos(e1)*cos(e2)*sin(e3) + cos(e1)*cos(e3)*sin(e2)))*(cos(e4)*(a1 + d4*cos(e2 + e3) + a3*sin(e2 + e3) + a2*sin(e2)) + x4*sin(e2 + e3) + z4*cos(e2 + e3)*cos(e4)) - 1.0*(cos(e1)*cos(e2)*cos(e3) - 1.0*cos(e1)*sin(e2)*sin(e3))*(y4*cos(e2 + e3)*cos(e4) + x4*cos(e2 + e3)*sin(e4)) + (sin(e1)*sin(e4) + cos(e4)*(cos(e1)*cos(e2)*sin(e3) + cos(e1)*cos(e3)*sin(e2)))*(sin(e4)*(a1 + d4*cos(e2 + e3) + a3*sin(e2 + e3) + a2*sin(e2)) - 1.0*y4*sin(e2 + e3) + z4*cos(e2 + e3)*sin(e4)))*((cos(e1)*cos(e2)*sin(e3) + cos(e1)*cos(e3)*sin(e2))*(a3 + a2*cos(e3) + x4*cos(e4) - 1.0*y4*sin(e4)) + cos(e4)*(cos(e1)*cos(e2)*cos(e3) - 1.0*cos(e1)*sin(e2)*sin(e3))*(z4*cos(e4) + cos(e4)*(d4 - 1.0*a2*sin(e3))) + sin(e4)*(cos(e1)*cos(e2)*cos(e3) - 1.0*cos(e1)*sin(e2)*sin(e3))*(z4*sin(e4) + sin(e4)*(d4 - 1.0*a2*sin(e3))) + a2*sin(e3)*(cos(e1)*cos(e2)*cos(e3) - 1.0*cos(e1)*sin(e2)*sin(e3)) + a2*cos(e3)*sin(e4)*(cos(e4)*sin(e1) - 1.0*sin(e4)*(cos(e1)*cos(e2)*sin(e3) + cos(e1)*cos(e3)*sin(e2))) - 1.0*a2*cos(e3)*cos(e4)*(sin(e1)*sin(e4) + cos(e4)*(cos(e1)*cos(e2)*sin(e3) + cos(e1)*cos(e3)*sin(e2)))) - m5*((cos(e5)*(cos(e2)*sin(e3) + cos(e3)*sin(e2)) - 1.0*cos(e4)*sin(e5)*(sin(e2)*sin(e3) - 1.0*cos(e2)*cos(e3)))*(cos(e5)*(a3 + a2*cos(e3)) + x5*cos(e4) + z5*cos(e5)*sin(e4) + cos(e4)*sin(e5)*(d4 - 1.0*a2*sin(e3))) + (sin(e5)*(cos(e2)*sin(e3) + cos(e3)*sin(e2)) + cos(e4)*cos(e5)*(sin(e2)*sin(e3) - 1.0*cos(e2)*cos(e3)))*(sin(e5)*(a3 + a2*cos(e3)) - 1.0*y5*cos(e4) + z5*sin(e4)*sin(e5) - 1.0*cos(e4)*cos(e5)*(d4 - 1.0*a2*sin(e3))) - 1.0*sin(e4)*(sin(e2)*sin(e3) - 1.0*cos(e2)*cos(e3))*(sin(e4)*(d4 - 1.0*a2*sin(e3)) + y5*cos(e5)*sin(e4) + x5*sin(e4)*sin(e5)))*((sin(e5)*(sin(e2)*sin(e3) - 1.0*cos(e2)*cos(e3)) - 1.0*cos(e4)*cos(e5)*(cos(e2)*sin(e3) + cos(e3)*sin(e2)))*(z5*(sin(e2 + e3)*cos(e5) + cos(e2 + e3)*cos(e4)*sin(e5)) + cos(e5)*sin(e4)*(a1 + d4*cos(e2 + e3) + a3*sin(e2 + e3) + a2*sin(e2)) + y5*cos(e2 + e3)*sin(e4)) - 1.0*(cos(e5)*(sin(e2)*sin(e3) - 1.0*cos(e2)*cos(e3)) + cos(e4)*sin(e5)*(cos(e2)*sin(e3) + cos(e3)*sin(e2)))*(z5*(sin(e2 + e3)*sin(e5) - 1.0*cos(e2 + e3)*cos(e4)*cos(e5)) + sin(e4)*sin(e5)*(a1 + d4*cos(e2 + e3) + a3*sin(e2 + e3) + a2*sin(e2)) + x5*cos(e2 + e3)*sin(e4)) - 1.0*(sin(e5)*(cos(e2)*sin(e3) + cos(e3)*sin(e2)) + cos(e4)*cos(e5)*(sin(e2)*sin(e3) - 1.0*cos(e2)*cos(e3)))*(z5*(cos(e2 + e3)*cos(e5) - 1.0*sin(e2 + e3)*cos(e4)*sin(e5)) + cos(e5)*sin(e4)*(a3*cos(e2 + e3) - 1.0*d4*sin(e2 + e3)) - 1.0*y5*sin(e2 + e3)*sin(e4)) + (cos(e5)*(cos(e2)*sin(e3) + cos(e3)*sin(e2)) - 1.0*cos(e4)*sin(e5)*(sin(e2)*sin(e3) - 1.0*cos(e2)*cos(e3)))*(z5*(cos(e2 + e3)*sin(e5) + sin(e2 + e3)*cos(e4)*cos(e5)) - 1.0*x5*sin(e2 + e3)*sin(e4) + sin(e4)*sin(e5)*(a3*cos(e2 + e3) - 1.0*d4*sin(e2 + e3))) + sin(e4)*(sin(e2)*sin(e3) - 1.0*cos(e2)*cos(e3))*(cos(e4)*(a3*cos(e2 + e3) - 1.0*d4*sin(e2 + e3)) - 1.0*y5*(cos(e2 + e3)*sin(e5) + sin(e2 + e3)*cos(e4)*cos(e5)) + x5*(cos(e2 + e3)*cos(e5) - 1.0*sin(e2 + e3)*cos(e4)*sin(e5))) + sin(e4)*(cos(e2)*sin(e3) + cos(e3)*sin(e2))*(cos(e4)*(a1 + d4*cos(e2 + e3) + a3*sin(e2 + e3) + a2*sin(e2)) + x5*(sin(e2 + e3)*cos(e5) + cos(e2 + e3)*cos(e4)*sin(e5)) - 1.0*y5*(sin(e2 + e3)*sin(e5) - 1.0*cos(e2 + e3)*cos(e4)*cos(e5)))) + 0.5*sin(e4)*sin(e5)*(I6zz*(cos(e2 + e3)*cos(e5) - 1.0*sin(e2 + e3)*cos(e4)*sin(e5)) - 1.0*I6yz*(sin(e6)*(cos(e2 + e3)*sin(e5) + sin(e2 + e3)*cos(e4)*cos(e5)) + sin(e2 + e3)*cos(e6)*sin(e4)) + I6xz*(cos(e6)*(cos(e2 + e3)*sin(e5) + sin(e2 + e3)*cos(e4)*cos(e5)) - 1.0*sin(e2 + e3)*sin(e4)*sin(e6))) + 1.0*m5*((sin(e4)*(cos(e2)*sin(e1)*sin(e3) + cos(e3)*sin(e1)*sin(e2)) + cos(e1)*cos(e4))*(cos(e4)*(a1 + d4*cos(e2 + e3) + a3*sin(e2 + e3) + a2*sin(e2)) + x5*(sin(e2 + e3)*cos(e5) + cos(e2 + e3)*cos(e4)*sin(e5)) - 1.0*y5*(sin(e2 + e3)*sin(e5) - 1.0*cos(e2 + e3)*cos(e4)*cos(e5))) + 1.0*(1.0*cos(e5)*(cos(e1)*sin(e4) - 1.0*cos(e4)*(cos(e2)*sin(e1)*sin(e3) + cos(e3)*sin(e1)*sin(e2))) - sin(e5)*(cos(e2)*cos(e3)*sin(e1) - 1.0*sin(e1)*sin(e2)*sin(e3)))*(z5*(sin(e2 + e3)*cos(e5) + cos(e2 + e3)*cos(e4)*sin(e5)) + cos(e5)*sin(e4)*(a1 + d4*cos(e2 + e3) + a3*sin(e2 + e3) + a2*sin(e2)) + y5*cos(e2 + e3)*sin(e4)) + (sin(e5)*(cos(e1)*sin(e4) - 1.0*cos(e4)*(cos(e2)*sin(e1)*sin(e3) + cos(e3)*sin(e1)*sin(e2))) + cos(e5)*(cos(e2)*cos(e3)*sin(e1) - 1.0*sin(e1)*sin(e2)*sin(e3)))*(z5*(sin(e2 + e3)*sin(e5) - 1.0*cos(e2 + e3)*cos(e4)*cos(e5)) + sin(e4)*sin(e5)*(a1 + d4*cos(e2 + e3) + a3*sin(e2 + e3) + a2*sin(e2)) + x5*cos(e2 + e3)*sin(e4)))*((sin(e5)*(cos(e1)*sin(e4) - 1.0*cos(e4)*(cos(e2)*sin(e1)*sin(e3) + cos(e3)*sin(e1)*sin(e2))) + cos(e5)*(cos(e2)*cos(e3)*sin(e1) - 1.0*sin(e1)*sin(e2)*sin(e3)))*(a2*cos(e5)*sin(e3) + a2*cos(e3)*cos(e4)*sin(e5)) + (sin(e5)*(cos(e2)*sin(e1)*sin(e3) + cos(e3)*sin(e1)*sin(e2)) - 1.0*cos(e4)*cos(e5)*(cos(e2)*cos(e3)*sin(e1) - 1.0*sin(e1)*sin(e2)*sin(e3)))*(sin(e5)*(a3 + a2*cos(e3)) - 1.0*y5*cos(e4) + z5*sin(e4)*sin(e5) - 1.0*cos(e4)*cos(e5)*(d4 - 1.0*a2*sin(e3))) - (1.0*cos(e5)*(cos(e1)*sin(e4) - 1.0*cos(e4)*(cos(e2)*sin(e1)*sin(e3) + cos(e3)*sin(e1)*sin(e2))) - sin(e5)*(cos(e2)*cos(e3)*sin(e1) - 1.0*sin(e1)*sin(e2)*sin(e3)))*(a2*sin(e3)*sin(e5) - 1.0*a2*cos(e3)*cos(e4)*cos(e5)) + (cos(e5)*(cos(e2)*sin(e1)*sin(e3) + cos(e3)*sin(e1)*sin(e2)) + cos(e4)*sin(e5)*(cos(e2)*cos(e3)*sin(e1) - 1.0*sin(e1)*sin(e2)*sin(e3)))*(cos(e5)*(a3 + a2*cos(e3)) + x5*cos(e4) + z5*cos(e5)*sin(e4) + cos(e4)*sin(e5)*(d4 - 1.0*a2*sin(e3))) + sin(e4)*(cos(e2)*cos(e3)*sin(e1) - 1.0*sin(e1)*sin(e2)*sin(e3))*(sin(e4)*(d4 - 1.0*a2*sin(e3)) + y5*cos(e5)*sin(e4) + x5*sin(e4)*sin(e5)) - 1.0*a2*cos(e3)*sin(e4)*(sin(e4)*(cos(e2)*sin(e1)*sin(e3) + cos(e3)*sin(e1)*sin(e2)) + cos(e1)*cos(e4))) + 1.0*m5*((cos(e5)*(cos(e2)*sin(e3) + cos(e3)*sin(e2)) - 1.0*cos(e4)*sin(e5)*(sin(e2)*sin(e3) - 1.0*cos(e2)*cos(e3)))*(z5*(sin(e2 + e3)*sin(e5) - 1.0*cos(e2 + e3)*cos(e4)*cos(e5)) + sin(e4)*sin(e5)*(a1 + d4*cos(e2 + e3) + a3*sin(e2 + e3) + a2*sin(e2)) + x5*cos(e2 + e3)*sin(e4)) - 1.0*(sin(e5)*(cos(e2)*sin(e3) + cos(e3)*sin(e2)) + cos(e4)*cos(e5)*(sin(e2)*sin(e3) - 1.0*cos(e2)*cos(e3)))*(z5*(sin(e2 + e3)*cos(e5) + cos(e2 + e3)*cos(e4)*sin(e5)) + cos(e5)*sin(e4)*(a1 + d4*cos(e2 + e3) + a3*sin(e2 + e3) + a2*sin(e2)) + y5*cos(e2 + e3)*sin(e4)) + sin(e4)*(sin(e2)*sin(e3) - 1.0*cos(e2)*cos(e3))*(cos(e4)*(a1 + d4*cos(e2 + e3) + a3*sin(e2 + e3) + a2*sin(e2)) + x5*(sin(e2 + e3)*cos(e5) + cos(e2 + e3)*cos(e4)*sin(e5)) - 1.0*y5*(sin(e2 + e3)*sin(e5) - 1.0*cos(e2 + e3)*cos(e4)*cos(e5))))*((a2*sin(e3)*sin(e5) - 1.0*a2*cos(e3)*cos(e4)*cos(e5))*(sin(e5)*(cos(e2)*sin(e3) + cos(e3)*sin(e2)) + cos(e4)*cos(e5)*(sin(e2)*sin(e3) - 1.0*cos(e2)*cos(e3))) + (cos(e5)*(cos(e2)*sin(e3) + cos(e3)*sin(e2)) - 1.0*cos(e4)*sin(e5)*(sin(e2)*sin(e3) - 1.0*cos(e2)*cos(e3)))*(a2*cos(e5)*sin(e3) + a2*cos(e3)*cos(e4)*sin(e5)) + (sin(e5)*(sin(e2)*sin(e3) - 1.0*cos(e2)*cos(e3)) - 1.0*cos(e4)*cos(e5)*(cos(e2)*sin(e3) + cos(e3)*sin(e2)))*(sin(e5)*(a3 + a2*cos(e3)) - 1.0*y5*cos(e4) + z5*sin(e4)*sin(e5) - 1.0*cos(e4)*cos(e5)*(d4 - 1.0*a2*sin(e3))) + (cos(e5)*(sin(e2)*sin(e3) - 1.0*cos(e2)*cos(e3)) + cos(e4)*sin(e5)*(cos(e2)*sin(e3) + cos(e3)*sin(e2)))*(cos(e5)*(a3 + a2*cos(e3)) + x5*cos(e4) + z5*cos(e5)*sin(e4) + cos(e4)*sin(e5)*(d4 - 1.0*a2*sin(e3))) + sin(e4)*(cos(e2)*sin(e3) + cos(e3)*sin(e2))*(sin(e4)*(d4 - 1.0*a2*sin(e3)) + y5*cos(e5)*sin(e4) + x5*sin(e4)*sin(e5)) - 1.0*a2*cos(e3)*sin(e4)^2*(sin(e2)*sin(e3) - 1.0*cos(e2)*cos(e3))) - m3*(sin(e1)*(a1 + y3*cos(e2 + e3) + x3*sin(e2 + e3) + a2*sin(e2)) + z3*cos(e2 + e3)^2*cos(e1) + z3*sin(e2 + e3)^2*cos(e1))*(sin(e2 + e3)*cos(e1)*(x3 + a2*cos(e3)) + cos(e2 + e3)*cos(e1)*(y3 - 1.0*a2*sin(e3)) + a2*cos(e2 + e3)*cos(e1)*sin(e3) - 1.0*a2*sin(e2 + e3)*cos(e1)*cos(e3)) + 1.0*m6*((sin(e6)*(sin(e5)*(cos(e1)*cos(e2)*cos(e3) - 1.0*cos(e1)*sin(e2)*sin(e3)) + cos(e5)*(sin(e1)*sin(e4) + cos(e4)*(cos(e1)*cos(e2)*sin(e3) + cos(e1)*cos(e3)*sin(e2)))) - 1.0*cos(e6)*(cos(e4)*sin(e1) - 1.0*sin(e4)*(cos(e1)*cos(e2)*sin(e3) + cos(e1)*cos(e3)*sin(e2))))*(z6*(cos(e4)*sin(e6) + cos(e5)*cos(e6)*sin(e4)) - 1.0*sin(e6)*(sin(e5)*(a3 + a2*cos(e3)) - 1.0*cos(e4)*cos(e5)*(d4 - 1.0*a2*sin(e3))) + x6*sin(e4)*sin(e5) + cos(e6)*sin(e4)*(d4 - 1.0*a2*sin(e3))) - 1.0*(cos(e5)*(cos(e1)*cos(e2)*cos(e3) - 1.0*cos(e1)*sin(e2)*sin(e3)) - 1.0*sin(e5)*(sin(e1)*sin(e4) + cos(e4)*(cos(e1)*cos(e2)*sin(e3) + cos(e1)*cos(e3)*sin(e2))))*(x6*(cos(e4)*cos(e6) - 1.0*cos(e5)*sin(e4)*sin(e6)) - 1.0*y6*(cos(e4)*sin(e6) + cos(e5)*cos(e6)*sin(e4)) + cos(e5)*(a3 + a2*cos(e3)) + cos(e4)*sin(e5)*(d4 - 1.0*a2*sin(e3))) + (sin(e6)*(cos(e4)*sin(e1) - 1.0*sin(e4)*(cos(e1)*cos(e2)*sin(e3) + cos(e1)*cos(e3)*sin(e2))) + cos(e6)*(sin(e5)*(cos(e1)*cos(e2)*cos(e3) - 1.0*cos(e1)*sin(e2)*sin(e3)) + cos(e5)*(sin(e1)*sin(e4) + cos(e4)*(cos(e1)*cos(e2)*sin(e3) + cos(e1)*cos(e3)*sin(e2)))))*(z6*(cos(e4)*cos(e6) - 1.0*cos(e5)*sin(e4)*sin(e6)) - 1.0*cos(e6)*(sin(e5)*(a3 + a2*cos(e3)) - 1.0*cos(e4)*cos(e5)*(d4 - 1.0*a2*sin(e3))) + y6*sin(e4)*sin(e5) - 1.0*sin(e4)*sin(e6)*(d4 - 1.0*a2*sin(e3))))*((sin(e6)*(cos(e4)*sin(e1) - 1.0*sin(e4)*(cos(e1)*cos(e2)*sin(e3) + cos(e1)*cos(e3)*sin(e2))) + cos(e6)*(sin(e5)*(cos(e1)*cos(e2)*cos(e3) - 1.0*cos(e1)*sin(e2)*sin(e3)) + cos(e5)*(sin(e1)*sin(e4) + cos(e4)*(cos(e1)*cos(e2)*sin(e3) + cos(e1)*cos(e3)*sin(e2)))))*(z6*(sin(e6)*(cos(e2 + e3)*sin(e5) + sin(e2 + e3)*cos(e4)*cos(e5)) + sin(e2 + e3)*cos(e6)*sin(e4)) + y6*(cos(e2 + e3)*cos(e5) - 1.0*sin(e2 + e3)*cos(e4)*sin(e5)) - 1.0*cos(e4)*sin(e6)*(a3*cos(e2 + e3) - 1.0*d4*sin(e2 + e3)) - 1.0*cos(e5)*cos(e6)*sin(e4)*(a3*cos(e2 + e3) - 1.0*d4*sin(e2 + e3))) - 1.0*(sin(e6)*(sin(e5)*(cos(e1)*cos(e2)*sin(e3) + cos(e1)*cos(e3)*sin(e2)) - 1.0*cos(e4)*cos(e5)*(cos(e1)*cos(e2)*cos(e3) - 1.0*cos(e1)*sin(e2)*sin(e3))) - 1.0*cos(e6)*sin(e4)*(cos(e1)*cos(e2)*cos(e3) - 1.0*cos(e1)*sin(e2)*sin(e3)))*(x6*(sin(e2 + e3)*cos(e5) + cos(e2 + e3)*cos(e4)*sin(e5)) - 1.0*z6*(cos(e6)*(sin(e2 + e3)*sin(e5) - 1.0*cos(e2 + e3)*cos(e4)*cos(e5)) + cos(e2 + e3)*sin(e4)*sin(e6)) + cos(e4)*cos(e6)*(a1 + d4*cos(e2 + e3) + a3*sin(e2 + e3) + a2*sin(e2)) - 1.0*cos(e5)*sin(e4)*sin(e6)*(a1 + d4*cos(e2 + e3) + a3*sin(e2 + e3) + a2*sin(e2))) - 1.0*(cos(e6)*(sin(e5)*(cos(e1)*cos(e2)*sin(e3) + cos(e1)*cos(e3)*sin(e2)) - 1.0*cos(e4)*cos(e5)*(cos(e1)*cos(e2)*cos(e3) - 1.0*cos(e1)*sin(e2)*sin(e3))) + sin(e4)*sin(e6)*(cos(e1)*cos(e2)*cos(e3) - 1.0*cos(e1)*sin(e2)*sin(e3)))*(z6*(sin(e6)*(sin(e2 + e3)*sin(e5) - 1.0*cos(e2 + e3)*cos(e4)*cos(e5)) - 1.0*cos(e2 + e3)*cos(e6)*sin(e4)) + y6*(sin(e2 + e3)*cos(e5) + cos(e2 + e3)*cos(e4)*sin(e5)) - 1.0*cos(e4)*sin(e6)*(a1 + d4*cos(e2 + e3) + a3*sin(e2 + e3) + a2*sin(e2)) - 1.0*cos(e5)*cos(e6)*sin(e4)*(a1 + d4*cos(e2 + e3) + a3*sin(e2 + e3) + a2*sin(e2))) + (sin(e6)*(sin(e5)*(cos(e1)*cos(e2)*cos(e3) - 1.0*cos(e1)*sin(e2)*sin(e3)) + cos(e5)*(sin(e1)*sin(e4) + cos(e4)*(cos(e1)*cos(e2)*sin(e3) + cos(e1)*cos(e3)*sin(e2)))) - 1.0*cos(e6)*(cos(e4)*sin(e1) - 1.0*sin(e4)*(cos(e1)*cos(e2)*sin(e3) + cos(e1)*cos(e3)*sin(e2))))*(x6*(cos(e2 + e3)*cos(e5) - 1.0*sin(e2 + e3)*cos(e4)*sin(e5)) - 1.0*z6*(cos(e6)*(cos(e2 + e3)*sin(e5) + sin(e2 + e3)*cos(e4)*cos(e5)) - 1.0*sin(e2 + e3)*sin(e4)*sin(e6)) + cos(e4)*cos(e6)*(a3*cos(e2 + e3) - 1.0*d4*sin(e2 + e3)) - 1.0*cos(e5)*sin(e4)*sin(e6)*(a3*cos(e2 + e3) - 1.0*d4*sin(e2 + e3))) - 1.0*(cos(e5)*(cos(e1)*cos(e2)*cos(e3) - 1.0*cos(e1)*sin(e2)*sin(e3)) - 1.0*sin(e5)*(sin(e1)*sin(e4) + cos(e4)*(cos(e1)*cos(e2)*sin(e3) + cos(e1)*cos(e3)*sin(e2))))*(x6*(sin(e6)*(cos(e2 + e3)*sin(e5) + sin(e2 + e3)*cos(e4)*cos(e5)) + sin(e2 + e3)*cos(e6)*sin(e4)) + y6*(cos(e6)*(cos(e2 + e3)*sin(e5) + sin(e2 + e3)*cos(e4)*cos(e5)) - 1.0*sin(e2 + e3)*sin(e4)*sin(e6)) - 1.0*sin(e4)*sin(e5)*(a3*cos(e2 + e3) - 1.0*d4*sin(e2 + e3))) + (cos(e5)*(cos(e1)*cos(e2)*sin(e3) + cos(e1)*cos(e3)*sin(e2)) + cos(e4)*sin(e5)*(cos(e1)*cos(e2)*cos(e3) - 1.0*cos(e1)*sin(e2)*sin(e3)))*(x6*(sin(e6)*(sin(e2 + e3)*sin(e5) - 1.0*cos(e2 + e3)*cos(e4)*cos(e5)) - 1.0*cos(e2 + e3)*cos(e6)*sin(e4)) + y6*(cos(e6)*(sin(e2 + e3)*sin(e5) - 1.0*cos(e2 + e3)*cos(e4)*cos(e5)) + cos(e2 + e3)*sin(e4)*sin(e6)) - 1.0*sin(e4)*sin(e5)*(a1 + d4*cos(e2 + e3) + a3*sin(e2 + e3) + a2*sin(e2)))) - m4*(cos(e4)*(sin(e2)*sin(e3) - 1.0*cos(e2)*cos(e3))*(z4*cos(e4) + cos(e4)*(d4 - 1.0*a2*sin(e3))) - 1.0*(cos(e2)*sin(e3) + cos(e3)*sin(e2))*(a3 + a2*cos(e3) + x4*cos(e4) - 1.0*y4*sin(e4)) + sin(e4)*(sin(e2)*sin(e3) - 1.0*cos(e2)*cos(e3))*(z4*sin(e4) + sin(e4)*(d4 - 1.0*a2*sin(e3))))*((cos(e2)*sin(e3) + cos(e3)*sin(e2))*(y4*sin(e2 + e3)*cos(e4) + x4*sin(e2 + e3)*sin(e4)) + (sin(e2)*sin(e3) - 1.0*cos(e2)*cos(e3))*(y4*cos(e2 + e3)*cos(e4) + x4*cos(e2 + e3)*sin(e4)) + cos(e4)*(cos(e2)*sin(e3) + cos(e3)*sin(e2))*(sin(e4)*(a1 + d4*cos(e2 + e3) + a3*sin(e2 + e3) + a2*sin(e2)) - 1.0*y4*sin(e2 + e3) + z4*cos(e2 + e3)*sin(e4)) - 1.0*sin(e4)*(sin(e2)*sin(e3) - 1.0*cos(e2)*cos(e3))*(x4*cos(e2 + e3) + cos(e4)*(a3*cos(e2 + e3) - 1.0*d4*sin(e2 + e3)) - 1.0*z4*sin(e2 + e3)*cos(e4)) - 1.0*cos(e4)*(sin(e2)*sin(e3) - 1.0*cos(e2)*cos(e3))*(y4*cos(e2 + e3) - 1.0*sin(e4)*(a3*cos(e2 + e3) - 1.0*d4*sin(e2 + e3)) + z4*sin(e2 + e3)*sin(e4)) - 1.0*sin(e4)*(cos(e2)*sin(e3) + cos(e3)*sin(e2))*(cos(e4)*(a1 + d4*cos(e2 + e3) + a3*sin(e2 + e3) + a2*sin(e2)) + x4*sin(e2 + e3) + z4*cos(e2 + e3)*cos(e4))) + m6*((cos(e6)*(sin(e5)*(cos(e2)*sin(e3) + cos(e3)*sin(e2)) + cos(e4)*cos(e5)*(sin(e2)*sin(e3) - 1.0*cos(e2)*cos(e3))) - 1.0*sin(e4)*sin(e6)*(sin(e2)*sin(e3) - 1.0*cos(e2)*cos(e3)))*(z6*(cos(e4)*cos(e6) - 1.0*cos(e5)*sin(e4)*sin(e6)) - 1.0*cos(e6)*(sin(e5)*(a3 + a2*cos(e3)) - 1.0*cos(e4)*cos(e5)*(d4 - 1.0*a2*sin(e3))) + y6*sin(e4)*sin(e5) - 1.0*sin(e4)*sin(e6)*(d4 - 1.0*a2*sin(e3))) - 1.0*(cos(e5)*(cos(e2)*sin(e3) + cos(e3)*sin(e2)) - 1.0*cos(e4)*sin(e5)*(sin(e2)*sin(e3) - 1.0*cos(e2)*cos(e3)))*(x6*(cos(e4)*cos(e6) - 1.0*cos(e5)*sin(e4)*sin(e6)) - 1.0*y6*(cos(e4)*sin(e6) + cos(e5)*cos(e6)*sin(e4)) + cos(e5)*(a3 + a2*cos(e3)) + cos(e4)*sin(e5)*(d4 - 1.0*a2*sin(e3))) + (sin(e6)*(sin(e5)*(cos(e2)*sin(e3) + cos(e3)*sin(e2)) + cos(e4)*cos(e5)*(sin(e2)*sin(e3) - 1.0*cos(e2)*cos(e3))) + cos(e6)*sin(e4)*(sin(e2)*sin(e3) - 1.0*cos(e2)*cos(e3)))*(z6*(cos(e4)*sin(e6) + cos(e5)*cos(e6)*sin(e4)) - 1.0*sin(e6)*(sin(e5)*(a3 + a2*cos(e3)) - 1.0*cos(e4)*cos(e5)*(d4 - 1.0*a2*sin(e3))) + x6*sin(e4)*sin(e5) + cos(e6)*sin(e4)*(d4 - 1.0*a2*sin(e3))))*(1.0*(sin(e6)*(sin(e5)*(cos(e2)*sin(e3) + cos(e3)*sin(e2)) + cos(e4)*cos(e5)*(sin(e2)*sin(e3) - 1.0*cos(e2)*cos(e3))) + cos(e6)*sin(e4)*(sin(e2)*sin(e3) - 1.0*cos(e2)*cos(e3)))*(x6*(cos(e2 + e3)*cos(e5) - 1.0*sin(e2 + e3)*cos(e4)*sin(e5)) - 1.0*z6*(cos(e6)*(cos(e2 + e3)*sin(e5) + sin(e2 + e3)*cos(e4)*cos(e5)) - 1.0*sin(e2 + e3)*sin(e4)*sin(e6)) + cos(e4)*cos(e6)*(a3*cos(e2 + e3) - 1.0*d4*sin(e2 + e3)) - 1.0*cos(e5)*sin(e4)*sin(e6)*(a3*cos(e2 + e3) - 1.0*d4*sin(e2 + e3))) + 1.0*(cos(e6)*(sin(e5)*(cos(e2)*sin(e3) + cos(e3)*sin(e2)) + cos(e4)*cos(e5)*(sin(e2)*sin(e3) - 1.0*cos(e2)*cos(e3))) - 1.0*sin(e4)*sin(e6)*(sin(e2)*sin(e3) - 1.0*cos(e2)*cos(e3)))*(z6*(sin(e6)*(cos(e2 + e3)*sin(e5) + sin(e2 + e3)*cos(e4)*cos(e5)) + sin(e2 + e3)*cos(e6)*sin(e4)) + y6*(cos(e2 + e3)*cos(e5) - 1.0*sin(e2 + e3)*cos(e4)*sin(e5)) - 1.0*cos(e4)*sin(e6)*(a3*cos(e2 + e3) - 1.0*d4*sin(e2 + e3)) - 1.0*cos(e5)*cos(e6)*sin(e4)*(a3*cos(e2 + e3) - 1.0*d4*sin(e2 + e3))) - (sin(e6)*(sin(e5)*(sin(e2)*sin(e3) - 1.0*cos(e2)*cos(e3)) - 1.0*cos(e4)*cos(e5)*(cos(e2)*sin(e3) + cos(e3)*sin(e2))) - 1.0*cos(e6)*sin(e4)*(cos(e2)*sin(e3) + cos(e3)*sin(e2)))*(x6*(sin(e2 + e3)*cos(e5) + cos(e2 + e3)*cos(e4)*sin(e5)) - 1.0*z6*(cos(e6)*(sin(e2 + e3)*sin(e5) - 1.0*cos(e2 + e3)*cos(e4)*cos(e5)) + cos(e2 + e3)*sin(e4)*sin(e6)) + cos(e4)*cos(e6)*(a1 + d4*cos(e2 + e3) + a3*sin(e2 + e3) + a2*sin(e2)) - 1.0*cos(e5)*sin(e4)*sin(e6)*(a1 + d4*cos(e2 + e3) + a3*sin(e2 + e3) + a2*sin(e2))) - (cos(e6)*(sin(e5)*(sin(e2)*sin(e3) - 1.0*cos(e2)*cos(e3)) - 1.0*cos(e4)*cos(e5)*(cos(e2)*sin(e3) + cos(e3)*sin(e2))) + sin(e4)*sin(e6)*(cos(e2)*sin(e3) + cos(e3)*sin(e2)))*(z6*(sin(e6)*(sin(e2 + e3)*sin(e5) - 1.0*cos(e2 + e3)*cos(e4)*cos(e5)) - 1.0*cos(e2 + e3)*cos(e6)*sin(e4)) + y6*(sin(e2 + e3)*cos(e5) + cos(e2 + e3)*cos(e4)*sin(e5)) - 1.0*cos(e4)*sin(e6)*(a1 + d4*cos(e2 + e3) + a3*sin(e2 + e3) + a2*sin(e2)) - 1.0*cos(e5)*cos(e6)*sin(e4)*(a1 + d4*cos(e2 + e3) + a3*sin(e2 + e3) + a2*sin(e2))) + 1.0*(cos(e5)*(sin(e2)*sin(e3) - 1.0*cos(e2)*cos(e3)) + cos(e4)*sin(e5)*(cos(e2)*sin(e3) + cos(e3)*sin(e2)))*(x6*(sin(e6)*(sin(e2 + e3)*sin(e5) - 1.0*cos(e2 + e3)*cos(e4)*cos(e5)) - 1.0*cos(e2 + e3)*cos(e6)*sin(e4)) + y6*(cos(e6)*(sin(e2 + e3)*sin(e5) - 1.0*cos(e2 + e3)*cos(e4)*cos(e5)) + cos(e2 + e3)*sin(e4)*sin(e6)) - 1.0*sin(e4)*sin(e5)*(a1 + d4*cos(e2 + e3) + a3*sin(e2 + e3) + a2*sin(e2))) - (cos(e5)*(cos(e2)*sin(e3) + cos(e3)*sin(e2)) - 1.0*cos(e4)*sin(e5)*(sin(e2)*sin(e3) - 1.0*cos(e2)*cos(e3)))*(x6*(sin(e6)*(cos(e2 + e3)*sin(e5) + sin(e2 + e3)*cos(e4)*cos(e5)) + sin(e2 + e3)*cos(e6)*sin(e4)) + y6*(cos(e6)*(cos(e2 + e3)*sin(e5) + sin(e2 + e3)*cos(e4)*cos(e5)) - 1.0*sin(e2 + e3)*sin(e4)*sin(e6)) - 1.0*sin(e4)*sin(e5)*(a3*cos(e2 + e3) - 1.0*d4*sin(e2 + e3)))) + 1.0*m3*sin(e1)*(cos(e2 + e3)*cos(e1)*(x3 + a2*cos(e3)) - 1.0*sin(e2 + e3)*cos(e1)*(y3 - 1.0*a2*sin(e3)))*(x3*cos(e2 + e3) - 1.0*y3*sin(e2 + e3)) - m3*cos(e1)*(cos(e2 + e3)*sin(e1)*(x3 + a2*cos(e3)) - 1.0*sin(e2 + e3)*sin(e1)*(y3 - 1.0*a2*sin(e3)))*(x3*cos(e2 + e3) - 1.0*y3*sin(e2 + e3))))/2 + de4*((cos(e4)*(I5zz*cos(e2 + e3)*cos(e4) - I5xz*cos(e2 + e3)*cos(e5)*sin(e4) + I5yz*cos(e2 + e3)*sin(e4)*sin(e5)))/2 - ((cos(e6)*sin(e4) + cos(e4)*cos(e5)*sin(e6))*(I6zy*(sin(e2 + e3)*cos(e5) + cos(e2 + e3)*cos(e4)*sin(e5)) + I6xy*(cos(e6)*(sin(e2 + e3)*sin(e5) - cos(e2 + e3)*cos(e4)*cos(e5)) + cos(e2 + e3)*sin(e4)*sin(e6)) - I6yy*(sin(e6)*(sin(e2 + e3)*sin(e5) - cos(e2 + e3)*cos(e4)*cos(e5)) - cos(e2 + e3)*cos(e6)*sin(e4))))/2 - ((sin(e4)*sin(e6) - cos(e4)*cos(e5)*cos(e6))*(I6zx*(sin(e2 + e3)*cos(e5) + cos(e2 + e3)*cos(e4)*sin(e5)) + I6xx*(cos(e6)*(sin(e2 + e3)*sin(e5) - cos(e2 + e3)*cos(e4)*cos(e5)) + cos(e2 + e3)*sin(e4)*sin(e6)) - I6yx*(sin(e6)*(sin(e2 + e3)*sin(e5) - cos(e2 + e3)*cos(e4)*cos(e5)) - cos(e2 + e3)*cos(e6)*sin(e4))))/2 + (sin(e2 + e3)*(I4xz*cos(e4) - I4yz*sin(e4)))/2 + (sin(e4)*(I5xz*(sin(e2 + e3)*sin(e5) - cos(e2 + e3)*cos(e4)*cos(e5)) + I5yz*(sin(e2 + e3)*cos(e5) + cos(e2 + e3)*cos(e4)*sin(e5)) - I5zz*cos(e2 + e3)*sin(e4)))/2 - ((sin(e2 + e3)*cos(e5) + cos(e2 + e3)*cos(e4)*sin(e5))*(I6xz*(sin(e4)*sin(e6) - cos(e4)*cos(e5)*cos(e6)) + I6yz*(cos(e6)*sin(e4) + cos(e4)*cos(e5)*sin(e6)) + I6zz*cos(e4)*sin(e5)))/2 + ((sin(e2 + e3)*sin(e5) - cos(e2 + e3)*cos(e4)*cos(e5))*(I5zx*sin(e4) + I5xx*cos(e4)*cos(e5) - I5yx*cos(e4)*sin(e5)))/2 + ((sin(e2 + e3)*cos(e5) + cos(e2 + e3)*cos(e4)*sin(e5))*(I5zy*sin(e4) + I5xy*cos(e4)*cos(e5) - I5yy*cos(e4)*sin(e5)))/2 - ((cos(e6)*(sin(e2 + e3)*sin(e5) - cos(e2 + e3)*cos(e4)*cos(e5)) + cos(e2 + e3)*sin(e4)*sin(e6))*(I6xx*(sin(e4)*sin(e6) - cos(e4)*cos(e5)*cos(e6)) + I6yx*(cos(e6)*sin(e4) + cos(e4)*cos(e5)*sin(e6)) + I6zx*cos(e4)*sin(e5)))/2 + ((sin(e6)*(sin(e2 + e3)*sin(e5) - cos(e2 + e3)*cos(e4)*cos(e5)) - cos(e2 + e3)*cos(e6)*sin(e4))*(I6xy*(sin(e4)*sin(e6) - cos(e4)*cos(e5)*cos(e6)) + I6yy*(cos(e6)*sin(e4) + cos(e4)*cos(e5)*sin(e6)) + I6zy*cos(e4)*sin(e5)))/2 + (cos(e4)*(I4xy*cos(e2 + e3)*sin(e4) + I4yy*cos(e2 + e3)*cos(e4)))/2 + ((cos(e4)*sin(e6) + cos(e5)*cos(e6)*sin(e4))*(I6xx*(cos(e2 + e3)*cos(e4)*sin(e6) + cos(e2 + e3)*cos(e5)*cos(e6)*sin(e4)) + I6yx*(cos(e2 + e3)*cos(e4)*cos(e6) - cos(e2 + e3)*cos(e5)*sin(e4)*sin(e6)) - I6zx*cos(e2 + e3)*sin(e4)*sin(e5)))/2 + ((cos(e4)*cos(e6) - cos(e5)*sin(e4)*sin(e6))*(I6xy*(cos(e2 + e3)*cos(e4)*sin(e6) + cos(e2 + e3)*cos(e5)*cos(e6)*sin(e4)) + I6yy*(cos(e2 + e3)*cos(e4)*cos(e6) - cos(e2 + e3)*cos(e5)*sin(e4)*sin(e6)) - I6zy*cos(e2 + e3)*sin(e4)*sin(e5)))/2 + (sin(e4)*(I4xx*cos(e2 + e3)*sin(e4) + I4yx*cos(e2 + e3)*cos(e4)))/2 + (cos(e4)*(I4zx*sin(e2 + e3) + I4yx*cos(e2 + e3)*sin(e4) - I4xx*cos(e2 + e3)*cos(e4)))/2 - (sin(e4)*(I4zy*sin(e2 + e3) + I4yy*cos(e2 + e3)*sin(e4) - I4xy*cos(e2 + e3)*cos(e4)))/2 + ((cos(e2 + e3)*cos(e4)*sin(e6) + cos(e2 + e3)*cos(e5)*cos(e6)*sin(e4))*(I6xx*(cos(e4)*sin(e6) + cos(e5)*cos(e6)*sin(e4)) + I6yx*(cos(e4)*cos(e6) - cos(e5)*sin(e4)*sin(e6)) - I6zx*sin(e4)*sin(e5)))/2 + ((cos(e2 + e3)*cos(e4)*cos(e6) - cos(e2 + e3)*cos(e5)*sin(e4)*sin(e6))*(I6xy*(cos(e4)*sin(e6) + cos(e5)*cos(e6)*sin(e4)) + I6yy*(cos(e4)*cos(e6) - cos(e5)*sin(e4)*sin(e6)) - I6zy*sin(e4)*sin(e5)))/2 - (cos(e2 + e3)*cos(e4)*(I4xx*cos(e4) - I4yx*sin(e4)))/2 + (cos(e2 + e3)*cos(e4)*(I4yy*cos(e4) + I4xy*sin(e4)))/2 + (cos(e4)*cos(e5)*(I5xx*(sin(e2 + e3)*sin(e5) - cos(e2 + e3)*cos(e4)*cos(e5)) + I5yx*(sin(e2 + e3)*cos(e5) + cos(e2 + e3)*cos(e4)*sin(e5)) - I5zx*cos(e2 + e3)*sin(e4)))/2 + (cos(e2 + e3)*sin(e4)*(I4yx*cos(e4) + I4xx*sin(e4)))/2 + (cos(e2 + e3)*sin(e4)*(I4xy*cos(e4) - I4yy*sin(e4)))/2 - (cos(e5)*sin(e4)*(I5zx*cos(e2 + e3)*cos(e4) - I5xx*cos(e2 + e3)*cos(e5)*sin(e4) + I5yx*cos(e2 + e3)*sin(e4)*sin(e5)))/2 - (cos(e4)*sin(e5)*(I5xy*(sin(e2 + e3)*sin(e5) - cos(e2 + e3)*cos(e4)*cos(e5)) + I5yy*(sin(e2 + e3)*cos(e5) + cos(e2 + e3)*cos(e4)*sin(e5)) - I5zy*cos(e2 + e3)*sin(e4)))/2 + (cos(e2 + e3)*cos(e4)*(I5zz*cos(e4) - I5xz*cos(e5)*sin(e4) + I5yz*sin(e4)*sin(e5)))/2 - (cos(e2 + e3)*sin(e4)*(I5zz*sin(e4) + I5xz*cos(e4)*cos(e5) - I5yz*cos(e4)*sin(e5)))/2 + (sin(e4)*sin(e5)*(I5zy*cos(e2 + e3)*cos(e4) - I5xy*cos(e2 + e3)*cos(e5)*sin(e4) + I5yy*cos(e2 + e3)*sin(e4)*sin(e5)))/2 - (sin(e4)*sin(e5)*(I6xz*(cos(e2 + e3)*cos(e4)*sin(e6) + cos(e2 + e3)*cos(e5)*cos(e6)*sin(e4)) + I6yz*(cos(e2 + e3)*cos(e4)*cos(e6) - cos(e2 + e3)*cos(e5)*sin(e4)*sin(e6)) - I6zz*cos(e2 + e3)*sin(e4)*sin(e5)))/2 + m6*((sin(e6)*(sin(e5)*(cos(e1)*cos(e2)*cos(e3) - cos(e1)*sin(e2)*sin(e3)) + cos(e5)*(sin(e1)*sin(e4) + cos(e4)*(cos(e1)*cos(e2)*sin(e3) + cos(e1)*cos(e3)*sin(e2)))) - cos(e6)*(cos(e4)*sin(e1) - sin(e4)*(cos(e1)*cos(e2)*sin(e3) + cos(e1)*cos(e3)*sin(e2))))*(x6*(sin(e2 + e3)*cos(e5) + cos(e2 + e3)*cos(e4)*sin(e5)) - z6*(cos(e6)*(sin(e2 + e3)*sin(e5) - cos(e2 + e3)*cos(e4)*cos(e5)) + cos(e2 + e3)*sin(e4)*sin(e6)) + cos(e4)*cos(e6)*(a1 + d4*cos(e2 + e3) + a3*sin(e2 + e3) + a2*sin(e2)) - cos(e5)*sin(e4)*sin(e6)*(a1 + d4*cos(e2 + e3) + a3*sin(e2 + e3) + a2*sin(e2))) + (cos(e6)*(sin(e5)*(cos(e1)*cos(e2)*cos(e3) - cos(e1)*sin(e2)*sin(e3)) + cos(e5)*(sin(e1)*sin(e4) + cos(e4)*(cos(e1)*cos(e2)*sin(e3) + cos(e1)*cos(e3)*sin(e2)))) + sin(e6)*(cos(e4)*sin(e1) - sin(e4)*(cos(e1)*cos(e2)*sin(e3) + cos(e1)*cos(e3)*sin(e2))))*(y6*(sin(e2 + e3)*cos(e5) + cos(e2 + e3)*cos(e4)*sin(e5)) + z6*(sin(e6)*(sin(e2 + e3)*sin(e5) - cos(e2 + e3)*cos(e4)*cos(e5)) - cos(e2 + e3)*cos(e6)*sin(e4)) - cos(e4)*sin(e6)*(a1 + d4*cos(e2 + e3) + a3*sin(e2 + e3) + a2*sin(e2)) - cos(e5)*cos(e6)*sin(e4)*(a1 + d4*cos(e2 + e3) + a3*sin(e2 + e3) + a2*sin(e2))) - (cos(e5)*(cos(e1)*cos(e2)*cos(e3) - cos(e1)*sin(e2)*sin(e3)) - sin(e5)*(sin(e1)*sin(e4) + cos(e4)*(cos(e1)*cos(e2)*sin(e3) + cos(e1)*cos(e3)*sin(e2))))*(x6*(sin(e6)*(sin(e2 + e3)*sin(e5) - cos(e2 + e3)*cos(e4)*cos(e5)) - cos(e2 + e3)*cos(e6)*sin(e4)) + y6*(cos(e6)*(sin(e2 + e3)*sin(e5) - cos(e2 + e3)*cos(e4)*cos(e5)) + cos(e2 + e3)*sin(e4)*sin(e6)) - sin(e4)*sin(e5)*(a1 + d4*cos(e2 + e3) + a3*sin(e2 + e3) + a2*sin(e2))))*((sin(e6)*(sin(e5)*(cos(e1)*cos(e2)*cos(e3) - cos(e1)*sin(e2)*sin(e3)) + cos(e5)*(sin(e1)*sin(e4) + cos(e4)*(cos(e1)*cos(e2)*sin(e3) + cos(e1)*cos(e3)*sin(e2)))) - cos(e6)*(cos(e4)*sin(e1) - sin(e4)*(cos(e1)*cos(e2)*sin(e3) + cos(e1)*cos(e3)*sin(e2))))*(z6*(sin(e4)*sin(e6) - cos(e4)*cos(e5)*cos(e6)) - d4*cos(e4)*cos(e6) - x6*cos(e4)*sin(e5) + d4*cos(e5)*sin(e4)*sin(e6)) + (cos(e6)*(sin(e5)*(cos(e1)*cos(e2)*cos(e3) - cos(e1)*sin(e2)*sin(e3)) + cos(e5)*(sin(e1)*sin(e4) + cos(e4)*(cos(e1)*cos(e2)*sin(e3) + cos(e1)*cos(e3)*sin(e2)))) + sin(e6)*(cos(e4)*sin(e1) - sin(e4)*(cos(e1)*cos(e2)*sin(e3) + cos(e1)*cos(e3)*sin(e2))))*(z6*(cos(e6)*sin(e4) + cos(e4)*cos(e5)*sin(e6)) + d4*cos(e4)*sin(e6) - y6*cos(e4)*sin(e5) + d4*cos(e5)*cos(e6)*sin(e4)) - (cos(e5)*(cos(e1)*cos(e2)*cos(e3) - cos(e1)*sin(e2)*sin(e3)) - sin(e5)*(sin(e1)*sin(e4) + cos(e4)*(cos(e1)*cos(e2)*sin(e3) + cos(e1)*cos(e3)*sin(e2))))*(x6*(cos(e6)*sin(e4) + cos(e4)*cos(e5)*sin(e6)) - y6*(sin(e4)*sin(e6) - cos(e4)*cos(e5)*cos(e6)) + d4*sin(e4)*sin(e5)) - (cos(e6)*(sin(e1)*sin(e4) + cos(e4)*(cos(e1)*cos(e2)*sin(e3) + cos(e1)*cos(e3)*sin(e2))) + cos(e5)*sin(e6)*(cos(e4)*sin(e1) - sin(e4)*(cos(e1)*cos(e2)*sin(e3) + cos(e1)*cos(e3)*sin(e2))))*(z6*(cos(e4)*sin(e6) + cos(e5)*cos(e6)*sin(e4)) - sin(e6)*(a3*sin(e5) - d4*cos(e4)*cos(e5)) + d4*cos(e6)*sin(e4) + x6*sin(e4)*sin(e5)) + (sin(e6)*(sin(e1)*sin(e4) + cos(e4)*(cos(e1)*cos(e2)*sin(e3) + cos(e1)*cos(e3)*sin(e2))) - cos(e5)*cos(e6)*(cos(e4)*sin(e1) - sin(e4)*(cos(e1)*cos(e2)*sin(e3) + cos(e1)*cos(e3)*sin(e2))))*(z6*(cos(e4)*cos(e6) - cos(e5)*sin(e4)*sin(e6)) - cos(e6)*(a3*sin(e5) - d4*cos(e4)*cos(e5)) - d4*sin(e4)*sin(e6) + y6*sin(e4)*sin(e5)) - sin(e5)*(cos(e4)*sin(e1) - sin(e4)*(cos(e1)*cos(e2)*sin(e3) + cos(e1)*cos(e3)*sin(e2)))*(a3*cos(e5) - y6*(cos(e4)*sin(e6) + cos(e5)*cos(e6)*sin(e4)) + x6*(cos(e4)*cos(e6) - cos(e5)*sin(e4)*sin(e6)) + d4*cos(e4)*sin(e5))) - m5*((cos(e5)*(cos(e2)*sin(e3) + cos(e3)*sin(e2)) - cos(e4)*sin(e5)*(sin(e2)*sin(e3) - cos(e2)*cos(e3)))*(z5*(sin(e2 + e3)*sin(e5) - cos(e2 + e3)*cos(e4)*cos(e5)) + sin(e4)*sin(e5)*(a1 + d4*cos(e2 + e3) + a3*sin(e2 + e3) + a2*sin(e2)) + x5*cos(e2 + e3)*sin(e4)) - (sin(e5)*(cos(e2)*sin(e3) + cos(e3)*sin(e2)) + cos(e4)*cos(e5)*(sin(e2)*sin(e3) - cos(e2)*cos(e3)))*(z5*(sin(e2 + e3)*cos(e5) + cos(e2 + e3)*cos(e4)*sin(e5)) + cos(e5)*sin(e4)*(a1 + d4*cos(e2 + e3) + a3*sin(e2 + e3) + a2*sin(e2)) + y5*cos(e2 + e3)*sin(e4)) + sin(e4)*(sin(e2)*sin(e3) - cos(e2)*cos(e3))*(cos(e4)*(a1 + d4*cos(e2 + e3) + a3*sin(e2 + e3) + a2*sin(e2)) + x5*(sin(e2 + e3)*cos(e5) + cos(e2 + e3)*cos(e4)*sin(e5)) - y5*(sin(e2 + e3)*sin(e5) - cos(e2 + e3)*cos(e4)*cos(e5))))*((cos(e5)*(cos(e2)*sin(e3) + cos(e3)*sin(e2)) - cos(e4)*sin(e5)*(sin(e2)*sin(e3) - cos(e2)*cos(e3)))*(x5*sin(e4) - z5*cos(e4)*cos(e5) + d4*sin(e4)*sin(e5)) - (sin(e5)*(cos(e2)*sin(e3) + cos(e3)*sin(e2)) + cos(e4)*cos(e5)*(sin(e2)*sin(e3) - cos(e2)*cos(e3)))*(y5*sin(e4) + d4*cos(e5)*sin(e4) + z5*cos(e4)*sin(e5)) + sin(e4)*(sin(e2)*sin(e3) - cos(e2)*cos(e3))*(d4*cos(e4) + y5*cos(e4)*cos(e5) + x5*cos(e4)*sin(e5)) + cos(e4)*(sin(e2)*sin(e3) - cos(e2)*cos(e3))*(d4*sin(e4) + y5*cos(e5)*sin(e4) + x5*sin(e4)*sin(e5)) - sin(e4)*sin(e5)*(sin(e2)*sin(e3) - cos(e2)*cos(e3))*(a3*cos(e5) + x5*cos(e4) + d4*cos(e4)*sin(e5) + z5*cos(e5)*sin(e4)) + cos(e5)*sin(e4)*(sin(e2)*sin(e3) - cos(e2)*cos(e3))*(a3*sin(e5) - y5*cos(e4) - d4*cos(e4)*cos(e5) + z5*sin(e4)*sin(e5))) + m6*((sin(e6)*(sin(e5)*(cos(e2)*sin(e3) + cos(e3)*sin(e2)) + cos(e4)*cos(e5)*(sin(e2)*sin(e3) - cos(e2)*cos(e3))) + cos(e6)*sin(e4)*(sin(e2)*sin(e3) - cos(e2)*cos(e3)))*(z6*(cos(e4)*sin(e6) + cos(e5)*cos(e6)*sin(e4)) - sin(e6)*(a3*sin(e5) - d4*cos(e4)*cos(e5)) + d4*cos(e6)*sin(e4) + x6*sin(e4)*sin(e5)) + (cos(e6)*(sin(e5)*(cos(e2)*sin(e3) + cos(e3)*sin(e2)) + cos(e4)*cos(e5)*(sin(e2)*sin(e3) - cos(e2)*cos(e3))) - sin(e4)*sin(e6)*(sin(e2)*sin(e3) - cos(e2)*cos(e3)))*(z6*(cos(e4)*cos(e6) - cos(e5)*sin(e4)*sin(e6)) - cos(e6)*(a3*sin(e5) - d4*cos(e4)*cos(e5)) - d4*sin(e4)*sin(e6) + y6*sin(e4)*sin(e5)) - (cos(e5)*(cos(e2)*sin(e3) + cos(e3)*sin(e2)) - cos(e4)*sin(e5)*(sin(e2)*sin(e3) - cos(e2)*cos(e3)))*(a3*cos(e5) - y6*(cos(e4)*sin(e6) + cos(e5)*cos(e6)*sin(e4)) + x6*(cos(e4)*cos(e6) - cos(e5)*sin(e4)*sin(e6)) + d4*cos(e4)*sin(e5)))*((sin(e6)*(sin(e5)*(cos(e2)*sin(e3) + cos(e3)*sin(e2)) + cos(e4)*cos(e5)*(sin(e2)*sin(e3) - cos(e2)*cos(e3))) + cos(e6)*sin(e4)*(sin(e2)*sin(e3) - cos(e2)*cos(e3)))*(z6*(cos(e2 + e3)*cos(e4)*sin(e6) + cos(e2 + e3)*cos(e5)*cos(e6)*sin(e4)) + cos(e6)*sin(e4)*(a1 + d4*cos(e2 + e3) + a3*sin(e2 + e3) + a2*sin(e2)) + x6*cos(e2 + e3)*sin(e4)*sin(e5) + cos(e4)*cos(e5)*sin(e6)*(a1 + d4*cos(e2 + e3) + a3*sin(e2 + e3) + a2*sin(e2))) + (cos(e6)*(sin(e5)*(cos(e2)*sin(e3) + cos(e3)*sin(e2)) + cos(e4)*cos(e5)*(sin(e2)*sin(e3) - cos(e2)*cos(e3))) - sin(e4)*sin(e6)*(sin(e2)*sin(e3) - cos(e2)*cos(e3)))*(z6*(cos(e2 + e3)*cos(e4)*cos(e6) - cos(e2 + e3)*cos(e5)*sin(e4)*sin(e6)) - sin(e4)*sin(e6)*(a1 + d4*cos(e2 + e3) + a3*sin(e2 + e3) + a2*sin(e2)) + y6*cos(e2 + e3)*sin(e4)*sin(e5) + cos(e4)*cos(e5)*cos(e6)*(a1 + d4*cos(e2 + e3) + a3*sin(e2 + e3) + a2*sin(e2))) - (cos(e5)*(cos(e2)*sin(e3) + cos(e3)*sin(e2)) - cos(e4)*sin(e5)*(sin(e2)*sin(e3) - cos(e2)*cos(e3)))*(x6*(cos(e2 + e3)*cos(e4)*cos(e6) - cos(e2 + e3)*cos(e5)*sin(e4)*sin(e6)) - y6*(cos(e2 + e3)*cos(e4)*sin(e6) + cos(e2 + e3)*cos(e5)*cos(e6)*sin(e4)) + cos(e4)*sin(e5)*(a1 + d4*cos(e2 + e3) + a3*sin(e2 + e3) + a2*sin(e2))) - (cos(e4)*cos(e6)*(sin(e2)*sin(e3) - cos(e2)*cos(e3)) - cos(e5)*sin(e4)*sin(e6)*(sin(e2)*sin(e3) - cos(e2)*cos(e3)))*(x6*(sin(e2 + e3)*cos(e5) + cos(e2 + e3)*cos(e4)*sin(e5)) - z6*(cos(e6)*(sin(e2 + e3)*sin(e5) - cos(e2 + e3)*cos(e4)*cos(e5)) + cos(e2 + e3)*sin(e4)*sin(e6)) + cos(e4)*cos(e6)*(a1 + d4*cos(e2 + e3) + a3*sin(e2 + e3) + a2*sin(e2)) - cos(e5)*sin(e4)*sin(e6)*(a1 + d4*cos(e2 + e3) + a3*sin(e2 + e3) + a2*sin(e2))) + (cos(e4)*sin(e6)*(sin(e2)*sin(e3) - cos(e2)*cos(e3)) + cos(e5)*cos(e6)*sin(e4)*(sin(e2)*sin(e3) - cos(e2)*cos(e3)))*(y6*(sin(e2 + e3)*cos(e5) + cos(e2 + e3)*cos(e4)*sin(e5)) + z6*(sin(e6)*(sin(e2 + e3)*sin(e5) - cos(e2 + e3)*cos(e4)*cos(e5)) - cos(e2 + e3)*cos(e6)*sin(e4)) - cos(e4)*sin(e6)*(a1 + d4*cos(e2 + e3) + a3*sin(e2 + e3) + a2*sin(e2)) - cos(e5)*cos(e6)*sin(e4)*(a1 + d4*cos(e2 + e3) + a3*sin(e2 + e3) + a2*sin(e2))) + sin(e4)*sin(e5)*(sin(e2)*sin(e3) - cos(e2)*cos(e3))*(x6*(sin(e6)*(sin(e2 + e3)*sin(e5) - cos(e2 + e3)*cos(e4)*cos(e5)) - cos(e2 + e3)*cos(e6)*sin(e4)) + y6*(cos(e6)*(sin(e2 + e3)*sin(e5) - cos(e2 + e3)*cos(e4)*cos(e5)) + cos(e2 + e3)*sin(e4)*sin(e6)) - sin(e4)*sin(e5)*(a1 + d4*cos(e2 + e3) + a3*sin(e2 + e3) + a2*sin(e2)))) + m4*((cos(e2)*cos(e3)*sin(e1) - sin(e1)*sin(e2)*sin(e3))*(a3 + x4*cos(e4) - y4*sin(e4)) + (d4*cos(e4) + z4*cos(e4))*(cos(e1)*sin(e4) - cos(e4)*(cos(e2)*sin(e1)*sin(e3) + cos(e3)*sin(e1)*sin(e2))) - (sin(e4)*(cos(e2)*sin(e1)*sin(e3) + cos(e3)*sin(e1)*sin(e2)) + cos(e1)*cos(e4))*(d4*sin(e4) + z4*sin(e4)))*((cos(e2)*cos(e3)*sin(e1) - sin(e1)*sin(e2)*sin(e3))*(x4*cos(e2 + e3)*cos(e4) - y4*cos(e2 + e3)*sin(e4)) - (cos(e1)*sin(e4) - cos(e4)*(cos(e2)*sin(e1)*sin(e3) + cos(e3)*sin(e1)*sin(e2)))*(cos(e4)*(a1 + d4*cos(e2 + e3) + a3*sin(e2 + e3) + a2*sin(e2)) + x4*sin(e2 + e3) + z4*cos(e2 + e3)*cos(e4)) + (sin(e4)*(cos(e2)*sin(e1)*sin(e3) + cos(e3)*sin(e1)*sin(e2)) + cos(e1)*cos(e4))*(sin(e4)*(a1 + d4*cos(e2 + e3) + a3*sin(e2 + e3) + a2*sin(e2)) - y4*sin(e2 + e3) + z4*cos(e2 + e3)*sin(e4)) + (cos(e1)*sin(e4) - cos(e4)*(cos(e2)*sin(e1)*sin(e3) + cos(e3)*sin(e1)*sin(e2)))*(cos(e4)*(a1 + d4*cos(e2 + e3) + a3*sin(e2 + e3) + a2*sin(e2)) + z4*cos(e2 + e3)*cos(e4)) - (sin(e4)*(cos(e2)*sin(e1)*sin(e3) + cos(e3)*sin(e1)*sin(e2)) + cos(e1)*cos(e4))*(sin(e4)*(a1 + d4*cos(e2 + e3) + a3*sin(e2 + e3) + a2*sin(e2)) + z4*cos(e2 + e3)*sin(e4))) + m5*((cos(e5)*(cos(e2)*sin(e3) + cos(e3)*sin(e2)) - cos(e4)*sin(e5)*(sin(e2)*sin(e3) - cos(e2)*cos(e3)))*(a3*cos(e5) + x5*cos(e4) + d4*cos(e4)*sin(e5) + z5*cos(e5)*sin(e4)) + (sin(e5)*(cos(e2)*sin(e3) + cos(e3)*sin(e2)) + cos(e4)*cos(e5)*(sin(e2)*sin(e3) - cos(e2)*cos(e3)))*(a3*sin(e5) - y5*cos(e4) - d4*cos(e4)*cos(e5) + z5*sin(e4)*sin(e5)) - sin(e4)*(sin(e2)*sin(e3) - cos(e2)*cos(e3))*(d4*sin(e4) + y5*cos(e5)*sin(e4) + x5*sin(e4)*sin(e5)))*((cos(e5)*(cos(e2)*sin(e3) + cos(e3)*sin(e2)) - cos(e4)*sin(e5)*(sin(e2)*sin(e3) - cos(e2)*cos(e3)))*(cos(e4)*sin(e5)*(a1 + d4*cos(e2 + e3) + a3*sin(e2 + e3) + a2*sin(e2)) + x5*cos(e2 + e3)*cos(e4) + z5*cos(e2 + e3)*cos(e5)*sin(e4)) - (sin(e5)*(cos(e2)*sin(e3) + cos(e3)*sin(e2)) + cos(e4)*cos(e5)*(sin(e2)*sin(e3) - cos(e2)*cos(e3)))*(y5*cos(e2 + e3)*cos(e4) + cos(e4)*cos(e5)*(a1 + d4*cos(e2 + e3) + a3*sin(e2 + e3) + a2*sin(e2)) - z5*cos(e2 + e3)*sin(e4)*sin(e5)) + cos(e4)*(sin(e2)*sin(e3) - cos(e2)*cos(e3))*(cos(e4)*(a1 + d4*cos(e2 + e3) + a3*sin(e2 + e3) + a2*sin(e2)) + x5*(sin(e2 + e3)*cos(e5) + cos(e2 + e3)*cos(e4)*sin(e5)) - y5*(sin(e2 + e3)*sin(e5) - cos(e2 + e3)*cos(e4)*cos(e5))) - sin(e4)*(sin(e2)*sin(e3) - cos(e2)*cos(e3))*(sin(e4)*(a1 + d4*cos(e2 + e3) + a3*sin(e2 + e3) + a2*sin(e2)) + y5*cos(e2 + e3)*cos(e5)*sin(e4) + x5*cos(e2 + e3)*sin(e4)*sin(e5)) + cos(e5)*sin(e4)*(sin(e2)*sin(e3) - cos(e2)*cos(e3))*(z5*(sin(e2 + e3)*cos(e5) + cos(e2 + e3)*cos(e4)*sin(e5)) + cos(e5)*sin(e4)*(a1 + d4*cos(e2 + e3) + a3*sin(e2 + e3) + a2*sin(e2)) + y5*cos(e2 + e3)*sin(e4)) + sin(e4)*sin(e5)*(sin(e2)*sin(e3) - cos(e2)*cos(e3))*(z5*(sin(e2 + e3)*sin(e5) - cos(e2 + e3)*cos(e4)*cos(e5)) + sin(e4)*sin(e5)*(a1 + d4*cos(e2 + e3) + a3*sin(e2 + e3) + a2*sin(e2)) + x5*cos(e2 + e3)*sin(e4))) - m4*(cos(e4)*(sin(e2)*sin(e3) - cos(e2)*cos(e3))*(d4*cos(e4) + z4*cos(e4)) - (cos(e2)*sin(e3) + cos(e3)*sin(e2))*(a3 + x4*cos(e4) - y4*sin(e4)) + sin(e4)*(sin(e2)*sin(e3) - cos(e2)*cos(e3))*(d4*sin(e4) + z4*sin(e4)))*((cos(e2)*sin(e3) + cos(e3)*sin(e2))*(x4*cos(e2 + e3)*cos(e4) - y4*cos(e2 + e3)*sin(e4)) - cos(e4)*(sin(e2)*sin(e3) - cos(e2)*cos(e3))*(cos(e4)*(a1 + d4*cos(e2 + e3) + a3*sin(e2 + e3) + a2*sin(e2)) + z4*cos(e2 + e3)*cos(e4)) - sin(e4)*(sin(e2)*sin(e3) - cos(e2)*cos(e3))*(sin(e4)*(a1 + d4*cos(e2 + e3) + a3*sin(e2 + e3) + a2*sin(e2)) + z4*cos(e2 + e3)*sin(e4)) + cos(e4)*(sin(e2)*sin(e3) - cos(e2)*cos(e3))*(cos(e4)*(a1 + d4*cos(e2 + e3) + a3*sin(e2 + e3) + a2*sin(e2)) + x4*sin(e2 + e3) + z4*cos(e2 + e3)*cos(e4)) + sin(e4)*(sin(e2)*sin(e3) - cos(e2)*cos(e3))*(sin(e4)*(a1 + d4*cos(e2 + e3) + a3*sin(e2 + e3) + a2*sin(e2)) - y4*sin(e2 + e3) + z4*cos(e2 + e3)*sin(e4))) + m6*((sin(e6)*(sin(e5)*(cos(e2)*sin(e3) + cos(e3)*sin(e2)) + cos(e4)*cos(e5)*(sin(e2)*sin(e3) - cos(e2)*cos(e3))) + cos(e6)*sin(e4)*(sin(e2)*sin(e3) - cos(e2)*cos(e3)))*(x6*(sin(e2 + e3)*cos(e5) + cos(e2 + e3)*cos(e4)*sin(e5)) - z6*(cos(e6)*(sin(e2 + e3)*sin(e5) - cos(e2 + e3)*cos(e4)*cos(e5)) + cos(e2 + e3)*sin(e4)*sin(e6)) + cos(e4)*cos(e6)*(a1 + d4*cos(e2 + e3) + a3*sin(e2 + e3) + a2*sin(e2)) - cos(e5)*sin(e4)*sin(e6)*(a1 + d4*cos(e2 + e3) + a3*sin(e2 + e3) + a2*sin(e2))) + (cos(e6)*(sin(e5)*(cos(e2)*sin(e3) + cos(e3)*sin(e2)) + cos(e4)*cos(e5)*(sin(e2)*sin(e3) - cos(e2)*cos(e3))) - sin(e4)*sin(e6)*(sin(e2)*sin(e3) - cos(e2)*cos(e3)))*(y6*(sin(e2 + e3)*cos(e5) + cos(e2 + e3)*cos(e4)*sin(e5)) + z6*(sin(e6)*(sin(e2 + e3)*sin(e5) - cos(e2 + e3)*cos(e4)*cos(e5)) - cos(e2 + e3)*cos(e6)*sin(e4)) - cos(e4)*sin(e6)*(a1 + d4*cos(e2 + e3) + a3*sin(e2 + e3) + a2*sin(e2)) - cos(e5)*cos(e6)*sin(e4)*(a1 + d4*cos(e2 + e3) + a3*sin(e2 + e3) + a2*sin(e2))) - (cos(e5)*(cos(e2)*sin(e3) + cos(e3)*sin(e2)) - cos(e4)*sin(e5)*(sin(e2)*sin(e3) - cos(e2)*cos(e3)))*(x6*(sin(e6)*(sin(e2 + e3)*sin(e5) - cos(e2 + e3)*cos(e4)*cos(e5)) - cos(e2 + e3)*cos(e6)*sin(e4)) + y6*(cos(e6)*(sin(e2 + e3)*sin(e5) - cos(e2 + e3)*cos(e4)*cos(e5)) + cos(e2 + e3)*sin(e4)*sin(e6)) - sin(e4)*sin(e5)*(a1 + d4*cos(e2 + e3) + a3*sin(e2 + e3) + a2*sin(e2))))*((sin(e6)*(sin(e5)*(cos(e2)*sin(e3) + cos(e3)*sin(e2)) + cos(e4)*cos(e5)*(sin(e2)*sin(e3) - cos(e2)*cos(e3))) + cos(e6)*sin(e4)*(sin(e2)*sin(e3) - cos(e2)*cos(e3)))*(z6*(sin(e4)*sin(e6) - cos(e4)*cos(e5)*cos(e6)) - d4*cos(e4)*cos(e6) - x6*cos(e4)*sin(e5) + d4*cos(e5)*sin(e4)*sin(e6)) + (cos(e6)*(sin(e5)*(cos(e2)*sin(e3) + cos(e3)*sin(e2)) + cos(e4)*cos(e5)*(sin(e2)*sin(e3) - cos(e2)*cos(e3))) - sin(e4)*sin(e6)*(sin(e2)*sin(e3) - cos(e2)*cos(e3)))*(z6*(cos(e6)*sin(e4) + cos(e4)*cos(e5)*sin(e6)) + d4*cos(e4)*sin(e6) - y6*cos(e4)*sin(e5) + d4*cos(e5)*cos(e6)*sin(e4)) - (cos(e4)*cos(e6)*(sin(e2)*sin(e3) - cos(e2)*cos(e3)) - cos(e5)*sin(e4)*sin(e6)*(sin(e2)*sin(e3) - cos(e2)*cos(e3)))*(z6*(cos(e4)*sin(e6) + cos(e5)*cos(e6)*sin(e4)) - sin(e6)*(a3*sin(e5) - d4*cos(e4)*cos(e5)) + d4*cos(e6)*sin(e4) + x6*sin(e4)*sin(e5)) + (cos(e4)*sin(e6)*(sin(e2)*sin(e3) - cos(e2)*cos(e3)) + cos(e5)*cos(e6)*sin(e4)*(sin(e2)*sin(e3) - cos(e2)*cos(e3)))*(z6*(cos(e4)*cos(e6) - cos(e5)*sin(e4)*sin(e6)) - cos(e6)*(a3*sin(e5) - d4*cos(e4)*cos(e5)) - d4*sin(e4)*sin(e6) + y6*sin(e4)*sin(e5)) - (cos(e5)*(cos(e2)*sin(e3) + cos(e3)*sin(e2)) - cos(e4)*sin(e5)*(sin(e2)*sin(e3) - cos(e2)*cos(e3)))*(x6*(cos(e6)*sin(e4) + cos(e4)*cos(e5)*sin(e6)) - y6*(sin(e4)*sin(e6) - cos(e4)*cos(e5)*cos(e6)) + d4*sin(e4)*sin(e5)) + sin(e4)*sin(e5)*(sin(e2)*sin(e3) - cos(e2)*cos(e3))*(a3*cos(e5) - y6*(cos(e4)*sin(e6) + cos(e5)*cos(e6)*sin(e4)) + x6*(cos(e4)*cos(e6) - cos(e5)*sin(e4)*sin(e6)) + d4*cos(e4)*sin(e5))) + m6*((sin(e6)*(sin(e5)*(cos(e2)*cos(e3)*sin(e1) - sin(e1)*sin(e2)*sin(e3)) - cos(e5)*(cos(e1)*sin(e4) - cos(e4)*(cos(e2)*sin(e1)*sin(e3) + cos(e3)*sin(e1)*sin(e2)))) + cos(e6)*(sin(e4)*(cos(e2)*sin(e1)*sin(e3) + cos(e3)*sin(e1)*sin(e2)) + cos(e1)*cos(e4)))*(z6*(cos(e4)*sin(e6) + cos(e5)*cos(e6)*sin(e4)) - sin(e6)*(a3*sin(e5) - d4*cos(e4)*cos(e5)) + d4*cos(e6)*sin(e4) + x6*sin(e4)*sin(e5)) - (cos(e5)*(cos(e2)*cos(e3)*sin(e1) - sin(e1)*sin(e2)*sin(e3)) + sin(e5)*(cos(e1)*sin(e4) - cos(e4)*(cos(e2)*sin(e1)*sin(e3) + cos(e3)*sin(e1)*sin(e2))))*(a3*cos(e5) - y6*(cos(e4)*sin(e6) + cos(e5)*cos(e6)*sin(e4)) + x6*(cos(e4)*cos(e6) - cos(e5)*sin(e4)*sin(e6)) + d4*cos(e4)*sin(e5)) + (cos(e6)*(sin(e5)*(cos(e2)*cos(e3)*sin(e1) - sin(e1)*sin(e2)*sin(e3)) - cos(e5)*(cos(e1)*sin(e4) - cos(e4)*(cos(e2)*sin(e1)*sin(e3) + cos(e3)*sin(e1)*sin(e2)))) - sin(e6)*(sin(e4)*(cos(e2)*sin(e1)*sin(e3) + cos(e3)*sin(e1)*sin(e2)) + cos(e1)*cos(e4)))*(z6*(cos(e4)*cos(e6) - cos(e5)*sin(e4)*sin(e6)) - cos(e6)*(a3*sin(e5) - d4*cos(e4)*cos(e5)) - d4*sin(e4)*sin(e6) + y6*sin(e4)*sin(e5)))*((cos(e6)*(cos(e1)*sin(e4) - cos(e4)*(cos(e2)*sin(e1)*sin(e3) + cos(e3)*sin(e1)*sin(e2))) + cos(e5)*sin(e6)*(sin(e4)*(cos(e2)*sin(e1)*sin(e3) + cos(e3)*sin(e1)*sin(e2)) + cos(e1)*cos(e4)))*(x6*(sin(e2 + e3)*cos(e5) + cos(e2 + e3)*cos(e4)*sin(e5)) - z6*(cos(e6)*(sin(e2 + e3)*sin(e5) - cos(e2 + e3)*cos(e4)*cos(e5)) + cos(e2 + e3)*sin(e4)*sin(e6)) + cos(e4)*cos(e6)*(a1 + d4*cos(e2 + e3) + a3*sin(e2 + e3) + a2*sin(e2)) - cos(e5)*sin(e4)*sin(e6)*(a1 + d4*cos(e2 + e3) + a3*sin(e2 + e3) + a2*sin(e2))) - (cos(e5)*(cos(e2)*cos(e3)*sin(e1) - sin(e1)*sin(e2)*sin(e3)) + sin(e5)*(cos(e1)*sin(e4) - cos(e4)*(cos(e2)*sin(e1)*sin(e3) + cos(e3)*sin(e1)*sin(e2))))*(x6*(cos(e2 + e3)*cos(e4)*cos(e6) - cos(e2 + e3)*cos(e5)*sin(e4)*sin(e6)) - y6*(cos(e2 + e3)*cos(e4)*sin(e6) + cos(e2 + e3)*cos(e5)*cos(e6)*sin(e4)) + cos(e4)*sin(e5)*(a1 + d4*cos(e2 + e3) + a3*sin(e2 + e3) + a2*sin(e2))) + (sin(e6)*(sin(e5)*(cos(e2)*cos(e3)*sin(e1) - sin(e1)*sin(e2)*sin(e3)) - cos(e5)*(cos(e1)*sin(e4) - cos(e4)*(cos(e2)*sin(e1)*sin(e3) + cos(e3)*sin(e1)*sin(e2)))) + cos(e6)*(sin(e4)*(cos(e2)*sin(e1)*sin(e3) + cos(e3)*sin(e1)*sin(e2)) + cos(e1)*cos(e4)))*(z6*(cos(e2 + e3)*cos(e4)*sin(e6) + cos(e2 + e3)*cos(e5)*cos(e6)*sin(e4)) + cos(e6)*sin(e4)*(a1 + d4*cos(e2 + e3) + a3*sin(e2 + e3) + a2*sin(e2)) + x6*cos(e2 + e3)*sin(e4)*sin(e5) + cos(e4)*cos(e5)*sin(e6)*(a1 + d4*cos(e2 + e3) + a3*sin(e2 + e3) + a2*sin(e2))) - (sin(e6)*(cos(e1)*sin(e4) - cos(e4)*(cos(e2)*sin(e1)*sin(e3) + cos(e3)*sin(e1)*sin(e2))) - cos(e5)*cos(e6)*(sin(e4)*(cos(e2)*sin(e1)*sin(e3) + cos(e3)*sin(e1)*sin(e2)) + cos(e1)*cos(e4)))*(y6*(sin(e2 + e3)*cos(e5) + cos(e2 + e3)*cos(e4)*sin(e5)) + z6*(sin(e6)*(sin(e2 + e3)*sin(e5) - cos(e2 + e3)*cos(e4)*cos(e5)) - cos(e2 + e3)*cos(e6)*sin(e4)) - cos(e4)*sin(e6)*(a1 + d4*cos(e2 + e3) + a3*sin(e2 + e3) + a2*sin(e2)) - cos(e5)*cos(e6)*sin(e4)*(a1 + d4*cos(e2 + e3) + a3*sin(e2 + e3) + a2*sin(e2))) + (cos(e6)*(sin(e5)*(cos(e2)*cos(e3)*sin(e1) - sin(e1)*sin(e2)*sin(e3)) - cos(e5)*(cos(e1)*sin(e4) - cos(e4)*(cos(e2)*sin(e1)*sin(e3) + cos(e3)*sin(e1)*sin(e2)))) - sin(e6)*(sin(e4)*(cos(e2)*sin(e1)*sin(e3) + cos(e3)*sin(e1)*sin(e2)) + cos(e1)*cos(e4)))*(z6*(cos(e2 + e3)*cos(e4)*cos(e6) - cos(e2 + e3)*cos(e5)*sin(e4)*sin(e6)) - sin(e4)*sin(e6)*(a1 + d4*cos(e2 + e3) + a3*sin(e2 + e3) + a2*sin(e2)) + y6*cos(e2 + e3)*sin(e4)*sin(e5) + cos(e4)*cos(e5)*cos(e6)*(a1 + d4*cos(e2 + e3) + a3*sin(e2 + e3) + a2*sin(e2))) + sin(e5)*(sin(e4)*(cos(e2)*sin(e1)*sin(e3) + cos(e3)*sin(e1)*sin(e2)) + cos(e1)*cos(e4))*(x6*(sin(e6)*(sin(e2 + e3)*sin(e5) - cos(e2 + e3)*cos(e4)*cos(e5)) - cos(e2 + e3)*cos(e6)*sin(e4)) + y6*(cos(e6)*(sin(e2 + e3)*sin(e5) - cos(e2 + e3)*cos(e4)*cos(e5)) + cos(e2 + e3)*sin(e4)*sin(e6)) - sin(e4)*sin(e5)*(a1 + d4*cos(e2 + e3) + a3*sin(e2 + e3) + a2*sin(e2)))) + m5*((cos(e4)*sin(e1) - sin(e4)*(cos(e1)*cos(e2)*sin(e3) + cos(e1)*cos(e3)*sin(e2)))*(cos(e4)*(a1 + d4*cos(e2 + e3) + a3*sin(e2 + e3) + a2*sin(e2)) + x5*(sin(e2 + e3)*cos(e5) + cos(e2 + e3)*cos(e4)*sin(e5)) - y5*(sin(e2 + e3)*sin(e5) - cos(e2 + e3)*cos(e4)*cos(e5))) + (sin(e5)*(cos(e1)*cos(e2)*cos(e3) - cos(e1)*sin(e2)*sin(e3)) + cos(e5)*(sin(e1)*sin(e4) + cos(e4)*(cos(e1)*cos(e2)*sin(e3) + cos(e1)*cos(e3)*sin(e2))))*(z5*(sin(e2 + e3)*cos(e5) + cos(e2 + e3)*cos(e4)*sin(e5)) + cos(e5)*sin(e4)*(a1 + d4*cos(e2 + e3) + a3*sin(e2 + e3) + a2*sin(e2)) + y5*cos(e2 + e3)*sin(e4)) - (cos(e5)*(cos(e1)*cos(e2)*cos(e3) - cos(e1)*sin(e2)*sin(e3)) - sin(e5)*(sin(e1)*sin(e4) + cos(e4)*(cos(e1)*cos(e2)*sin(e3) + cos(e1)*cos(e3)*sin(e2))))*(z5*(sin(e2 + e3)*sin(e5) - cos(e2 + e3)*cos(e4)*cos(e5)) + sin(e4)*sin(e5)*(a1 + d4*cos(e2 + e3) + a3*sin(e2 + e3) + a2*sin(e2)) + x5*cos(e2 + e3)*sin(e4)))*((cos(e5)*(cos(e1)*cos(e2)*cos(e3) - cos(e1)*sin(e2)*sin(e3)) - sin(e5)*(sin(e1)*sin(e4) + cos(e4)*(cos(e1)*cos(e2)*sin(e3) + cos(e1)*cos(e3)*sin(e2))))*(x5*sin(e4) - z5*cos(e4)*cos(e5) + d4*sin(e4)*sin(e5)) - (sin(e5)*(cos(e1)*cos(e2)*cos(e3) - cos(e1)*sin(e2)*sin(e3)) + cos(e5)*(sin(e1)*sin(e4) + cos(e4)*(cos(e1)*cos(e2)*sin(e3) + cos(e1)*cos(e3)*sin(e2))))*(y5*sin(e4) + d4*cos(e5)*sin(e4) + z5*cos(e4)*sin(e5)) - (cos(e4)*sin(e1) - sin(e4)*(cos(e1)*cos(e2)*sin(e3) + cos(e1)*cos(e3)*sin(e2)))*(d4*cos(e4) + y5*cos(e4)*cos(e5) + x5*cos(e4)*sin(e5)) + (sin(e1)*sin(e4) + cos(e4)*(cos(e1)*cos(e2)*sin(e3) + cos(e1)*cos(e3)*sin(e2)))*(d4*sin(e4) + y5*cos(e5)*sin(e4) + x5*sin(e4)*sin(e5)) + sin(e5)*(cos(e4)*sin(e1) - sin(e4)*(cos(e1)*cos(e2)*sin(e3) + cos(e1)*cos(e3)*sin(e2)))*(a3*cos(e5) + x5*cos(e4) + d4*cos(e4)*sin(e5) + z5*cos(e5)*sin(e4)) - cos(e5)*(cos(e4)*sin(e1) - sin(e4)*(cos(e1)*cos(e2)*sin(e3) + cos(e1)*cos(e3)*sin(e2)))*(a3*sin(e5) - y5*cos(e4) - d4*cos(e4)*cos(e5) + z5*sin(e4)*sin(e5))) - m5*((cos(e5)*(cos(e2)*cos(e3)*sin(e1) - sin(e1)*sin(e2)*sin(e3)) + sin(e5)*(cos(e1)*sin(e4) - cos(e4)*(cos(e2)*sin(e1)*sin(e3) + cos(e3)*sin(e1)*sin(e2))))*(z5*(sin(e2 + e3)*sin(e5) - cos(e2 + e3)*cos(e4)*cos(e5)) + sin(e4)*sin(e5)*(a1 + d4*cos(e2 + e3) + a3*sin(e2 + e3) + a2*sin(e2)) + x5*cos(e2 + e3)*sin(e4)) + (sin(e4)*(cos(e2)*sin(e1)*sin(e3) + cos(e3)*sin(e1)*sin(e2)) + cos(e1)*cos(e4))*(cos(e4)*(a1 + d4*cos(e2 + e3) + a3*sin(e2 + e3) + a2*sin(e2)) + x5*(sin(e2 + e3)*cos(e5) + cos(e2 + e3)*cos(e4)*sin(e5)) - y5*(sin(e2 + e3)*sin(e5) - cos(e2 + e3)*cos(e4)*cos(e5))) - (sin(e5)*(cos(e2)*cos(e3)*sin(e1) - sin(e1)*sin(e2)*sin(e3)) - cos(e5)*(cos(e1)*sin(e4) - cos(e4)*(cos(e2)*sin(e1)*sin(e3) + cos(e3)*sin(e1)*sin(e2))))*(z5*(sin(e2 + e3)*cos(e5) + cos(e2 + e3)*cos(e4)*sin(e5)) + cos(e5)*sin(e4)*(a1 + d4*cos(e2 + e3) + a3*sin(e2 + e3) + a2*sin(e2)) + y5*cos(e2 + e3)*sin(e4)))*((cos(e5)*(cos(e2)*cos(e3)*sin(e1) - sin(e1)*sin(e2)*sin(e3)) + sin(e5)*(cos(e1)*sin(e4) - cos(e4)*(cos(e2)*sin(e1)*sin(e3) + cos(e3)*sin(e1)*sin(e2))))*(x5*sin(e4) - z5*cos(e4)*cos(e5) + d4*sin(e4)*sin(e5)) - (sin(e5)*(cos(e2)*cos(e3)*sin(e1) - sin(e1)*sin(e2)*sin(e3)) - cos(e5)*(cos(e1)*sin(e4) - cos(e4)*(cos(e2)*sin(e1)*sin(e3) + cos(e3)*sin(e1)*sin(e2))))*(y5*sin(e4) + d4*cos(e5)*sin(e4) + z5*cos(e4)*sin(e5)) + (sin(e4)*(cos(e2)*sin(e1)*sin(e3) + cos(e3)*sin(e1)*sin(e2)) + cos(e1)*cos(e4))*(d4*cos(e4) + y5*cos(e4)*cos(e5) + x5*cos(e4)*sin(e5)) - (cos(e1)*sin(e4) - cos(e4)*(cos(e2)*sin(e1)*sin(e3) + cos(e3)*sin(e1)*sin(e2)))*(d4*sin(e4) + y5*cos(e5)*sin(e4) + x5*sin(e4)*sin(e5)) - sin(e5)*(sin(e4)*(cos(e2)*sin(e1)*sin(e3) + cos(e3)*sin(e1)*sin(e2)) + cos(e1)*cos(e4))*(a3*cos(e5) + x5*cos(e4) + d4*cos(e4)*sin(e5) + z5*cos(e5)*sin(e4)) + cos(e5)*(sin(e4)*(cos(e2)*sin(e1)*sin(e3) + cos(e3)*sin(e1)*sin(e2)) + cos(e1)*cos(e4))*(a3*sin(e5) - y5*cos(e4) - d4*cos(e4)*cos(e5) + z5*sin(e4)*sin(e5))) - (cos(e4)*sin(e5)*(I6zz*(sin(e2 + e3)*cos(e5) + cos(e2 + e3)*cos(e4)*sin(e5)) + I6xz*(cos(e6)*(sin(e2 + e3)*sin(e5) - cos(e2 + e3)*cos(e4)*cos(e5)) + cos(e2 + e3)*sin(e4)*sin(e6)) - I6yz*(sin(e6)*(sin(e2 + e3)*sin(e5) - cos(e2 + e3)*cos(e4)*cos(e5)) - cos(e2 + e3)*cos(e6)*sin(e4))))/2 + m4*((cos(e1)*cos(e2)*cos(e3) - cos(e1)*sin(e2)*sin(e3))*(a3 + x4*cos(e4) - y4*sin(e4)) - (sin(e1)*sin(e4) + cos(e4)*(cos(e1)*cos(e2)*sin(e3) + cos(e1)*cos(e3)*sin(e2)))*(d4*cos(e4) + z4*cos(e4)) + (cos(e4)*sin(e1) - sin(e4)*(cos(e1)*cos(e2)*sin(e3) + cos(e1)*cos(e3)*sin(e2)))*(d4*sin(e4) + z4*sin(e4)))*((sin(e1)*sin(e4) + cos(e4)*(cos(e1)*cos(e2)*sin(e3) + cos(e1)*cos(e3)*sin(e2)))*(cos(e4)*(a1 + d4*cos(e2 + e3) + a3*sin(e2 + e3) + a2*sin(e2)) + x4*sin(e2 + e3) + z4*cos(e2 + e3)*cos(e4)) + (x4*cos(e2 + e3)*cos(e4) - y4*cos(e2 + e3)*sin(e4))*(cos(e1)*cos(e2)*cos(e3) - cos(e1)*sin(e2)*sin(e3)) - (cos(e4)*sin(e1) - sin(e4)*(cos(e1)*cos(e2)*sin(e3) + cos(e1)*cos(e3)*sin(e2)))*(sin(e4)*(a1 + d4*cos(e2 + e3) + a3*sin(e2 + e3) + a2*sin(e2)) - y4*sin(e2 + e3) + z4*cos(e2 + e3)*sin(e4)) - (sin(e1)*sin(e4) + cos(e4)*(cos(e1)*cos(e2)*sin(e3) + cos(e1)*cos(e3)*sin(e2)))*(cos(e4)*(a1 + d4*cos(e2 + e3) + a3*sin(e2 + e3) + a2*sin(e2)) + z4*cos(e2 + e3)*cos(e4)) + (cos(e4)*sin(e1) - sin(e4)*(cos(e1)*cos(e2)*sin(e3) + cos(e1)*cos(e3)*sin(e2)))*(sin(e4)*(a1 + d4*cos(e2 + e3) + a3*sin(e2 + e3) + a2*sin(e2)) + z4*cos(e2 + e3)*sin(e4))) + m6*((sin(e6)*(sin(e5)*(cos(e2)*cos(e3)*sin(e1) - sin(e1)*sin(e2)*sin(e3)) - cos(e5)*(cos(e1)*sin(e4) - cos(e4)*(cos(e2)*sin(e1)*sin(e3) + cos(e3)*sin(e1)*sin(e2)))) + cos(e6)*(sin(e4)*(cos(e2)*sin(e1)*sin(e3) + cos(e3)*sin(e1)*sin(e2)) + cos(e1)*cos(e4)))*(x6*(sin(e2 + e3)*cos(e5) + cos(e2 + e3)*cos(e4)*sin(e5)) - z6*(cos(e6)*(sin(e2 + e3)*sin(e5) - cos(e2 + e3)*cos(e4)*cos(e5)) + cos(e2 + e3)*sin(e4)*sin(e6)) + cos(e4)*cos(e6)*(a1 + d4*cos(e2 + e3) + a3*sin(e2 + e3) + a2*sin(e2)) - cos(e5)*sin(e4)*sin(e6)*(a1 + d4*cos(e2 + e3) + a3*sin(e2 + e3) + a2*sin(e2))) + (cos(e6)*(sin(e5)*(cos(e2)*cos(e3)*sin(e1) - sin(e1)*sin(e2)*sin(e3)) - cos(e5)*(cos(e1)*sin(e4) - cos(e4)*(cos(e2)*sin(e1)*sin(e3) + cos(e3)*sin(e1)*sin(e2)))) - sin(e6)*(sin(e4)*(cos(e2)*sin(e1)*sin(e3) + cos(e3)*sin(e1)*sin(e2)) + cos(e1)*cos(e4)))*(y6*(sin(e2 + e3)*cos(e5) + cos(e2 + e3)*cos(e4)*sin(e5)) + z6*(sin(e6)*(sin(e2 + e3)*sin(e5) - cos(e2 + e3)*cos(e4)*cos(e5)) - cos(e2 + e3)*cos(e6)*sin(e4)) - cos(e4)*sin(e6)*(a1 + d4*cos(e2 + e3) + a3*sin(e2 + e3) + a2*sin(e2)) - cos(e5)*cos(e6)*sin(e4)*(a1 + d4*cos(e2 + e3) + a3*sin(e2 + e3) + a2*sin(e2))) - (cos(e5)*(cos(e2)*cos(e3)*sin(e1) - sin(e1)*sin(e2)*sin(e3)) + sin(e5)*(cos(e1)*sin(e4) - cos(e4)*(cos(e2)*sin(e1)*sin(e3) + cos(e3)*sin(e1)*sin(e2))))*(x6*(sin(e6)*(sin(e2 + e3)*sin(e5) - cos(e2 + e3)*cos(e4)*cos(e5)) - cos(e2 + e3)*cos(e6)*sin(e4)) + y6*(cos(e6)*(sin(e2 + e3)*sin(e5) - cos(e2 + e3)*cos(e4)*cos(e5)) + cos(e2 + e3)*sin(e4)*sin(e6)) - sin(e4)*sin(e5)*(a1 + d4*cos(e2 + e3) + a3*sin(e2 + e3) + a2*sin(e2))))*((sin(e6)*(sin(e5)*(cos(e2)*cos(e3)*sin(e1) - sin(e1)*sin(e2)*sin(e3)) - cos(e5)*(cos(e1)*sin(e4) - cos(e4)*(cos(e2)*sin(e1)*sin(e3) + cos(e3)*sin(e1)*sin(e2)))) + cos(e6)*(sin(e4)*(cos(e2)*sin(e1)*sin(e3) + cos(e3)*sin(e1)*sin(e2)) + cos(e1)*cos(e4)))*(z6*(sin(e4)*sin(e6) - cos(e4)*cos(e5)*cos(e6)) - d4*cos(e4)*cos(e6) - x6*cos(e4)*sin(e5) + d4*cos(e5)*sin(e4)*sin(e6)) + (cos(e6)*(sin(e5)*(cos(e2)*cos(e3)*sin(e1) - sin(e1)*sin(e2)*sin(e3)) - cos(e5)*(cos(e1)*sin(e4) - cos(e4)*(cos(e2)*sin(e1)*sin(e3) + cos(e3)*sin(e1)*sin(e2)))) - sin(e6)*(sin(e4)*(cos(e2)*sin(e1)*sin(e3) + cos(e3)*sin(e1)*sin(e2)) + cos(e1)*cos(e4)))*(z6*(cos(e6)*sin(e4) + cos(e4)*cos(e5)*sin(e6)) + d4*cos(e4)*sin(e6) - y6*cos(e4)*sin(e5) + d4*cos(e5)*cos(e6)*sin(e4)) - (cos(e5)*(cos(e2)*cos(e3)*sin(e1) - sin(e1)*sin(e2)*sin(e3)) + sin(e5)*(cos(e1)*sin(e4) - cos(e4)*(cos(e2)*sin(e1)*sin(e3) + cos(e3)*sin(e1)*sin(e2))))*(x6*(cos(e6)*sin(e4) + cos(e4)*cos(e5)*sin(e6)) - y6*(sin(e4)*sin(e6) - cos(e4)*cos(e5)*cos(e6)) + d4*sin(e4)*sin(e5)) + (cos(e6)*(cos(e1)*sin(e4) - cos(e4)*(cos(e2)*sin(e1)*sin(e3) + cos(e3)*sin(e1)*sin(e2))) + cos(e5)*sin(e6)*(sin(e4)*(cos(e2)*sin(e1)*sin(e3) + cos(e3)*sin(e1)*sin(e2)) + cos(e1)*cos(e4)))*(z6*(cos(e4)*sin(e6) + cos(e5)*cos(e6)*sin(e4)) - sin(e6)*(a3*sin(e5) - d4*cos(e4)*cos(e5)) + d4*cos(e6)*sin(e4) + x6*sin(e4)*sin(e5)) - (sin(e6)*(cos(e1)*sin(e4) - cos(e4)*(cos(e2)*sin(e1)*sin(e3) + cos(e3)*sin(e1)*sin(e2))) - cos(e5)*cos(e6)*(sin(e4)*(cos(e2)*sin(e1)*sin(e3) + cos(e3)*sin(e1)*sin(e2)) + cos(e1)*cos(e4)))*(z6*(cos(e4)*cos(e6) - cos(e5)*sin(e4)*sin(e6)) - cos(e6)*(a3*sin(e5) - d4*cos(e4)*cos(e5)) - d4*sin(e4)*sin(e6) + y6*sin(e4)*sin(e5)) + sin(e5)*(sin(e4)*(cos(e2)*sin(e1)*sin(e3) + cos(e3)*sin(e1)*sin(e2)) + cos(e1)*cos(e4))*(a3*cos(e5) - y6*(cos(e4)*sin(e6) + cos(e5)*cos(e6)*sin(e4)) + x6*(cos(e4)*cos(e6) - cos(e5)*sin(e4)*sin(e6)) + d4*cos(e4)*sin(e5))) + m5*((sin(e5)*(cos(e1)*cos(e2)*cos(e3) - cos(e1)*sin(e2)*sin(e3)) + cos(e5)*(sin(e1)*sin(e4) + cos(e4)*(cos(e1)*cos(e2)*sin(e3) + cos(e1)*cos(e3)*sin(e2))))*(a3*sin(e5) - y5*cos(e4) - d4*cos(e4)*cos(e5) + z5*sin(e4)*sin(e5)) + (cos(e4)*sin(e1) - sin(e4)*(cos(e1)*cos(e2)*sin(e3) + cos(e1)*cos(e3)*sin(e2)))*(d4*sin(e4) + y5*cos(e5)*sin(e4) + x5*sin(e4)*sin(e5)) + (cos(e5)*(cos(e1)*cos(e2)*cos(e3) - cos(e1)*sin(e2)*sin(e3)) - sin(e5)*(sin(e1)*sin(e4) + cos(e4)*(cos(e1)*cos(e2)*sin(e3) + cos(e1)*cos(e3)*sin(e2))))*(a3*cos(e5) + x5*cos(e4) + d4*cos(e4)*sin(e5) + z5*cos(e5)*sin(e4)))*((cos(e5)*(cos(e1)*cos(e2)*cos(e3) - cos(e1)*sin(e2)*sin(e3)) - sin(e5)*(sin(e1)*sin(e4) + cos(e4)*(cos(e1)*cos(e2)*sin(e3) + 